simulink model "ABB_1010"  (R2024a)
settings: Solver=VariableStepAuto  StartTime=0.0  StopTime=200  RelTol=1e-3
model workspace: external: MATLAB File C:\Users\lucas\OneDrive\Documents\MATLAB\projeto final\ABB_1010_DataFile.m (data not in the file)
values from neighbouring files (symbols this model uses):
  g = 9.81    [inicializacaoAntropomorfico.m]
  I1 = [ 0.00243841  0.00000307  0.00007261    [inicializacaoAntropomorfico.m]
  I2 = [ 0.01633569  0.00000387 -0.00034405    [inicializacaoAntropomorfico.m]
  I3 = [ 0.00244760 -0.00000208  0.00000538    [inicializacaoAntropomorfico.m]
  I4 = [ 0.00245792 -0.00000008  0.00003121    [inicializacaoAntropomorfico.m]
  I5 = [ 0.00062165 -0.00000206 -0.00000303    [inicializacaoAntropomorfico.m]
  I6 = [ 0.00000357  0.00000000  0.00000000    [inicializacaoAntropomorfico.m]
  I7 = [(m7*L7^2)/12 0.00000000  0.00000000    [inicializacaoAntropomorfico.m]
  L = [L1, L2, L3, L4, L5, L6, L7]    [inicializacaoAntropomorfico.m]
  Lcm1 = [-0.00258308  0.00024508 -0.01434968]    [inicializacaoAntropomorfico.m]
  Lcm2 = [-0.02078894  0.00020016 -0.10516734]    [inicializacaoAntropomorfico.m]
  Lcm3 = [ 0.00021912  0.00015355 -0.06228290]    [inicializacaoAntropomorfico.m]
  Lcm4 = [-0.00172658 -0.00124140 -0.07369196]    [inicializacaoAntropomorfico.m]
  Lcm5 = [-0.00014110  0.00085992 -0.03825278]    [inicializacaoAntropomorfico.m]
  Lcm6 = [ 0.00002478  0.00000000 -0.00042157]    [inicializacaoAntropomorfico.m]
  Lcm7 = [ 0           0          -0.05000000]    [inicializacaoAntropomorfico.m]
  m = [m1, m2, m3, m4, m5, m6, m7]    [inicializacaoAntropomorfico.m]
  Pf = [  0.05    [inicializacaoAntropomorfico.m]
  Pi = [  0.2    [inicializacaoAntropomorfico.m]
  Raio = [0]    [inicializacaoAntropomorfico.m]
  Sentido = [0]    [inicializacaoAntropomorfico.m]
  Tipo = [1]    [inicializacaoAntropomorfico.m]
undefined symbols (not defined in the file or in its folder): smiData, X, Y, Z
libraries: sm_lib x35, nesl_utility x7
(part 14 of 16)

== matlab function ABB_1010/Dinamica1/MATLAB Function3 ==
  data: L parameter; Lcm1 parameter; Q input; I2 parameter; I3 parameter; I4 parameter; I5 parameter; I6 parameter; I7 parameter; Lcm2 parameter; Lcm3 parameter; Lcm4 parameter; Lcm5 parameter; Lcm6 parameter; m parameter; dQ input; C output; Lcm7 parameter; I1 parameter
function C = func_C( L, Lcm1, Q, I2, I3, I4, I5, I6, I7, Lcm2, Lcm3, Lcm4, Lcm5, Lcm6, m, dQ, Lcm7, I1)
%func_C
%    OUT1 = func_C(Ixx2,Ixx3,Ixx4,Ixx5,Ixx6,Ixy3,Ixy4,Ixy5,Ixy6,Ixz2,Ixz3,Ixz4,Ixz5,Ixz6,Iyx3,Iyx4,Iyx5,Iyx6,Iyy4,Iyy5,Iyy6,Iyz3,Iyz4,Iyz5,Iyz6,Izx2,Izx3,Izx4,Izx5,Izx6,Izy3,Izy4,Izy5,Izy6,Izz2,Izz3,Izz4,Izz5,Izz6,Lx2,Lx3,Lxcm2,Lxcm3,Lxcm4,Lxcm5,Lxcm6,Lycm3,Lycm4,Lycm5,Lycm6,Lz4,Lz5,Lzcm2,Lzcm3,Lzcm4,Lzcm5,Lzcm6,Q2,Q3,Q4,Q5,Q6,dQ1,dQ2,dQ3,dQ4,dQ5,dQ6,M2,M3,M4,M5,M6)

%    This function was generated by the Symbolic Math Toolbox version 24.1.
%    30-Apr-2025 06:24:11

C   = zeros(6,1);
m1  = m(1);
m2  = m(2);
m3  = m(3);
m4  = m(4);
m5  = m(5);
m6  = m(6);
m7  = m(7);

Q1  = Q(1);
Q2  = Q(2);
Q3  = Q(3);
Q4  = Q(4);
Q5  = Q(5);
Q6  = Q(6);

dQ1  = dQ(1);
dQ2  = dQ(2);
dQ3  = dQ(3);
dQ4  = dQ(4);
dQ5  = dQ(5);
dQ6  = dQ(6);

Lz1 = L(1);
Lx2 = L(2);
Lx3 = L(3);
Lx4 = L(4);
Lz5 = L(5);
Lz6 = L(6);
Lz7 = L(7);

Lxcm1 = Lcm1(1);
Lycm1 = Lcm1(2);
Lzcm1 = Lcm1(3);

Lxcm2 = Lcm2(1);
Lycm2 = Lcm2(2);
Lzcm2 = Lcm2(3);

Lxcm3 = Lcm3(1);
Lycm3 = Lcm3(2);
Lzcm3 = Lcm3(3);

Lxcm4 = Lcm4(1);
Lycm4 = Lcm4(2);
Lzcm4 = Lcm4(3);

Lxcm5 = Lcm5(1);
Lycm5 = Lcm5(2);
Lzcm5 = Lcm5(3);

Lxcm6 = Lcm6(1);
Lycm6 = Lcm6(2);
Lzcm6 = Lcm6(3);

Lxcm7 = Lcm7(1);
Lycm7 = Lcm7(2);
Lzcm7 = Lcm7(3);

Ixx1 = I1(1,1);
Ixy1 = I1(1,2);
Ixz1 = I1(1,3);
Iyx1 = I1(2,1);
Iyy1 = I1(2,2);
Iyz1 = I1(2,3);
Izx1 = I1(3,1);
Izy1 = I1(3,2);
Izz1 = I1(3,3);

Ixx2 = I2(1,1);
Ixy2 = I2(1,2);
Ixz2 = I2(1,3);
Iyx2 = I2(2,1);
Iyy2 = I2(2,2);
Iyz2 = I2(2,3);
Izx2 = I2(3,1);
Izy2 = I2(3,2);
Izz2 = I2(3,3);

Ixx3 = I3(1,1);
Ixy3 = I3(1,2);
Ixz3 = I3(1,3);
Iyx3 = I3(2,1);
Iyy3 = I3(2,2);
Iyz3 = I3(2,3);
Izx3 = I3(3,1);
Izy3 = I3(3,2);
Izz3 = I3(3,3);

Ixx4 = I4(1,1);
Ixy4 = I4(1,2);
Ixz4 = I4(1,3);
Iyx4 = I4(2,1);
Iyy4 = I4(2,2);
Iyz4 = I4(2,3);
Izx4 = I4(3,1);
Izy4 = I4(3,2);
Izz4 = I4(3,3);

Ixx5 = I5(1,1);
Ixy5 = I5(1,2);
Ixz5 = I5(1,3);
Iyx5 = I5(2,1);
Iyy5 = I5(2,2);
Iyz5 = I5(2,3);
Izx5 = I5(3,1);
Izy5 = I5(3,2);
Izz5 = I5(3,3);

Ixx6 = I6(1,1);
Ixy6 = I6(1,2);
Ixz6 = I6(1,3);
Iyx6 = I6(2,1);
Iyy6 = I6(2,2);
Iyz6 = I6(2,3);
Izx6 = I6(3,1);
Izy6 = I6(3,2);
Izz6 = I6(3,3);

Ixx7 = I7(1,1);
Ixy7 = I7(1,2);
Ixz7 = I7(1,3);
Iyx7 = I7(2,1);
Iyy7 = I7(2,2);
Iyz7 = I7(2,3);
Izx7 = I7(3,1);
Izy7 = I7(3,2);
Izz7 = I7(3,3);

t2 = cos(Q2);
t3 = cos(Q3);
t4 = cos(Q4);
t5 = cos(Q5);
t6 = cos(Q6);
t7 = sin(Q2);
t8 = sin(Q3);
t9 = sin(Q4);
t10 = sin(Q5);
t11 = sin(Q6);
t12 = Lx2^2;
t13 = Lx3^2;
t14 = Lx4^2;
t15 = Lxcm3^2;
t16 = Lxcm4^2;
t17 = Lxcm5^2;
t18 = Lxcm6^2;
t19 = Lycm4^2;
t20 = Lycm5^2;
t21 = Lycm6^2;
t22 = Lz6^2;
t23 = Lzcm3^2;
t24 = Lzcm4^2;
t25 = Lzcm5^2;
t26 = Lzcm6^2;
t27 = Q2*2.0;
t28 = Q3*2.0;
t29 = Q4*2.0;
t30 = Q5*2.0;
t31 = Q6*2.0;
t48 = Lx4*Lycm4*dQ2*dQ4*m4*2.0;
t49 = Lx4*Lycm4*dQ3*dQ4*m4*2.0;
t50 = Lx4*Lycm5*dQ2*dQ4*m5*2.0;
t51 = Lx4*Lycm5*dQ3*dQ4*m5*2.0;
t52 = Lxcm4*Lycm4*dQ2*dQ4*m4*2.0;
t53 = Lxcm4*Lycm4*dQ3*dQ4*m4*2.0;
t54 = Lxcm5*Lzcm5*dQ2*dQ5*m5*2.0;
t55 = Lxcm5*Lzcm5*dQ3*dQ5*m5*2.0;
t32 = t2^2;
t33 = t3^2;
t34 = t4^2;
t35 = t5^2;
t36 = t6^2;
t37 = sin(t27);
t38 = sin(t28);
t39 = sin(t29);
t40 = sin(t30);
t41 = sin(t31);
t42 = Ixx5*dQ4*dQ5*t9;
t43 = Ixx6*dQ4*dQ5*t9;
t44 = Iyy5*dQ4*dQ5*t9;
t45 = Iyy6*dQ4*dQ5*t9;
t46 = Izz5*dQ4*dQ5*t9;
t47 = Izz6*dQ4*dQ5*t9;
t80 = Ixx4*dQ1*dQ4*t2*t8;
t81 = Ixx4*dQ1*dQ4*t3*t7;
t82 = Ixx5*dQ1*dQ4*t2*t8;
t83 = Ixx5*dQ1*dQ4*t3*t7;
t84 = Ixx6*dQ1*dQ4*t2*t8;
t85 = Ixx6*dQ1*dQ4*t3*t7;
t86 = Ixx6*dQ4*dQ6*t4*t10;
t87 = Ixx6*dQ5*dQ6*t5*t9;
t88 = Iyy4*dQ1*dQ4*t2*t8;
t89 = Iyy4*dQ1*dQ4*t3*t7;
t90 = Iyy5*dQ1*dQ4*t2*t8;
t91 = Iyy5*dQ1*dQ4*t3*t7;
t92 = Iyy6*dQ1*dQ4*t2*t8;
t93 = Iyy6*dQ1*dQ4*t3*t7;
t94 = Iyy6*dQ4*dQ6*t4*t10;
t95 = Iyy6*dQ5*dQ6*t5*t9;
t96 = Izz4*dQ1*dQ4*t2*t8;
t97 = Izz4*dQ1*dQ4*t3*t7;
t98 = Izz5*dQ1*dQ4*t2*t8;
t99 = Izz5*dQ1*dQ4*t3*t7;
t100 = Izz6*dQ1*dQ4*t2*t8;
t101 = Izz6*dQ1*dQ4*t3*t7;
t102 = Izz6*dQ4*dQ6*t4*t10;
t103 = Izz6*dQ5*dQ6*t5*t9;
t104 = Lx3*Lycm4*dQ2*dQ4*m4*t4*2.0;
t105 = Lx3*Lycm4*dQ3*dQ4*m4*t4*2.0;
t106 = Lx3*Lycm5*dQ2*dQ4*m5*t4*2.0;
t107 = Lx3*Lycm5*dQ3*dQ4*m5*t4*2.0;
t108 = Lx4*Lycm6*dQ2*dQ4*m6*t6*2.0;
t109 = Lx4*Lycm6*dQ3*dQ4*m6*t6*2.0;
t110 = Lxcm5*Lycm5*dQ2*dQ4*m5*t5*2.0;
t111 = Lxcm5*Lycm5*dQ3*dQ4*m5*t5*2.0;
t112 = Lxcm6*Lycm6*dQ2*dQ4*m6*t5*2.0;
t113 = Lxcm6*Lycm6*dQ3*dQ4*m6*t5*2.0;
t114 = Lxcm6*Lycm6*dQ5*dQ6*m6*t4*2.0;
t115 = Lxcm6*Lz6*dQ2*dQ5*m6*t6*2.0;
t116 = Lxcm6*Lz6*dQ3*dQ5*m6*t6*2.0;
t117 = Lxcm6*Lzcm6*dQ2*dQ5*m6*t6*2.0;
t118 = Lxcm6*Lzcm6*dQ3*dQ5*m6*t6*2.0;
t119 = Lx3*Lx4*dQ2*dQ4*m4*t9*2.0;
t120 = Lx3*Lx4*dQ2*dQ4*m5*t9*2.0;
t121 = Lx3*Lx4*dQ3*dQ4*m4*t9*2.0;
t122 = Lx3*Lx4*dQ2*dQ4*m6*t9*2.0;
t123 = Lx3*Lx4*dQ3*dQ4*m5*t9*2.0;
t124 = Lx3*Lx4*dQ3*dQ4*m6*t9*2.0;
t125 = Lx3*Lxcm4*dQ2*dQ4*m4*t9*2.0;
t126 = Lx3*Lxcm4*dQ3*dQ4*m4*t9*2.0;
t127 = Lx4*Lxcm6*dQ2*dQ4*m6*t11*2.0;
t128 = Lx4*Lxcm6*dQ3*dQ4*m6*t11*2.0;
t129 = Lycm6*Lz6*dQ2*dQ5*m6*t11*2.0;
t130 = Lycm6*Lz6*dQ3*dQ5*m6*t11*2.0;
t131 = Lycm5*Lzcm5*dQ2*dQ4*m5*t10*2.0;
t132 = Lycm5*Lzcm5*dQ3*dQ4*m5*t10*2.0;
t133 = Lycm6*Lzcm6*dQ2*dQ5*m6*t11*2.0;
t134 = Lycm6*Lzcm6*dQ3*dQ5*m6*t11*2.0;
t135 = dQ4*dQ5*m5*t9*t17*2.0;
t136 = dQ4*dQ5*m6*t9*t21*2.0;
t147 = Ixx5*dQ1*dQ5*t2*t3*t9;
t148 = Ixx6*dQ1*dQ5*t2*t3*t9;
t149 = Ixx6*dQ1*dQ6*t2*t5*t8;
t150 = Ixx6*dQ1*dQ6*t3*t5*t7;
t151 = Iyy5*dQ1*dQ5*t2*t3*t9;
t152 = Iyy6*dQ1*dQ5*t2*t3*t9;
t153 = Iyy6*dQ1*dQ6*t2*t5*t8;
t154 = Iyy6*dQ1*dQ6*t3*t5*t7;
t155 = Izz5*dQ1*dQ5*t2*t3*t9;
t156 = Izz6*dQ1*dQ5*t2*t3*t9;
t157 = Izz6*dQ1*dQ6*t2*t5*t8;
t158 = Izz6*dQ1*dQ6*t3*t5*t7;
t159 = Ixx5*dQ1*dQ5*t7*t8*t9;
t160 = Ixx6*dQ1*dQ5*t7*t8*t9;
t161 = Iyy5*dQ1*dQ5*t7*t8*t9;
t162 = Iyy6*dQ1*dQ5*t7*t8*t9;
t163 = Izz5*dQ1*dQ5*t7*t8*t9;
t164 = Izz6*dQ1*dQ5*t7*t8*t9;
t249 = Lx3*Lycm6*dQ2*dQ4*m6*t4*t6*2.0;
t250 = Lx3*Lycm6*dQ3*dQ4*m6*t4*t6*2.0;
t251 = Lx3*Lycm6*dQ5*dQ6*m6*t5*t6*2.0;
t252 = Lx3*Lz6*dQ2*dQ5*m6*t4*t5*2.0;
t253 = Lx3*Lz6*dQ3*dQ5*m6*t4*t5*2.0;
t254 = Lx3*Lzcm5*dQ2*dQ5*m5*t4*t5*2.0;
t255 = Lx3*Lzcm5*dQ3*dQ5*m5*t4*t5*2.0;
t256 = Lx3*Lzcm6*dQ2*dQ5*m6*t4*t5*2.0;
t257 = Lx3*Lzcm6*dQ3*dQ5*m6*t4*t5*2.0;
t258 = Ixx6*dQ2*dQ6*t4*t5*t9*2.0;
t259 = Ixx6*dQ3*dQ6*t4*t5*t9*2.0;
t260 = Ixx6*dQ2*dQ4*t5*t6*t11*2.0;
t261 = Ixx6*dQ3*dQ4*t5*t6*t11*2.0;
t262 = Ixx6*dQ5*dQ6*t4*t6*t11*2.0;
t263 = Iyy6*dQ2*dQ6*t4*t5*t9*2.0;
t264 = Iyy6*dQ3*dQ6*t4*t5*t9*2.0;
t265 = Iyy6*dQ2*dQ4*t5*t6*t11*2.0;
t266 = Iyy6*dQ3*dQ4*t5*t6*t11*2.0;
t267 = Iyy6*dQ5*dQ6*t4*t6*t11*2.0;
t268 = Lx3*Lxcm5*dQ2*dQ4*m5*t5*t9*2.0;
t269 = Lx3*Lxcm5*dQ2*dQ5*m5*t4*t10*2.0;
t270 = Lx3*Lxcm5*dQ3*dQ4*m5*t5*t9*2.0;
t271 = Lx3*Lxcm5*dQ3*dQ5*m5*t4*t10*2.0;
t272 = Lx3*Lxcm6*dQ2*dQ4*m6*t4*t11*2.0;
t273 = Lx3*Lxcm6*dQ3*dQ4*m6*t4*t11*2.0;
t274 = Lx3*Lxcm6*dQ2*dQ6*m6*t6*t9*2.0;
t275 = Lx3*Lxcm6*dQ3*dQ6*m6*t6*t9*2.0;
t276 = Lx3*Lxcm6*dQ5*dQ6*m6*t5*t11*2.0;
t277 = Lycm6*Lz6*dQ2*dQ4*m6*t6*t10*2.0;
t278 = Lycm6*Lz6*dQ3*dQ4*m6*t6*t10*2.0;
t279 = Lycm6*Lzcm6*dQ2*dQ4*m6*t6*t10*2.0;
t280 = Lycm6*Lzcm6*dQ3*dQ4*m6*t6*t10*2.0;
t281 = Lx3*Lycm6*dQ2*dQ6*m6*t9*t11*2.0;
t282 = Lx3*Lycm6*dQ3*dQ6*m6*t9*t11*2.0;
t283 = Lx3*Lz6*dQ2*dQ4*m6*t9*t10*2.0;
t284 = Lx3*Lz6*dQ3*dQ4*m6*t9*t10*2.0;
t285 = Lx3*Lzcm5*dQ2*dQ4*m5*t9*t10*2.0;
t286 = Lx3*Lzcm5*dQ3*dQ4*m5*t9*t10*2.0;
t287 = Lx3*Lzcm6*dQ2*dQ4*m6*t9*t10*2.0;
t288 = Lx3*Lzcm6*dQ3*dQ4*m6*t9*t10*2.0;
t289 = Lxcm6*Lz6*dQ2*dQ4*m6*t10*t11*2.0;
t290 = Lxcm6*Lz6*dQ3*dQ4*m6*t10*t11*2.0;
t291 = Lxcm6*Lzcm6*dQ2*dQ4*m6*t10*t11*2.0;
t292 = Lxcm6*Lzcm6*dQ3*dQ4*m6*t10*t11*2.0;
t314 = Ixx6*dQ1*dQ6*t2*t3*t4*t10;
t315 = Iyy6*dQ1*dQ6*t2*t3*t4*t10;
t316 = Izz6*dQ1*dQ6*t2*t3*t4*t10;
t317 = Ixx6*dQ1*dQ6*t4*t7*t8*t10;
t318 = Iyy6*dQ1*dQ6*t4*t7*t8*t10;
t319 = Izz6*dQ1*dQ6*t4*t7*t8*t10;
t349 = dQ1*dQ4*m6*t2*t8*t18*2.0;
t350 = dQ1*dQ4*m6*t3*t7*t18*2.0;
t351 = dQ5*dQ6*m6*t5*t9*t18*2.0;
t352 = dQ1*dQ4*m4*t2*t8*t19*2.0;
t353 = dQ1*dQ4*m4*t3*t7*t19*2.0;
t354 = dQ1*dQ4*m5*t2*t8*t20*2.0;
t355 = dQ1*dQ4*m5*t3*t7*t20*2.0;
t356 = dQ4*dQ6*m6*t4*t10*t21*2.0;
t374 = Lx3*Lycm6*dQ2*dQ6*m6*t4*t5*t6*2.0;
t375 = Lx3*Lycm6*dQ3*dQ6*m6*t4*t5*t6*2.0;
t376 = Lx4*Lycm6*dQ5*dQ6*m6*t4*t5*t6*2.0;
t377 = Lx4*Lzcm4*dQ1*dQ4*m4*t2*t3*t4*2.0;
t378 = Lxcm6*Lz6*dQ4*dQ6*m6*t4*t5*t6*2.0;
t379 = Lxcm4*Lzcm4*dQ1*dQ4*m4*t2*t3*t4*2.0;
t380 = Lxcm5*Lzcm5*dQ1*dQ4*m5*t2*t3*t4*2.0;
t381 = Lxcm6*Lzcm6*dQ4*dQ6*m6*t4*t5*t6*2.0;
t382 = Lx3*Lx4*dQ1*dQ4*m4*t2*t4*t8*2.0;
t383 = Lx3*Lx4*dQ1*dQ4*m4*t3*t4*t7*2.0;
t384 = Lx3*Lx4*dQ1*dQ4*m5*t2*t4*t8*2.0;
t385 = Lx3*Lx4*dQ1*dQ4*m5*t3*t4*t7*2.0;
t386 = Lx3*Lx4*dQ1*dQ4*m6*t2*t4*t8*2.0;
t387 = Lx3*Lx4*dQ1*dQ4*m6*t3*t4*t7*2.0;
t388 = Lx3*Lxcm4*dQ1*dQ4*m4*t2*t4*t8*2.0;
t389 = Lx3*Lxcm4*dQ1*dQ4*m4*t3*t4*t7*2.0;
t390 = Lx4*Lxcm5*dQ2*dQ4*m5*t4*t5*t9*4.0;
t391 = Lx3*Lxcm6*dQ2*dQ4*m6*t5*t6*t9*2.0;
t392 = Lx4*Lxcm5*dQ3*dQ4*m5*t4*t5*t9*4.0;
t393 = Lx3*Lxcm6*dQ2*dQ5*m6*t4*t6*t10*2.0;
t394 = Lx3*Lxcm6*dQ3*dQ4*m6*t5*t6*t9*2.0;
t395 = Lx3*Lxcm6*dQ2*dQ6*m6*t4*t5*t11*2.0;
t396 = Lx3*Lxcm6*dQ3*dQ5*m6*t4*t6*t10*2.0;
t397 = Lx4*Lxcm6*dQ2*dQ6*m6*t4*t6*t9*2.0;
t398 = Lx3*Lxcm6*dQ3*dQ6*m6*t4*t5*t11*2.0;
t399 = Lx4*Lxcm6*dQ3*dQ6*m6*t4*t6*t9*2.0;
t400 = Lx4*Lxcm6*dQ5*dQ6*m6*t4*t5*t11*2.0;
t401 = Lycm6*Lz6*dQ2*dQ6*m6*t5*t6*t10*2.0;
t402 = Lycm6*Lz6*dQ3*dQ6*m6*t5*t6*t10*2.0;
t403 = Lycm6*Lz6*dQ4*dQ6*m6*t4*t5*t11*2.0;
t404 = Lycm4*Lzcm4*dQ1*dQ4*m4*t2*t3*t9*2.0;
t405 = Lycm5*Lzcm5*dQ1*dQ5*m5*t2*t5*t8*2.0;
t406 = Lycm5*Lzcm5*dQ1*dQ5*m5*t3*t5*t7*2.0;
t407 = Lycm5*Lzcm5*dQ2*dQ5*m5*t4*t5*t9*2.0;
t408 = Lycm5*Lzcm5*dQ3*dQ5*m5*t4*t5*t9*2.0;
t409 = Lycm6*Lzcm6*dQ2*dQ6*m6*t5*t6*t10*2.0;
t410 = Lycm6*Lzcm6*dQ3*dQ6*m6*t5*t6*t10*2.0;
t411 = Lycm6*Lzcm6*dQ4*dQ6*m6*t4*t5*t11*2.0;
t432 = Lx3*Lycm4*dQ1*dQ4*m4*t2*t8*t9*2.0;
t433 = Lx3*Lycm4*dQ1*dQ4*m4*t3*t7*t9*2.0;
t434 = Lx3*Lycm5*dQ1*dQ4*m5*t2*t8*t9*2.0;
t435 = Lx3*Lycm5*dQ1*dQ4*m5*t3*t7*t9*2.0;
t436 = Lx3*Lycm6*dQ2*dQ4*m6*t5*t9*t11*2.0;
t437 = Lx3*Lycm6*dQ2*dQ5*m6*t4*t10*t11*2.0;
t438 = Lx3*Lycm6*dQ3*dQ4*m6*t5*t9*t11*2.0;
t439 = Lx3*Lycm6*dQ3*dQ5*m6*t4*t10*t11*2.0;
t440 = Lx4*Lycm6*dQ2*dQ6*m6*t4*t9*t11*2.0;
t441 = Lx4*Lycm6*dQ3*dQ6*m6*t4*t9*t11*2.0;
t442 = Lxcm5*Lycm5*dQ1*dQ5*m5*t2*t8*t10*2.0;
t443 = Lxcm5*Lycm5*dQ1*dQ5*m5*t3*t7*t10*2.0;
t444 = Lxcm6*Lycm6*dQ1*dQ5*m6*t2*t8*t10*2.0;
t445 = Lxcm6*Lycm6*dQ1*dQ5*m6*t3*t7*t10*2.0;
t446 = Lxcm5*Lycm5*dQ2*dQ5*m5*t4*t9*t10*2.0;
t447 = Lxcm5*Lycm5*dQ3*dQ5*m5*t4*t9*t10*2.0;
t448 = Lxcm6*Lycm6*dQ2*dQ5*m6*t4*t9*t10*2.0;
t449 = Lxcm6*Lycm6*dQ3*dQ5*m6*t4*t9*t10*2.0;
t450 = Lxcm6*Lycm6*dQ4*dQ6*m6*t5*t9*t10*2.0;
t451 = Lxcm6*Lycm6*dQ4*dQ5*m6*t6*t9*t11*4.0;
t452 = Lx4*Lz6*dQ2*dQ4*m6*t4*t9*t10*4.0;
t453 = Lx4*Lz6*dQ3*dQ4*m6*t4*t9*t10*4.0;
t454 = Lx4*Lzcm4*dQ1*dQ4*m4*t4*t7*t8*2.0;
t455 = Lx4*Lzcm5*dQ2*dQ4*m5*t4*t9*t10*4.0;
t456 = Lx4*Lzcm5*dQ3*dQ4*m5*t4*t9*t10*4.0;
t457 = Lx4*Lzcm6*dQ2*dQ4*m6*t4*t9*t10*4.0;
t458 = Lx4*Lzcm6*dQ3*dQ4*m6*t4*t9*t10*4.0;
t459 = Lxcm6*Lz6*dQ2*dQ6*m6*t5*t10*t11*2.0;
t460 = Lxcm6*Lz6*dQ3*dQ6*m6*t5*t10*t11*2.0;
t461 = Lxcm4*Lzcm4*dQ1*dQ4*m4*t4*t7*t8*2.0;
t462 = Lxcm5*Lzcm5*dQ1*dQ4*m5*t4*t7*t8*2.0;
t463 = Lxcm5*Lzcm5*dQ4*dQ5*m5*t5*t9*t10*4.0;
t464 = Lxcm6*Lzcm6*dQ2*dQ6*m6*t5*t10*t11*2.0;
t465 = Lxcm6*Lzcm6*dQ3*dQ6*m6*t5*t10*t11*2.0;
t466 = Lycm4*Lzcm4*dQ1*dQ4*m4*t7*t8*t9*2.0;
t594 = dQ1*dQ5*m5*t2*t3*t9*t17*2.0;
t595 = dQ1*dQ6*m6*t2*t5*t8*t18*2.0;
t596 = dQ1*dQ6*m6*t3*t5*t7*t18*2.0;
t597 = dQ2*dQ6*m6*t4*t5*t9*t18*2.0;
t598 = dQ3*dQ6*m6*t4*t5*t9*t18*2.0;
t599 = dQ2*dQ4*m6*t5*t6*t11*t18*2.0;
t600 = dQ3*dQ4*m6*t5*t6*t11*t18*2.0;
t601 = dQ5*dQ6*m6*t4*t6*t11*t18*2.0;
t602 = dQ1*dQ5*m6*t2*t3*t9*t21*2.0;
t603 = dQ2*dQ6*m6*t4*t5*t9*t21*2.0;
t604 = dQ3*dQ6*m6*t4*t5*t9*t21*2.0;
t605 = dQ2*dQ4*m6*t5*t6*t11*t21*2.0;
t606 = dQ3*dQ4*m6*t5*t6*t11*t21*2.0;
t607 = dQ5*dQ6*m6*t4*t6*t11*t21*2.0;
t611 = dQ1*dQ5*m5*t7*t8*t9*t17*2.0;
t612 = dQ1*dQ5*m6*t7*t8*t9*t21*2.0;
t652 = Ixx5*dQ1*dQ4*t2*t3*t4*t5*t10*2.0;
t653 = Iyy6*dQ1*dQ4*t2*t3*t4*t5*t10*2.0;
t654 = Izz5*dQ1*dQ4*t2*t3*t4*t5*t10*2.0;
t655 = Izz6*dQ1*dQ4*t2*t3*t4*t5*t10*2.0;
t656 = Lx3*Lxcm5*dQ1*dQ4*m5*t2*t4*t5*t8*2.0;
t657 = Lx3*Lxcm5*dQ1*dQ4*m5*t3*t4*t5*t7*2.0;
t658 = Lx4*Lxcm5*dQ1*dQ4*m5*t2*t3*t4*t10*2.0;
t659 = Lx3*Lxcm6*dQ1*dQ6*m6*t2*t4*t6*t8*2.0;
t660 = Lx3*Lxcm6*dQ1*dQ6*m6*t3*t4*t6*t7*2.0;
t661 = Lx4*Lxcm6*dQ2*dQ4*m6*t4*t5*t6*t9*4.0;
t662 = Lx4*Lxcm6*dQ3*dQ4*m6*t4*t5*t6*t9*4.0;
t663 = Lycm6*Lz6*dQ1*dQ4*m6*t2*t3*t4*t11*2.0;
t664 = Lycm6*Lz6*dQ1*dQ5*m6*t2*t5*t6*t8*2.0;
t665 = Lycm6*Lz6*dQ1*dQ5*m6*t3*t5*t6*t7*2.0;
t666 = Lycm6*Lz6*dQ2*dQ5*m6*t4*t5*t6*t9*2.0;
t667 = Lycm6*Lz6*dQ3*dQ5*m6*t4*t5*t6*t9*2.0;
t668 = Lycm5*Lzcm5*dQ1*dQ4*m5*t2*t3*t5*t9*2.0;
t669 = Lycm6*Lzcm6*dQ1*dQ4*m6*t2*t3*t4*t11*2.0;
t670 = Lycm6*Lzcm6*dQ1*dQ5*m6*t2*t5*t6*t8*2.0;
t671 = Lycm6*Lzcm6*dQ1*dQ5*m6*t3*t5*t6*t7*2.0;
t672 = Lycm6*Lzcm6*dQ2*dQ5*m6*t4*t5*t6*t9*2.0;
t673 = Lycm6*Lzcm6*dQ3*dQ5*m6*t4*t5*t6*t9*2.0;
t678 = Lx4*Lycm4*dQ1*dQ4*m4*t2*t4*t8*t9*4.0;
t679 = Lx4*Lycm4*dQ1*dQ4*m4*t3*t4*t7*t9*4.0;
t680 = Lx4*Lycm5*dQ1*dQ4*m5*t2*t4*t8*t9*4.0;
t681 = Lx4*Lycm5*dQ1*dQ4*m5*t3*t4*t7*t9*4.0;
t682 = Lx3*Lycm6*dQ1*dQ4*m6*t2*t6*t8*t9*2.0;
t683 = Lx3*Lycm6*dQ1*dQ4*m6*t3*t6*t7*t9*2.0;
t684 = Lx3*Lycm6*dQ1*dQ6*m6*t2*t4*t8*t11*2.0;
t685 = Lx3*Lycm6*dQ1*dQ6*m6*t3*t4*t7*t11*2.0;
t686 = Lx4*Lycm6*dQ2*dQ4*m6*t4*t5*t9*t11*4.0;
t687 = Lx4*Lycm6*dQ3*dQ4*m6*t4*t5*t9*t11*4.0;
t688 = Lxcm4*Lycm4*dQ1*dQ4*m4*t2*t4*t8*t9*4.0;
t689 = Lxcm4*Lycm4*dQ1*dQ4*m4*t3*t4*t7*t9*4.0;
t690 = Lxcm5*Lycm5*dQ1*dQ4*m5*t2*t3*t9*t10*2.0;
t691 = Lxcm6*Lycm6*dQ1*dQ4*m6*t2*t3*t9*t10*2.0;
t692 = Lxcm6*Lycm6*dQ1*dQ6*m6*t2*t4*t8*t9*2.0;
t693 = Lxcm6*Lycm6*dQ1*dQ6*m6*t3*t4*t7*t9*2.0;
t694 = Lxcm6*Lycm6*dQ1*dQ4*m6*t2*t6*t8*t11*4.0;
t695 = Lxcm6*Lycm6*dQ1*dQ4*m6*t3*t6*t7*t11*4.0;
t696 = Lxcm6*Lycm6*dQ2*dQ4*m6*t4*t6*t9*t11*4.0;
t697 = Lxcm6*Lycm6*dQ3*dQ4*m6*t4*t6*t9*t11*4.0;
t698 = Lxcm6*Lycm6*dQ2*dQ5*m6*t5*t6*t10*t11*4.0;
t699 = Lxcm6*Lycm6*dQ3*dQ5*m6*t5*t6*t10*t11*4.0;
t700 = Lxcm6*Lycm6*dQ4*dQ6*m6*t4*t6*t10*t11*4.0;
t701 = Lxcm6*Lycm6*dQ5*dQ6*m6*t5*t6*t9*t11*4.0;
t702 = Lx3*Lz6*dQ1*dQ4*m6*t2*t4*t8*t10*2.0;
t703 = Lx3*Lz6*dQ1*dQ4*m6*t3*t4*t7*t10*2.0;
t704 = Lx3*Lz6*dQ1*dQ5*m6*t2*t5*t8*t9*2.0;
t705 = Lx3*Lz6*dQ1*dQ5*m6*t3*t5*t7*t9*2.0;
t706 = Lx4*Lz6*dQ1*dQ4*m6*t4*t5*t7*t8*2.0;
t707 = Lx3*Lzcm5*dQ1*dQ4*m5*t2*t4*t8*t10*2.0;
t708 = Lx3*Lzcm5*dQ1*dQ4*m5*t3*t4*t7*t10*2.0;
t709 = Lx3*Lzcm5*dQ1*dQ5*m5*t2*t5*t8*t9*2.0;
t710 = Lx3*Lzcm5*dQ1*dQ5*m5*t3*t5*t7*t9*2.0;
t711 = Lx4*Lzcm5*dQ1*dQ4*m5*t4*t5*t7*t8*2.0;
t712 = Lx3*Lzcm6*dQ1*dQ4*m6*t2*t4*t8*t10*2.0;
t713 = Lx3*Lzcm6*dQ1*dQ4*m6*t3*t4*t7*t10*2.0;
t714 = Lx3*Lzcm6*dQ1*dQ5*m6*t2*t5*t8*t9*2.0;
t715 = Lx3*Lzcm6*dQ1*dQ5*m6*t3*t5*t7*t9*2.0;
t716 = Lx4*Lzcm6*dQ1*dQ4*m6*t4*t5*t7*t8*2.0;
t717 = Lxcm6*Lz6*dQ1*dQ4*m6*t4*t6*t7*t8*2.0;
t718 = Lxcm6*Lz6*dQ1*dQ5*m6*t2*t5*t8*t11*2.0;
t719 = Lxcm6*Lz6*dQ1*dQ5*m6*t3*t5*t7*t11*2.0;
t720 = Lxcm6*Lz6*dQ2*dQ5*m6*t4*t5*t9*t11*2.0;
t721 = Lxcm6*Lz6*dQ2*dQ6*m6*t4*t6*t9*t10*2.0;
t722 = Lxcm6*Lz6*dQ3*dQ5*m6*t4*t5*t9*t11*2.0;
t723 = Lxcm6*Lz6*dQ3*dQ6*m6*t4*t6*t9*t10*2.0;
t724 = Lxcm6*Lz6*dQ4*dQ5*m6*t5*t6*t9*t10*4.0;
t725 = Lxcm5*Lzcm5*dQ1*dQ5*m5*t2*t4*t8*t9*2.0;
t726 = Lxcm5*Lzcm5*dQ1*dQ5*m5*t3*t4*t7*t9*2.0;
t727 = Lxcm6*Lzcm6*dQ1*dQ4*m6*t4*t6*t7*t8*2.0;
t728 = Lxcm6*Lzcm6*dQ1*dQ5*m6*t2*t5*t8*t11*2.0;
t729 = Lxcm6*Lzcm6*dQ1*dQ5*m6*t3*t5*t7*t11*2.0;
t730 = Lxcm5*Lzcm5*dQ2*dQ4*m5*t4*t5*t9*t10*4.0;
t731 = Lxcm5*Lzcm5*dQ3*dQ4*m5*t4*t5*t9*t10*4.0;
t732 = Lxcm6*Lzcm6*dQ2*dQ5*m6*t4*t5*t9*t11*2.0;
t733 = Lxcm6*Lzcm6*dQ2*dQ6*m6*t4*t6*t9*t10*2.0;
t734 = Lxcm6*Lzcm6*dQ3*dQ5*m6*t4*t5*t9*t11*2.0;
t735 = Lxcm6*Lzcm6*dQ3*dQ6*m6*t4*t6*t9*t10*2.0;
t736 = Lxcm6*Lzcm6*dQ4*dQ5*m6*t5*t6*t9*t10*4.0;
t737 = Ixx5*dQ1*dQ4*t4*t5*t7*t8*t10*2.0;
t738 = Ixx6*dQ1*dQ5*t2*t6*t8*t10*t11*2.0;
t739 = Ixx6*dQ1*dQ5*t3*t6*t7*t10*t11*2.0;
t740 = Ixx6*dQ2*dQ5*t4*t6*t9*t10*t11*2.0;
t741 = Ixx6*dQ3*dQ5*t4*t6*t9*t10*t11*2.0;
t742 = Ixx6*dQ4*dQ6*t5*t6*t9*t10*t11*2.0;
t743 = Iyy6*dQ1*dQ4*t4*t5*t7*t8*t10*2.0;
t744 = Iyy6*dQ1*dQ5*t2*t6*t8*t10*t11*2.0;
t745 = Iyy6*dQ1*dQ5*t3*t6*t7*t10*t11*2.0;
t746 = Iyy6*dQ2*dQ5*t4*t6*t9*t10*t11*2.0;
t747 = Iyy6*dQ3*dQ5*t4*t6*t9*t10*t11*2.0;
t748 = Iyy6*dQ4*dQ6*t5*t6*t9*t10*t11*2.0;
t749 = Izz5*dQ1*dQ4*t4*t5*t7*t8*t10*2.0;
t750 = Izz6*dQ1*dQ4*t4*t5*t7*t8*t10*2.0;
t751 = Lx3*Lxcm5*dQ1*dQ5*m5*t2*t8*t9*t10*2.0;
t752 = Lx3*Lxcm5*dQ1*dQ5*m5*t3*t7*t9*t10*2.0;
t753 = Lx4*Lxcm5*dQ1*dQ4*m5*t4*t7*t8*t10*2.0;
t754 = Lx3*Lxcm6*dQ1*dQ4*m6*t2*t8*t9*t11*2.0;
t755 = Lx3*Lxcm6*dQ1*dQ4*m6*t3*t7*t9*t11*2.0;
t756 = Lycm6*Lz6*dQ1*dQ4*m6*t4*t7*t8*t11*2.0;
t757 = Lycm6*Lz6*dQ2*dQ6*m6*t4*t9*t10*t11*2.0;
t758 = Lycm6*Lz6*dQ3*dQ6*m6*t4*t9*t10*t11*2.0;
t759 = Lycm6*Lz6*dQ4*dQ5*m6*t5*t9*t10*t11*4.0;
t760 = Lycm5*Lzcm5*dQ1*dQ4*m5*t5*t7*t8*t9*2.0;
t761 = Lycm6*Lzcm6*dQ1*dQ4*m6*t4*t7*t8*t11*2.0;
t762 = Lycm6*Lzcm6*dQ2*dQ6*m6*t4*t9*t10*t11*2.0;
t763 = Lycm6*Lzcm6*dQ3*dQ6*m6*t4*t9*t10*t11*2.0;
t764 = Lycm6*Lzcm6*dQ4*dQ5*m6*t5*t9*t10*t11*4.0;
t765 = Lxcm5*Lycm5*dQ1*dQ4*m5*t7*t8*t9*t10*2.0;
t766 = Lxcm6*Lycm6*dQ1*dQ4*m6*t7*t8*t9*t10*2.0;
t840 = Lx4*Lz6*dQ1*dQ4*m6*t2*t3*t4*t5*2.0;
t841 = Lx4*Lzcm5*dQ1*dQ4*m5*t2*t3*t4*t5*2.0;
t842 = Lx4*Lzcm6*dQ1*dQ4*m6*t2*t3*t4*t5*2.0;
t843 = Lxcm6*Lz6*dQ1*dQ4*m6*t2*t3*t4*t6*2.0;
t844 = Lxcm6*Lzcm6*dQ1*dQ4*m6*t2*t3*t4*t6*2.0;
t891 = dQ1*dQ6*m6*t2*t3*t4*t10*t21*2.0;
t908 = dQ1*dQ6*m6*t4*t7*t8*t10*t21*2.0;
t1080 = Lxcm6*Lz6*dQ1*dQ6*m6*t2*t3*t4*t5*t6*2.0;
t1081 = Lxcm6*Lzcm6*dQ1*dQ6*m6*t2*t3*t4*t5*t6*2.0;
t1082 = Lx3*Lxcm6*dQ1*dQ4*m6*t2*t4*t5*t6*t8*2.0;
t1083 = Lx3*Lxcm6*dQ1*dQ4*m6*t3*t4*t5*t6*t7*2.0;
t1084 = Lx4*Lxcm6*dQ1*dQ4*m6*t2*t3*t4*t6*t10*2.0;
t1085 = Lycm6*Lz6*dQ1*dQ4*m6*t2*t3*t5*t6*t9*2.0;
t1086 = Lycm6*Lz6*dQ1*dQ6*m6*t2*t3*t4*t5*t11*2.0;
t1087 = Lycm6*Lzcm6*dQ1*dQ4*m6*t2*t3*t5*t6*t9*2.0;
t1088 = Lycm6*Lzcm6*dQ1*dQ6*m6*t2*t3*t4*t5*t11*2.0;
t1089 = Lz6*Lzcm6*dQ1*dQ4*m6*t2*t3*t4*t5*t10*4.0;
t1116 = Lx3*Lycm6*dQ1*dQ4*m6*t2*t4*t5*t8*t11*2.0;
t1117 = Lx3*Lycm6*dQ1*dQ4*m6*t3*t4*t5*t7*t11*2.0;
t1118 = Lx4*Lycm6*dQ1*dQ4*m6*t2*t3*t4*t10*t11*2.0;
t1119 = Lx3*Lycm6*dQ1*dQ6*m6*t2*t5*t6*t8*t9*2.0;
t1120 = Lx3*Lycm6*dQ1*dQ6*m6*t3*t5*t6*t7*t9*2.0;
t1121 = Lx4*Lycm6*dQ1*dQ4*m6*t2*t4*t6*t8*t9*4.0;
t1122 = Lx4*Lycm6*dQ1*dQ4*m6*t3*t4*t6*t7*t9*4.0;
t1123 = Lxcm5*Lycm5*dQ1*dQ4*m5*t2*t4*t5*t8*t9*4.0;
t1124 = Lxcm5*Lycm5*dQ1*dQ4*m5*t3*t4*t5*t7*t9*4.0;
t1125 = Lxcm6*Lycm6*dQ1*dQ4*m6*t2*t4*t5*t8*t9*4.0;
t1126 = Lxcm6*Lycm6*dQ1*dQ4*m6*t3*t4*t5*t7*t9*4.0;
t1127 = Lxcm6*Lycm6*dQ1*dQ6*m6*t2*t3*t5*t9*t10*2.0;
t1128 = Lxcm6*Lycm6*dQ1*dQ5*m6*t2*t3*t6*t9*t11*4.0;
t1129 = Lxcm6*Lycm6*dQ1*dQ6*m6*t2*t5*t6*t8*t11*4.0;
t1130 = Lxcm6*Lycm6*dQ1*dQ6*m6*t3*t5*t6*t7*t11*4.0;
t1131 = Lx4*Lz6*dQ1*dQ5*m6*t2*t4*t5*t8*t9*2.0;
t1132 = Lx4*Lz6*dQ1*dQ5*m6*t3*t4*t5*t7*t9*2.0;
t1133 = Lx4*Lzcm5*dQ1*dQ5*m5*t2*t4*t5*t8*t9*2.0;
t1134 = Lx4*Lzcm5*dQ1*dQ5*m5*t3*t4*t5*t7*t9*2.0;
t1135 = Lx4*Lzcm6*dQ1*dQ5*m6*t2*t4*t5*t8*t9*2.0;
t1136 = Lx4*Lzcm6*dQ1*dQ5*m6*t3*t4*t5*t7*t9*2.0;
t1137 = Lxcm6*Lz6*dQ1*dQ4*m6*t2*t3*t5*t9*t11*2.0;
t1138 = Lxcm6*Lz6*dQ1*dQ5*m6*t2*t4*t6*t8*t9*2.0;
t1139 = Lxcm6*Lz6*dQ1*dQ5*m6*t3*t4*t6*t7*t9*2.0;
t1140 = Lxcm6*Lz6*dQ1*dQ6*m6*t4*t5*t6*t7*t8*2.0;
t1141 = Lxcm6*Lz6*dQ2*dQ4*m6*t4*t5*t6*t9*t10*4.0;
t1142 = Lxcm6*Lz6*dQ3*dQ4*m6*t4*t5*t6*t9*t10*4.0;
t1143 = Lxcm5*Lzcm5*dQ1*dQ5*m5*t2*t3*t5*t9*t10*4.0;
t1144 = Lxcm6*Lzcm6*dQ1*dQ4*m6*t2*t3*t5*t9*t11*2.0;
t1145 = Lxcm6*Lzcm6*dQ1*dQ5*m6*t2*t4*t6*t8*t9*2.0;
t1146 = Lxcm6*Lzcm6*dQ1*dQ5*m6*t3*t4*t6*t7*t9*2.0;
t1147 = Lxcm6*Lzcm6*dQ1*dQ6*m6*t4*t5*t6*t7*t8*2.0;
t1148 = Lxcm6*Lzcm6*dQ2*dQ4*m6*t4*t5*t6*t9*t10*4.0;
t1149 = Lxcm6*Lzcm6*dQ3*dQ4*m6*t4*t5*t6*t9*t10*4.0;
t1150 = Ixx5*dQ1*dQ5*t2*t4*t5*t8*t9*t10*2.0;
t1151 = Ixx5*dQ1*dQ5*t3*t4*t5*t7*t9*t10*2.0;
t1152 = Ixx6*dQ1*dQ4*t2*t3*t6*t9*t10*t11*2.0;
t1153 = Ixx6*dQ1*dQ6*t2*t4*t6*t8*t9*t11*2.0;
t1154 = Ixx6*dQ1*dQ6*t3*t4*t6*t7*t9*t11*2.0;
t1155 = Iyy6*dQ1*dQ5*t2*t4*t5*t8*t9*t10*2.0;
t1156 = Iyy6*dQ1*dQ5*t3*t4*t5*t7*t9*t10*2.0;
t1157 = Iyy6*dQ1*dQ4*t2*t3*t6*t9*t10*t11*2.0;
t1158 = Iyy6*dQ1*dQ6*t2*t4*t6*t8*t9*t11*2.0;
t1159 = Iyy6*dQ1*dQ6*t3*t4*t6*t7*t9*t11*2.0;
t1160 = Izz5*dQ1*dQ5*t2*t4*t5*t8*t9*t10*2.0;
t1161 = Izz5*dQ1*dQ5*t3*t4*t5*t7*t9*t10*2.0;
t1162 = Izz6*dQ1*dQ5*t2*t4*t5*t8*t9*t10*2.0;
t1163 = Izz6*dQ1*dQ5*t3*t4*t5*t7*t9*t10*2.0;
t1164 = Lx4*Lxcm5*dQ1*dQ5*m5*t2*t4*t8*t9*t10*2.0;
t1165 = Lx4*Lxcm5*dQ1*dQ5*m5*t3*t4*t7*t9*t10*2.0;
t1166 = Lx3*Lxcm6*dQ1*dQ5*m6*t2*t6*t8*t9*t10*2.0;
t1167 = Lx3*Lxcm6*dQ1*dQ5*m6*t3*t6*t7*t9*t10*2.0;
t1168 = Lx4*Lxcm6*dQ1*dQ4*m6*t4*t6*t7*t8*t10*2.0;
t1169 = Lx3*Lxcm6*dQ1*dQ6*m6*t2*t5*t8*t9*t11*2.0;
t1170 = Lx3*Lxcm6*dQ1*dQ6*m6*t3*t5*t7*t9*t11*2.0;
t1171 = Lx4*Lxcm6*dQ1*dQ4*m6*t2*t4*t8*t9*t11*4.0;
t1172 = Lx4*Lxcm6*dQ1*dQ4*m6*t3*t4*t7*t9*t11*4.0;
t1173 = Lycm6*Lz6*dQ1*dQ4*m6*t5*t6*t7*t8*t9*2.0;
t1174 = Lycm6*Lz6*dQ1*dQ5*m6*t2*t4*t8*t9*t11*2.0;
t1175 = Lycm6*Lz6*dQ1*dQ5*m6*t3*t4*t7*t9*t11*2.0;
t1176 = Lycm6*Lz6*dQ1*dQ6*m6*t4*t5*t7*t8*t11*2.0;
t1177 = Lycm6*Lz6*dQ2*dQ4*m6*t4*t5*t9*t10*t11*4.0;
t1178 = Lycm6*Lz6*dQ3*dQ4*m6*t4*t5*t9*t10*t11*4.0;
t1179 = Lycm5*Lzcm5*dQ1*dQ4*m5*t2*t4*t8*t9*t10*4.0;
t1180 = Lycm5*Lzcm5*dQ1*dQ4*m5*t3*t4*t7*t9*t10*4.0;
t1181 = Lycm6*Lzcm6*dQ1*dQ4*m6*t5*t6*t7*t8*t9*2.0;
t1182 = Lycm6*Lzcm6*dQ1*dQ5*m6*t2*t4*t8*t9*t11*2.0;
t1183 = Lycm6*Lzcm6*dQ1*dQ5*m6*t3*t4*t7*t9*t11*2.0;
t1184 = Lycm6*Lzcm6*dQ1*dQ6*m6*t4*t5*t7*t8*t11*2.0;
t1185 = Lycm6*Lzcm6*dQ2*dQ4*m6*t4*t5*t9*t10*t11*4.0;
t1186 = Lycm6*Lzcm6*dQ3*dQ4*m6*t4*t5*t9*t10*t11*4.0;
t1187 = Lz6*Lzcm6*dQ1*dQ4*m6*t4*t5*t7*t8*t10*4.0;
t1188 = Lx3*Lycm6*dQ1*dQ5*m6*t2*t8*t9*t10*t11*2.0;
t1189 = Lx3*Lycm6*dQ1*dQ5*m6*t3*t7*t9*t10*t11*2.0;
t1190 = Lx4*Lycm6*dQ1*dQ4*m6*t4*t7*t8*t10*t11*2.0;
t1191 = Lxcm6*Lycm6*dQ1*dQ6*m6*t5*t7*t8*t9*t10*2.0;
t1192 = Lxcm6*Lycm6*dQ1*dQ5*m6*t6*t7*t8*t9*t11*4.0;
t1193 = Lxcm6*Lz6*dQ1*dQ4*m6*t5*t7*t8*t9*t11*2.0;
t1194 = Lxcm5*Lzcm5*dQ1*dQ5*m5*t5*t7*t8*t9*t10*4.0;
t1195 = Lxcm6*Lzcm6*dQ1*dQ4*m6*t5*t7*t8*t9*t11*2.0;
t1196 = Ixx6*dQ1*dQ4*t6*t7*t8*t9*t10*t11*2.0;
t1197 = Iyy6*dQ1*dQ4*t6*t7*t8*t9*t10*t11*2.0;
t1278 = Lxcm6*Lycm6*dQ2*dQ6*m6*t4*t5*t6*t9*t11*8.0;
t1279 = Lxcm6*Lycm6*dQ3*dQ6*m6*t4*t5*t6*t9*t11*8.0;
t1288 = dQ1*dQ4*m5*t2*t3*t4*t5*t10*t17*2.0;
t1289 = dQ1*dQ4*m6*t2*t3*t4*t5*t10*t21*2.0;
t1290 = dQ1*dQ4*m6*t2*t3*t4*t5*t10*t22*2.0;
t1291 = dQ1*dQ4*m5*t2*t3*t4*t5*t10*t25*2.0;
t1292 = dQ1*dQ4*m6*t2*t3*t4*t5*t10*t26*2.0;
t1320 = dQ1*dQ4*m5*t4*t5*t7*t8*t10*t17*2.0;
t1321 = dQ1*dQ5*m6*t2*t6*t8*t10*t11*t18*2.0;
t1322 = dQ1*dQ5*m6*t3*t6*t7*t10*t11*t18*2.0;
t1323 = dQ2*dQ5*m6*t4*t6*t9*t10*t11*t18*2.0;
t1324 = dQ3*dQ5*m6*t4*t6*t9*t10*t11*t18*2.0;
t1325 = dQ4*dQ6*m6*t5*t6*t9*t10*t11*t18*2.0;
t1326 = dQ1*dQ4*m6*t4*t5*t7*t8*t10*t21*2.0;
out1 = ft_1({Ixx2,Ixx3,Ixx4,Ixx5,Ixx6,Iyy4,Iyy5,Iyy6,Izz2,Izz3,Izz4,Izz5,Izz6,Lx2,Lx3,Lx4,Lxcm2,Lxcm3,Lxcm4,Lxcm5,Lxcm6,Lycm3,Lycm4,Lycm5,Lycm6,Lz6,Lzcm2,Lzcm3,Lzcm4,Lzcm5,Lzcm6,dQ1,dQ2,dQ3,dQ4,dQ5,dQ6,m2,m3,m4,m5,m6,t10,t100,t101,t102,t103,t104,t105,t106,t107,t108,t1080,t1081,t1082,t1083,t1084,t1085,t1086,t1087,t1088,t1089,t109,t11,t110,t111,t1116,t1117,t1118,t1119,t112,t1120,t1121,t1122,t1123,t1124,t1125,t1126,t1127,t1128,t1129,t113,t1130,t1131,t1132,t1133,t1134,t1135,t1136,t1137,t1138,t1139,t114,t1140,t1141,t1142,t1143,t1144,t1145,t1146,t1147,t1148,t1149,t115,t1150,t1151,t1152,t1153,t1154,t1155,t1156,t1157,t1158,t1159,t116,t1160,t1161,t1162,t1163,t1164,t1165,t1166,t1167,t1168,t1169,t117,t1170,t1171,t1172,t1173,t1174,t1175,t1176,t1177,t1178,t1179,t118,t1180,t1181,t1182,t1183,t1184,t1185,t1186,t1187,t1188,t1189,t119,t1190,t1191,t1192,t1193,t1194,t1195,t1196,t1197,t12,t120,t121,t122,t123,t124,t125,t126,t127,t1278,t1279,t128,t1288,t1289,t129,t1290,t1291,t1292,t13,t130,t131,t132,t1320,t1321,t1322,t1323,t1324,t1325,t1326,t133,t134,t135,t136,t14,t147,t148,t149,t15,t150,t151,t152,t153,t154,t155,t156,t157,t158,t159,t16,t160,t161,t162,t163,t164,t17,t18,t19,t2,t20,t21,t22,t23,t24,t249,t25,t250,t251,t252,t253,t254,t255,t256,t257,t258,t259,t26,t260,t261,t262,t263,t264,t265,t266,t267,t268,t269,t270,t271,t272,t273,t274,t275,t276,t277,t278,t279,t280,t281,t282,t283,t284,t285,t286,t287,t288,t289,t290,t291,t292,t3,t314,t315,t316,t317,t318,t319,t32,t33,t34,t349,t35,t350,t351,t352,t353,t354,t355,t356,t36,t37,t374,t375,t376,t377,t378,t379,t38,t380,t381,t382,t383,t384,t385,t386,t387,t388,t389,t39,t390,t391,t392,t393,t394,t395,t396,t397,t398,t399,t4,t40,t400,t401,t402,t403,t404,t405,t406,t407,t408,t409,t41,t410,t411,t42,t43,t432,t433,t434,t435,t436,t437,t438,t439,t44,t440,t441,t442,t443,t444,t445,t446,t447,t448,t449,t45,t450,t451,t452,t453,t454,t455,t456,t457,t458,t459,t46,t460,t461,t462,t463,t464,t465,t466,t47,t48,t49,t5,t50,t51,t52,t53,t54,t55,t594,t595,t596,t597,t598,t599,t6,t600,t601,t602,t603,t604,t605,t606,t607,t611,t612,t652,t653,t654,t655,t656,t657,t658,t659,t660,t661,t662,t663,t664,t665,t666,t667,t668,t669,t670,t671,t672,t673,t678,t679,t680,t681,t682,t683,t684,t685,t686,t687,t688,t689,t690,t691,t692,t693,t694,t695,t696,t697,t698,t699,t7,t700,t701,t702,t703,t704,t705,t706,t707,t708,t709,t710,t711,t712,t713,t714,t715,t716,t717,t718,t719,t720,t721,t722,t723,t724,t725,t726,t727,t728,t729,t730,t731,t732,t733,t734,t735,t736,t737,t738,t739,t740,t741,t742,t743,t744,t745,t746,t747,t748,t749,t750,t751,t752,t753,t754,t755,t756,t757,t758,t759,t760,t761,t762,t763,t764,t765,t766,t8,t80,t81,t82,t83,t84,t840,t841,t842,t843,t844,t85,t86,t87,t88,t89,t891,t9,t90,t908,t91,t92,t93,t94,t95,t96,t97,t98,t99});
end
function out1 = ft_1(ct)
[Ixx2,Ixx3,Ixx4,Ixx5,Ixx6,Iyy4,Iyy5,Iyy6,Izz2,Izz3,Izz4,Izz5,Izz6,Lx2,Lx3,Lx4,Lxcm2,Lxcm3,Lxcm4,Lxcm5,Lxcm6,Lycm3,Lycm4,Lycm5,Lycm6,Lz6,Lzcm2,Lzcm3,Lzcm4,Lzcm5,Lzcm6,dQ1,dQ2,dQ3,dQ4,dQ5,dQ6,m2,m3,m4,m5,m6,t10,t100,t101,t102,t103,t104,t105,t106,t107,t108,t1080,t1081,t1082,t1083,t1084,t1085,t1086,t1087,t1088,t1089,t109,t11,t110,t111,t1116,t1117,t1118,t1119,t112,t1120,t1121,t1122,t1123,t1124,t1125,t1126,t1127,t1128,t1129,t113,t1130,t1131,t1132,t1133,t1134,t1135,t1136,t1137,t1138,t1139,t114,t1140,t1141,t1142,t1143,t1144,t1145,t1146,t1147,t1148,t1149,t115,t1150,t1151,t1152,t1153,t1154,t1155,t1156,t1157,t1158,t1159,t116,t1160,t1161,t1162,t1163,t1164,t1165,t1166,t1167,t1168,t1169,t117,t1170,t1171,t1172,t1173,t1174,t1175,t1176,t1177,t1178,t1179,t118,t1180,t1181,t1182,t1183,t1184,t1185,t1186,t1187,t1188,t1189,t119,t1190,t1191,t1192,t1193,t1194,t1195,t1196,t1197,t12,t120,t121,t122,t123,t124,t125,t126,t127,t1278,t1279,t128,t1288,t1289,t129,t1290,t1291,t1292,t13,t130,t131,t132,t1320,t1321,t1322,t1323,t1324,t1325,t1326,t133,t134,t135,t136,t14,t147,t148,t149,t15,t150,t151,t152,t153,t154,t155,t156,t157,t158,t159,t16,t160,t161,t162,t163,t164,t17,t18,t19,t2,t20,t21,t22,t23,t24,t249,t25,t250,t251,t252,t253,t254,t255,t256,t257,t258,t259,t26,t260,t261,t262,t263,t264,t265,t266,t267,t268,t269,t270,t271,t272,t273,t274,t275,t276,t277,t278,t279,t280,t281,t282,t283,t284,t285,t286,t287,t288,t289,t290,t291,t292,t3,t314,t315,t316,t317,t318,t319,t32,t33,t34,t349,t35,t350,t351,t352,t353,t354,t355,t356,t36,t37,t374,t375,t376,t377,t378,t379,t38,t380,t381,t382,t383,t384,t385,t386,t387,t388,t389,t39,t390,t391,t392,t393,t394,t395,t396,t397,t398,t399,t4,t40,t400,t401,t402,t403,t404,t405,t406,t407,t408,t409,t41,t410,t411,t42,t43,t432,t433,t434,t435,t436,t437,t438,t439,t44,t440,t441,t442,t443,t444,t445,t446,t447,t448,t449,t45,t450,t451,t452,t453,t454,t455,t456,t457,t458,t459,t46,t460,t461,t462,t463,t464,t465,t466,t47,t48,t49,t5,t50,t51,t52,t53,t54,t55,t594,t595,t596,t597,t598,t599,t6,t600,t601,t602,t603,t604,t605,t606,t607,t611,t612,t652,t653,t654,t655,t656,t657,t658,t659,t660,t661,t662,t663,t664,t665,t666,t667,t668,t669,t670,t671,t672,t673,t678,t679,t680,t681,t682,t683,t684,t685,t686,t687,t688,t689,t690,t691,t692,t693,t694,t695,t696,t697,t698,t699,t7,t700,t701,t702,t703,t704,t705,t706,t707,t708,t709,t710,t711,t712,t713,t714,t715,t716,t717,t718,t719,t720,t721,t722,t723,t724,t725,t726,t727,t728,t729,t730,t731,t732,t733,t734,t735,t736,t737,t738,t739,t740,t741,t742,t743,t744,t745,t746,t747,t748,t749,t750,t751,t752,t753,t754,t755,t756,t757,t758,t759,t760,t761,t762,t763,t764,t765,t766,t8,t80,t81,t82,t83,t84,t840,t841,t842,t843,t844,t85,t86,t87,t88,t89,t891,t9,t90,t908,t91,t92,t93,t94,t95,t96,t97,t98,t99] = ct{:};
t1327 = dQ1*dQ5*m6*t2*t6*t8*t10*t11*t21*2.0;
t1328 = dQ1*dQ5*m6*t3*t6*t7*t10*t11*t21*2.0;
t1329 = dQ2*dQ5*m6*t4*t6*t9*t10*t11*t21*2.0;
t1330 = dQ3*dQ5*m6*t4*t6*t9*t10*t11*t21*2.0;
t1331 = dQ4*dQ6*m6*t5*t6*t9*t10*t11*t21*2.0;
t1332 = dQ1*dQ4*m6*t4*t5*t7*t8*t10*t22*2.0;
t1333 = dQ1*dQ4*m5*t4*t5*t7*t8*t10*t25*2.0;
t1334 = dQ1*dQ4*m6*t4*t5*t7*t8*t10*t26*2.0;
t1413 = Lx4*Lycm6*dQ1*dQ6*m6*t2*t4*t5*t6*t8*t9*2.0;
t1414 = Lx4*Lycm6*dQ1*dQ6*m6*t3*t4*t5*t6*t7*t9*2.0;
t1415 = Lxcm6*Lycm6*dQ1*dQ6*m6*t2*t3*t4*t6*t10*t11*4.0;
t1416 = Lxcm6*Lz6*dQ1*dQ5*m6*t2*t3*t5*t6*t9*t10*4.0;
t1417 = Lxcm6*Lzcm6*dQ1*dQ5*m6*t2*t3*t5*t6*t9*t10*4.0;
t1420 = Ixx6*dQ1*dQ6*t2*t3*t5*t6*t9*t10*t11*2.0;
t1423 = Iyy6*dQ1*dQ6*t2*t3*t5*t6*t9*t10*t11*2.0;
t1424 = Lx4*Lxcm6*dQ1*dQ5*m6*t2*t4*t6*t8*t9*t10*2.0;
t1425 = Lx4*Lxcm6*dQ1*dQ5*m6*t3*t4*t6*t7*t9*t10*2.0;
t1426 = Lx4*Lxcm6*dQ1*dQ6*m6*t2*t4*t5*t8*t9*t11*2.0;
t1427 = Lx4*Lxcm6*dQ1*dQ6*m6*t3*t4*t5*t7*t9*t11*2.0;
t1428 = Lycm6*Lz6*dQ1*dQ4*m6*t2*t4*t6*t8*t9*t10*4.0;
t1429 = Lycm6*Lz6*dQ1*dQ4*m6*t3*t4*t6*t7*t9*t10*4.0;
t1430 = Lycm6*Lz6*dQ1*dQ5*m6*t2*t3*t5*t9*t10*t11*4.0;
t1431 = Lycm6*Lzcm6*dQ1*dQ4*m6*t2*t4*t6*t8*t9*t10*4.0;
t1432 = Lycm6*Lzcm6*dQ1*dQ4*m6*t3*t4*t6*t7*t9*t10*4.0;
t1433 = Lycm6*Lzcm6*dQ1*dQ5*m6*t2*t3*t5*t9*t10*t11*4.0;
t1434 = Lz6*Lzcm6*dQ1*dQ5*m6*t2*t4*t5*t8*t9*t10*4.0;
t1435 = Lz6*Lzcm6*dQ1*dQ5*m6*t3*t4*t5*t7*t9*t10*4.0;
t1439 = Lx4*Lycm6*dQ1*dQ5*m6*t2*t4*t8*t9*t10*t11*2.0;
t1440 = Lx4*Lycm6*dQ1*dQ5*m6*t3*t4*t7*t9*t10*t11*2.0;
t1441 = Lxcm6*Lycm6*dQ1*dQ6*m6*t4*t6*t7*t8*t10*t11*4.0;
t1442 = Lxcm6*Lz6*dQ1*dQ4*m6*t2*t4*t8*t9*t10*t11*4.0;
t1443 = Lxcm6*Lz6*dQ1*dQ4*m6*t3*t4*t7*t9*t10*t11*4.0;
t1444 = Lxcm6*Lz6*dQ1*dQ5*m6*t5*t6*t7*t8*t9*t10*4.0;
t1445 = Lxcm6*Lzcm6*dQ1*dQ4*m6*t2*t4*t8*t9*t10*t11*4.0;
t1446 = Lxcm6*Lzcm6*dQ1*dQ4*m6*t3*t4*t7*t9*t10*t11*4.0;
t1447 = Lxcm6*Lzcm6*dQ1*dQ5*m6*t5*t6*t7*t8*t9*t10*4.0;
t1448 = Ixx6*dQ1*dQ6*t5*t6*t7*t8*t9*t10*t11*2.0;
t1449 = Iyy6*dQ1*dQ6*t5*t6*t7*t8*t9*t10*t11*2.0;
t1450 = Lycm6*Lz6*dQ1*dQ5*m6*t5*t7*t8*t9*t10*t11*4.0;
t1451 = Lycm6*Lzcm6*dQ1*dQ5*m6*t5*t7*t8*t9*t10*t11*4.0;
t1523 = dQ1*dQ5*m5*t2*t4*t5*t8*t9*t10*t17*2.0;
t1524 = dQ1*dQ5*m5*t3*t4*t5*t7*t9*t10*t17*2.0;
t1525 = dQ1*dQ4*m6*t2*t3*t6*t9*t10*t11*t18*2.0;
t1526 = dQ1*dQ6*m6*t2*t4*t6*t8*t9*t11*t18*2.0;
t1527 = dQ1*dQ6*m6*t3*t4*t6*t7*t9*t11*t18*2.0;
t1528 = dQ1*dQ5*m6*t2*t4*t5*t8*t9*t10*t21*2.0;
t1529 = dQ1*dQ5*m6*t3*t4*t5*t7*t9*t10*t21*2.0;
t1530 = dQ1*dQ4*m6*t2*t3*t6*t9*t10*t11*t21*2.0;
t1531 = dQ1*dQ6*m6*t2*t4*t6*t8*t9*t11*t21*2.0;
t1532 = dQ1*dQ6*m6*t3*t4*t6*t7*t9*t11*t21*2.0;
t1533 = dQ1*dQ5*m6*t2*t4*t5*t8*t9*t10*t22*2.0;
t1534 = dQ1*dQ5*m6*t3*t4*t5*t7*t9*t10*t22*2.0;
t1535 = dQ1*dQ5*m5*t2*t4*t5*t8*t9*t10*t25*2.0;
t1536 = dQ1*dQ5*m5*t3*t4*t5*t7*t9*t10*t25*2.0;
t1537 = dQ1*dQ5*m6*t2*t4*t5*t8*t9*t10*t26*2.0;
t1538 = dQ1*dQ5*m6*t3*t4*t5*t7*t9*t10*t26*2.0;
t1543 = dQ1*dQ4*m6*t6*t7*t8*t9*t10*t11*t18*2.0;
t1544 = dQ1*dQ4*m6*t6*t7*t8*t9*t10*t11*t21*2.0;
t1581 = Lxcm6*Lycm6*dQ1*dQ4*m6*t2*t3*t4*t5*t6*t10*t11*4.0;
t1582 = Lycm6*Lz6*dQ1*dQ6*m6*t2*t4*t5*t6*t8*t9*t10*2.0;
t1583 = Lycm6*Lz6*dQ1*dQ6*m6*t3*t4*t5*t6*t7*t9*t10*2.0;
t1584 = Lycm6*Lzcm6*dQ1*dQ6*m6*t2*t4*t5*t6*t8*t9*t10*2.0;
t1585 = Lycm6*Lzcm6*dQ1*dQ6*m6*t3*t4*t5*t6*t7*t9*t10*2.0;
t1587 = Lxcm6*Lycm6*dQ1*dQ4*m6*t4*t5*t6*t7*t8*t10*t11*4.0;
t1588 = Lxcm6*Lz6*dQ1*dQ6*m6*t2*t4*t5*t8*t9*t10*t11*2.0;
t1589 = Lxcm6*Lz6*dQ1*dQ6*m6*t3*t4*t5*t7*t9*t10*t11*2.0;
t1590 = Lxcm6*Lzcm6*dQ1*dQ6*m6*t2*t4*t5*t8*t9*t10*t11*2.0;
t1591 = Lxcm6*Lzcm6*dQ1*dQ6*m6*t3*t4*t5*t7*t9*t10*t11*2.0;
t1659 = dQ1*dQ4*m6*t2*t4*t5*t6*t8*t9*t11*t18*4.0;
t1660 = dQ1*dQ4*m6*t3*t4*t5*t6*t7*t9*t11*t18*4.0;
t1661 = dQ1*dQ6*m6*t2*t3*t5*t6*t9*t10*t11*t18*2.0;
t1662 = dQ1*dQ4*m6*t2*t4*t5*t6*t8*t9*t11*t21*4.0;
t1663 = dQ1*dQ4*m6*t3*t4*t5*t6*t7*t9*t11*t21*4.0;
t1664 = dQ1*dQ6*m6*t2*t3*t5*t6*t9*t10*t11*t21*2.0;
t1665 = dQ1*dQ6*m6*t5*t6*t7*t8*t9*t10*t11*t18*2.0;
t1666 = dQ1*dQ6*m6*t5*t6*t7*t8*t9*t10*t11*t21*2.0;
t1700 = Lxcm6*Lycm6*dQ1*dQ5*m6*t2*t4*t5*t6*t8*t9*t10*t11*4.0;
t1701 = Lxcm6*Lycm6*dQ1*dQ5*m6*t3*t4*t5*t6*t7*t9*t10*t11*4.0;
t56 = -t43;
t57 = -t44;
t58 = -t46;
t59 = -t47;
t60 = Ixx4*dQ2*dQ4*t39;
t61 = Ixx4*dQ3*dQ4*t39;
t62 = Ixx6*dQ2*dQ4*t39;
t63 = Ixx5*dQ2*dQ5*t40;
t64 = Ixx6*dQ3*dQ4*t39;
t65 = Ixx5*dQ3*dQ5*t40;
t66 = Iyy4*dQ2*dQ4*t39;
t67 = Iyy4*dQ3*dQ4*t39;
t68 = Iyy5*dQ2*dQ4*t39;
t69 = Iyy5*dQ3*dQ4*t39;
t70 = Iyy6*dQ2*dQ5*t40;
t71 = Iyy6*dQ3*dQ5*t40;
t72 = Izz5*dQ2*dQ4*t39;
t73 = Izz5*dQ3*dQ4*t39;
t74 = Izz6*dQ2*dQ4*t39;
t75 = Izz5*dQ2*dQ5*t40;
t76 = Izz6*dQ3*dQ4*t39;
t77 = Izz5*dQ3*dQ5*t40;
t78 = Izz6*dQ2*dQ5*t40;
t79 = Izz6*dQ3*dQ5*t40;
t165 = -t104;
t166 = -t105;
t167 = -t106;
t168 = -t107;
t169 = -t112;
t170 = -t113;
t171 = -t84;
t172 = -t85;
t173 = -t87;
t174 = -t88;
t175 = -t89;
t176 = -t90;
t177 = -t91;
t178 = -t94;
t179 = -t119;
t180 = -t120;
t181 = -t121;
t182 = -t122;
t183 = -t123;
t184 = -t124;
t185 = -t125;
t186 = -t126;
t187 = -t129;
t188 = -t130;
t189 = -t133;
t190 = -t134;
t191 = -t135;
t192 = -t136;
t193 = Lx4*Lycm4*dQ2*dQ4*m4*t34*4.0;
t194 = Lx4*Lycm4*dQ3*dQ4*m4*t34*4.0;
t195 = Lx4*Lycm5*dQ2*dQ4*m5*t34*4.0;
t196 = Lx4*Lycm5*dQ3*dQ4*m5*t34*4.0;
t197 = Lxcm4*Lycm4*dQ2*dQ4*m4*t34*4.0;
t198 = Lxcm4*Lycm4*dQ3*dQ4*m4*t34*4.0;
t199 = Lxcm6*Lycm6*dQ2*dQ6*m6*t34*2.0;
t200 = Lxcm6*Lycm6*dQ2*dQ6*m6*t35*2.0;
t201 = Lxcm6*Lycm6*dQ3*dQ6*m6*t34*2.0;
t202 = Lxcm6*Lycm6*dQ3*dQ6*m6*t35*2.0;
t205 = Lxcm5*Lzcm5*dQ2*dQ5*m5*t35*4.0;
t206 = Lxcm5*Lzcm5*dQ3*dQ5*m5*t35*4.0;
t207 = t35*t42*2.0;
t208 = t36*t43*2.0;
t209 = t35*t45*2.0;
t210 = t36*t45*2.0;
t211 = t35*t46*2.0;
t212 = t35*t47*2.0;
t213 = Lx4*Lxcm4*dQ2*dQ4*m4*t39*2.0;
t214 = Lx4*Lxcm4*dQ3*dQ4*m4*t39*2.0;
t215 = Lz6*Lzcm6*dQ2*dQ4*m6*t39*2.0;
t216 = Lz6*Lzcm6*dQ3*dQ4*m6*t39*2.0;
t217 = Lz6*Lzcm6*dQ2*dQ5*m6*t40*2.0;
t218 = Lz6*Lzcm6*dQ3*dQ5*m6*t40*2.0;
t219 = dQ2*dQ4*m4*t14*t39;
t220 = dQ2*dQ4*m5*t14*t39;
t221 = dQ3*dQ4*m4*t14*t39;
t222 = dQ2*dQ4*m6*t14*t39;
t223 = dQ3*dQ4*m5*t14*t39;
t224 = dQ3*dQ4*m6*t14*t39;
t225 = dQ2*dQ4*m4*t16*t39;
t226 = dQ3*dQ4*m4*t16*t39;
t227 = dQ2*dQ5*m5*t17*t40;
t228 = dQ2*dQ4*m6*t18*t39;
t229 = dQ3*dQ5*m5*t17*t40;
t230 = dQ3*dQ4*m6*t18*t39;
t231 = dQ2*dQ4*m4*t19*t39;
t232 = dQ3*dQ4*m4*t19*t39;
t233 = dQ2*dQ4*m5*t20*t39;
t234 = dQ3*dQ4*m5*t20*t39;
t235 = dQ2*dQ5*m6*t21*t40;
t236 = dQ3*dQ5*m6*t21*t40;
t237 = dQ2*dQ4*m6*t22*t39;
t238 = dQ3*dQ4*m6*t22*t39;
t239 = dQ2*dQ5*m6*t22*t40;
t240 = dQ3*dQ5*m6*t22*t40;
t241 = dQ2*dQ4*m5*t25*t39;
t242 = dQ3*dQ4*m5*t25*t39;
t243 = dQ2*dQ5*m5*t25*t40;
t244 = dQ2*dQ4*m6*t26*t39;
t245 = dQ3*dQ5*m5*t25*t40;
t246 = dQ3*dQ4*m6*t26*t39;
t247 = dQ2*dQ5*m6*t26*t40;
t248 = dQ3*dQ5*m6*t26*t40;
t301 = Lxcm5*Lzcm5*dQ2*dQ5*m5*t34*-2.0;
t302 = Lxcm5*Lzcm5*dQ3*dQ5*m5*t34*-2.0;
t320 = -t249;
t321 = -t250;
t322 = -t251;
t323 = -t148;
t324 = -t149;
t325 = -t150;
t326 = -t258;
t327 = -t259;
t328 = -t260;
t329 = -t261;
t330 = -t151;
t331 = -t267;
t332 = -t155;
t333 = -t156;
t334 = -t268;
t335 = -t269;
t336 = -t270;
t337 = -t271;
t338 = -t272;
t339 = -t273;
t340 = -t274;
t341 = -t275;
t342 = -t276;
t343 = -t283;
t344 = -t284;
t345 = -t285;
t346 = -t286;
t347 = -t287;
t348 = -t288;
t357 = -t159;
t358 = -t162;
t359 = Lx4*Lxcm5*dQ2*dQ5*m5*t10*t34*2.0;
t360 = Lx4*Lxcm5*dQ3*dQ5*m5*t10*t34*2.0;
t361 = Lx4*Lxcm6*dQ2*dQ4*m6*t11*t34*4.0;
t362 = Lx4*Lxcm6*dQ3*dQ4*m6*t11*t34*4.0;
t363 = t34*t129;
t364 = t34*t130;
t365 = Lycm6*Lz6*dQ2*dQ5*m6*t11*t35*4.0;
t366 = Lycm6*Lz6*dQ3*dQ5*m6*t11*t35*4.0;
t367 = Lycm5*Lzcm5*dQ2*dQ4*m5*t10*t34*4.0;
t368 = Lycm5*Lzcm5*dQ3*dQ4*m5*t10*t34*4.0;
t369 = t34*t133;
t370 = t34*t134;
t371 = Lycm6*Lzcm6*dQ2*dQ5*m6*t11*t35*4.0;
t372 = Lycm6*Lzcm6*dQ3*dQ5*m6*t11*t35*4.0;
t373 = Lz6*Lzcm6*dQ4*dQ5*m6*t9*t35*4.0;
t467 = Lx4*Lycm6*dQ2*dQ4*m6*t6*t34*4.0;
t468 = Lx4*Lycm6*dQ3*dQ4*m6*t6*t34*4.0;
t469 = Lxcm5*Lycm5*dQ2*dQ4*m5*t5*t34*4.0;
t470 = Lxcm5*Lycm5*dQ3*dQ4*m5*t5*t34*4.0;
t471 = Lxcm6*Lycm6*dQ2*dQ4*m6*t5*t34*4.0;
t472 = Lxcm6*Lycm6*dQ3*dQ4*m6*t5*t34*4.0;
t473 = Lxcm6*Lycm6*dQ2*dQ4*m6*t5*t36*4.0;
t474 = Lxcm6*Lycm6*dQ3*dQ4*m6*t5*t36*4.0;
t475 = Lxcm6*Lycm6*dQ5*dQ6*m6*t4*t36*4.0;
t476 = Lx4*Lz6*dQ2*dQ5*m6*t5*t34*2.0;
t477 = Lx4*Lz6*dQ3*dQ5*m6*t5*t34*2.0;
t478 = Lx4*Lzcm5*dQ2*dQ5*m5*t5*t34*2.0;
t479 = Lx4*Lzcm5*dQ3*dQ5*m5*t5*t34*2.0;
t480 = Lx4*Lzcm6*dQ2*dQ5*m6*t5*t34*2.0;
t481 = Lx4*Lzcm6*dQ3*dQ5*m6*t5*t34*2.0;
t484 = Lxcm6*Lz6*dQ2*dQ5*m6*t6*t35*4.0;
t485 = Lxcm6*Lz6*dQ3*dQ5*m6*t6*t35*4.0;
t488 = Lxcm6*Lzcm6*dQ2*dQ5*m6*t6*t35*4.0;
t489 = Lxcm6*Lzcm6*dQ3*dQ5*m6*t6*t35*4.0;
t490 = t34*t80*2.0;
t491 = t34*t81*2.0;
t492 = t34*t84*2.0;
t493 = t34*t85*2.0;
t494 = t36*t84*2.0;
t495 = t36*t85*2.0;
t496 = Ixx5*dQ2*dQ4*t4*t9*t35*2.0;
t497 = Ixx5*dQ3*dQ4*t4*t9*t35*2.0;
t498 = Ixx5*dQ2*dQ5*t5*t10*t34*2.0;
t499 = Ixx6*dQ2*dQ4*t4*t9*t36*2.0;
t500 = Ixx5*dQ3*dQ5*t5*t10*t34*2.0;
t501 = Ixx6*dQ3*dQ4*t4*t9*t36*2.0;
t502 = Ixx6*dQ2*dQ5*t5*t10*t36*2.0;
t503 = Ixx6*dQ2*dQ6*t6*t11*t34*2.0;
t504 = Ixx6*dQ3*dQ5*t5*t10*t36*2.0;
t505 = Ixx6*dQ2*dQ6*t6*t11*t35*2.0;
t506 = Ixx6*dQ3*dQ6*t6*t11*t34*2.0;
t507 = t36*t86*2.0;
t508 = Ixx6*dQ3*dQ6*t6*t11*t35*2.0;
t509 = t36*t87*2.0;
t510 = t34*t88*2.0;
t511 = t34*t89*2.0;
t512 = t34*t90*2.0;
t513 = t34*t91*2.0;
t514 = t36*t92*2.0;
t515 = t36*t93*2.0;
t516 = Iyy6*dQ2*dQ4*t4*t9*t35*2.0;
t517 = Iyy6*dQ2*dQ4*t4*t9*t36*2.0;
t518 = Iyy6*dQ3*dQ4*t4*t9*t35*2.0;
t519 = Iyy6*dQ2*dQ5*t5*t10*t34*2.0;
t520 = Iyy6*dQ3*dQ4*t4*t9*t36*2.0;
t521 = Iyy6*dQ3*dQ5*t5*t10*t34*2.0;
t522 = Iyy6*dQ2*dQ5*t5*t10*t36*2.0;
t523 = Iyy6*dQ2*dQ6*t6*t11*t34*2.0;
t524 = Iyy6*dQ3*dQ5*t5*t10*t36*2.0;
t525 = Iyy6*dQ2*dQ6*t6*t11*t35*2.0;
t526 = Iyy6*dQ3*dQ6*t6*t11*t34*2.0;
t527 = t36*t94*2.0;
t528 = Iyy6*dQ3*dQ6*t6*t11*t35*2.0;
t529 = t36*t95*2.0;
t530 = t34*t98*2.0;
t531 = t34*t99*2.0;
t532 = t34*t100*2.0;
t533 = t34*t101*2.0;
t534 = Izz5*dQ2*dQ4*t4*t9*t35*2.0;
t535 = Izz5*dQ3*dQ4*t4*t9*t35*2.0;
t536 = Izz6*dQ2*dQ4*t4*t9*t35*2.0;
t537 = Izz5*dQ2*dQ5*t5*t10*t34*2.0;
t538 = Izz6*dQ3*dQ4*t4*t9*t35*2.0;
t539 = Izz5*dQ3*dQ5*t5*t10*t34*2.0;
t540 = Izz6*dQ2*dQ5*t5*t10*t34*2.0;
t541 = Izz6*dQ3*dQ5*t5*t10*t34*2.0;
t549 = t35*t135;
t550 = dQ4*dQ5*m6*t9*t18*t36*2.0;
t551 = t35*t136;
t552 = t36*t136;
t553 = dQ4*dQ5*m6*t9*t22*t35*2.0;
t554 = dQ4*dQ5*m5*t9*t25*t35*2.0;
t555 = dQ4*dQ5*m6*t9*t26*t35*2.0;
t556 = -t374;
t557 = -t375;
t558 = -t376;
t559 = -t377;
t560 = -t378;
t561 = -t379;
t562 = -t381;
t563 = -t315;
t564 = -t390;
t565 = -t391;
t566 = -t392;
t567 = -t393;
t568 = -t394;
t569 = -t395;
t570 = -t396;
t571 = -t397;
t572 = -t398;
t573 = -t399;
t574 = -t400;
t575 = -t405;
t576 = -t406;
t577 = -t407;
t578 = -t408;
t579 = -t432;
t580 = -t433;
t581 = -t434;
t582 = -t435;
t583 = -t444;
t584 = -t445;
t585 = -t448;
t586 = -t449;
t587 = -t452;
t588 = -t453;
t589 = -t455;
t590 = -t456;
t591 = -t457;
t592 = -t458;
t593 = -t462;
t608 = -t317;
t609 = -t319;
t610 = -t466;
t618 = Lxcm6*Lz6*dQ2*dQ5*m6*t6*t34*-2.0;
t619 = Lxcm6*Lz6*dQ3*dQ5*m6*t6*t34*-2.0;
t622 = Lxcm6*Lzcm6*dQ2*dQ5*m6*t6*t34*-2.0;
t623 = Lxcm6*Lzcm6*dQ3*dQ5*m6*t6*t34*-2.0;
t769 = Lxcm6*Lycm6*dQ2*dQ6*m6*t34*t36*4.0;
t770 = Lxcm6*Lycm6*dQ2*dQ6*m6*t35*t36*4.0;
t771 = Lxcm6*Lycm6*dQ3*dQ6*m6*t34*t36*4.0;
t772 = Lxcm6*Lycm6*dQ3*dQ6*m6*t35*t36*4.0;
t777 = -t594;
t778 = -t601;
t779 = -t602;
t780 = -t603;
t781 = -t604;
t782 = -t605;
t783 = -t606;
t784 = Lx4*Lycm6*dQ2*dQ6*m6*t5*t6*t34*2.0;
t785 = Lx4*Lycm6*dQ3*dQ6*m6*t5*t6*t34*2.0;
t786 = t35*t147*2.0;
t787 = t36*t148*2.0;
t788 = t34*t149*2.0;
t789 = t34*t150*2.0;
t790 = t36*t149*2.0;
t791 = t36*t150*2.0;
t792 = Ixx6*dQ2*dQ4*t5*t6*t11*t34*4.0;
t793 = Ixx6*dQ2*dQ6*t4*t5*t9*t36*4.0;
t794 = Ixx6*dQ3*dQ4*t5*t6*t11*t34*4.0;
t795 = Ixx6*dQ3*dQ6*t4*t5*t9*t36*4.0;
t796 = t35*t152*2.0;
t797 = t36*t152*2.0;
t798 = t34*t153*2.0;
t799 = t34*t154*2.0;
t800 = t36*t153*2.0;
t801 = t36*t154*2.0;
t802 = Iyy6*dQ2*dQ4*t5*t6*t11*t34*4.0;
t803 = Iyy6*dQ2*dQ6*t4*t5*t9*t36*4.0;
t804 = Iyy6*dQ3*dQ4*t5*t6*t11*t34*4.0;
t805 = Iyy6*dQ3*dQ6*t4*t5*t9*t36*4.0;
t806 = t35*t155*2.0;
t807 = t35*t156*2.0;
t808 = Lx4*Lxcm4*dQ1*dQ4*m4*t2*t8*t34*4.0;
t809 = Lx4*Lxcm4*dQ1*dQ4*m4*t3*t7*t34*4.0;
t810 = Lx4*Lxcm6*dQ2*dQ5*m6*t6*t10*t34*2.0;
t811 = Lx4*Lxcm6*dQ2*dQ6*m6*t5*t11*t34*2.0;
t812 = Lx4*Lxcm6*dQ3*dQ5*m6*t6*t10*t34*2.0;
t813 = Lx4*Lxcm6*dQ3*dQ6*m6*t5*t11*t34*2.0;
t814 = Lycm6*Lz6*dQ2*dQ4*m6*t6*t10*t34*4.0;
t815 = Lycm6*Lz6*dQ3*dQ4*m6*t6*t10*t34*4.0;
t816 = Lycm6*Lz6*dQ4*dQ6*m6*t6*t9*t35*2.0;
t817 = Lycm6*Lzcm6*dQ2*dQ4*m6*t6*t10*t34*4.0;
t818 = Lycm6*Lzcm6*dQ3*dQ4*m6*t6*t10*t34*4.0;
t819 = Lycm6*Lzcm6*dQ4*dQ6*m6*t6*t9*t35*2.0;
t820 = Lz6*Lzcm6*dQ1*dQ4*m6*t2*t8*t34*4.0;
t821 = Lz6*Lzcm6*dQ1*dQ4*m6*t3*t7*t34*4.0;
t822 = Lz6*Lzcm6*dQ2*dQ4*m6*t4*t9*t35*4.0;
t823 = Lz6*Lzcm6*dQ3*dQ4*m6*t4*t9*t35*4.0;
t824 = Lz6*Lzcm6*dQ2*dQ5*m6*t5*t10*t34*4.0;
t825 = Lz6*Lzcm6*dQ3*dQ5*m6*t5*t10*t34*4.0;
t826 = Lx4*Lycm6*dQ2*dQ5*m6*t10*t11*t34*2.0;
t827 = Lx4*Lycm6*dQ3*dQ5*m6*t10*t11*t34*2.0;
t828 = Lxcm6*Lz6*dQ2*dQ4*m6*t10*t11*t34*4.0;
t829 = Lxcm6*Lz6*dQ3*dQ4*m6*t10*t11*t34*4.0;
t830 = Lxcm6*Lz6*dQ4*dQ6*m6*t9*t11*t35*2.0;
t831 = Lxcm6*Lzcm6*dQ2*dQ4*m6*t10*t11*t34*4.0;
t832 = Lxcm6*Lzcm6*dQ3*dQ4*m6*t10*t11*t34*4.0;
t833 = Lxcm6*Lzcm6*dQ4*dQ6*m6*t9*t11*t35*2.0;
t834 = t35*t159*2.0;
t835 = t36*t160*2.0;
t836 = t35*t162*2.0;
t837 = t36*t162*2.0;
t838 = t35*t163*2.0;
t839 = t35*t164*2.0;
t845 = -t652;
t846 = -t653;
t847 = -t661;
t848 = -t662;
t849 = -t663;
t850 = -t664;
t851 = -t665;
t852 = -t666;
t853 = -t667;
t854 = -t669;
t855 = -t670;
t856 = -t671;
t857 = -t672;
t858 = -t673;
t859 = -t678;
t860 = -t679;
t861 = -t680;
t862 = -t681;
t863 = -t682;
t864 = -t683;
t865 = -t684;
t866 = -t685;
t867 = -t688;
t868 = -t689;
t869 = -t690;
t870 = -t698;
t871 = -t699;
t872 = -t700;
t873 = -t717;
t874 = -t718;
t875 = -t719;
t876 = -t720;
t877 = -t721;
t878 = -t722;
t879 = -t723;
t880 = -t725;
t881 = -t726;
t882 = -t727;
t883 = -t728;
t884 = -t729;
t885 = -t730;
t886 = -t731;
t887 = -t732;
t888 = -t733;
t889 = -t734;
t890 = -t735;
t892 = -t738;
t893 = -t739;
t894 = -t740;
t895 = -t741;
t896 = -t748;
t897 = -t749;
t898 = -t750;
t899 = -t751;
t900 = -t752;
t901 = -t753;
t902 = -t754;
t903 = -t755;
t904 = -t759;
t905 = -t760;
t906 = -t764;
t907 = -t766;
t911 = t35*t36*t43*-2.0;
t937 = dQ1*dQ4*m4*t2*t8*t14*t34*2.0;
t938 = dQ1*dQ4*m4*t3*t7*t14*t34*2.0;
t939 = dQ1*dQ4*m5*t2*t8*t14*t34*2.0;
t940 = dQ1*dQ4*m5*t3*t7*t14*t34*2.0;
t941 = dQ1*dQ4*m6*t2*t8*t14*t34*2.0;
t942 = dQ1*dQ4*m6*t3*t7*t14*t34*2.0;
t943 = dQ1*dQ4*m4*t2*t8*t16*t34*2.0;
t944 = dQ1*dQ4*m4*t3*t7*t16*t34*2.0;
t945 = t34*t349;
t946 = t34*t350;
t947 = t36*t349;
t948 = t36*t350;
t949 = dQ2*dQ4*m5*t4*t9*t17*t35*2.0;
t950 = dQ3*dQ4*m5*t4*t9*t17*t35*2.0;
t951 = dQ2*dQ5*m5*t5*t10*t17*t34*2.0;
out1 = ft_2({Ixx2,Ixx3,Ixx4,Ixx5,Ixx6,Iyy4,Iyy5,Iyy6,Izz2,Izz3,Izz4,Izz5,Izz6,Lx2,Lx3,Lx4,Lxcm2,Lxcm3,Lxcm4,Lxcm5,Lxcm6,Lycm3,Lycm4,Lycm5,Lycm6,Lz6,Lzcm2,Lzcm3,Lzcm4,Lzcm5,Lzcm6,dQ1,dQ2,dQ3,dQ4,dQ5,dQ6,m2,m3,m4,m5,m6,t10,t100,t101,t102,t103,t108,t1080,t1081,t1082,t1083,t1084,t1085,t1086,t1087,t1088,t1089,t109,t11,t110,t111,t1116,t1117,t1118,t1119,t112,t1120,t1121,t1122,t1123,t1124,t1125,t1126,t1127,t1128,t1129,t113,t1130,t1131,t1132,t1133,t1134,t1135,t1136,t1137,t1138,t1139,t114,t1140,t1141,t1142,t1143,t1144,t1145,t1146,t1147,t1148,t1149,t115,t1150,t1151,t1152,t1153,t1154,t1155,t1156,t1157,t1158,t1159,t116,t1160,t1161,t1162,t1163,t1164,t1165,t1166,t1167,t1168,t1169,t117,t1170,t1171,t1172,t1173,t1174,t1175,t1176,t1177,t1178,t1179,t118,t1180,t1181,t1182,t1183,t1184,t1185,t1186,t1187,t1188,t1189,t1190,t1191,t1192,t1193,t1194,t1195,t1196,t1197,t12,t127,t1278,t1279,t128,t1288,t1289,t129,t1290,t1291,t1292,t13,t130,t131,t132,t1320,t1321,t1322,t1323,t1324,t1325,t1326,t1327,t1328,t1329,t133,t1330,t1331,t1332,t1333,t1334,t134,t14,t1413,t1414,t1415,t1416,t1417,t1420,t1423,t1424,t1425,t1426,t1427,t1428,t1429,t1430,t1431,t1432,t1433,t1434,t1435,t1439,t1440,t1441,t1442,t1443,t1444,t1445,t1446,t1447,t1448,t1449,t1450,t1451,t147,t148,t149,t15,t150,t152,t1523,t1524,t1525,t1526,t1527,t1528,t1529,t153,t1530,t1531,t1532,t1533,t1534,t1535,t1536,t1537,t1538,t154,t1543,t1544,t157,t158,t1581,t1582,t1583,t1584,t1585,t1587,t1588,t1589,t1590,t1591,t16,t160,t161,t162,t163,t164,t165,t1659,t166,t1660,t1661,t1662,t1663,t1664,t1665,t1666,t167,t168,t169,t17,t170,t1700,t1701,t171,t172,t173,t174,t175,t176,t177,t178,t179,t18,t180,t181,t182,t183,t184,t185,t186,t187,t188,t189,t19,t190,t191,t192,t193,t194,t195,t196,t197,t198,t199,t2,t20,t200,t201,t202,t205,t206,t207,t208,t209,t21,t210,t211,t212,t213,t214,t215,t216,t217,t218,t219,t22,t220,t221,t222,t223,t224,t225,t226,t227,t228,t229,t23,t230,t231,t232,t233,t234,t235,t236,t237,t238,t239,t24,t240,t241,t242,t243,t244,t245,t246,t247,t248,t25,t252,t253,t254,t255,t256,t257,t26,t260,t261,t262,t263,t264,t265,t266,t277,t278,t279,t280,t281,t282,t289,t290,t291,t292,t3,t301,t302,t314,t315,t316,t317,t318,t32,t320,t321,t322,t323,t324,t325,t326,t327,t328,t329,t33,t330,t331,t332,t333,t334,t335,t336,t337,t338,t339,t34,t340,t341,t342,t343,t344,t345,t346,t347,t348,t349,t35,t350,t351,t352,t353,t354,t355,t356,t357,t358,t359,t36,t360,t361,t362,t363,t364,t365,t366,t367,t368,t369,t37,t370,t371,t372,t373,t38,t380,t382,t383,t384,t385,t386,t387,t388,t389,t39,t4,t40,t401,t402,t403,t404,t405,t406,t409,t41,t410,t411,t42,t436,t437,t438,t439,t440,t441,t442,t443,t444,t445,t446,t447,t45,t450,t451,t454,t459,t460,t461,t463,t464,t465,t467,t468,t469,t470,t471,t472,t473,t474,t475,t476,t477,t478,t479,t48,t480,t481,t484,t485,t488,t489,t49,t490,t491,t492,t493,t494,t495,t496,t497,t498,t499,t5,t50,t500,t501,t502,t503,t504,t505,t506,t507,t508,t509,t51,t510,t511,t512,t513,t514,t515,t516,t517,t518,t519,t52,t520,t521,t522,t523,t524,t525,t526,t527,t528,t529,t53,t530,t531,t532,t533,t534,t535,t536,t537,t538,t539,t54,t540,t541,t549,t55,t550,t551,t552,t553,t554,t555,t556,t557,t558,t559,t56,t560,t561,t562,t563,t564,t565,t566,t567,t568,t569,t57,t570,t571,t572,t573,t574,t575,t576,t577,t578,t579,t58,t580,t581,t582,t583,t584,t585,t586,t587,t588,t589,t59,t590,t591,t592,t593,t594,t595,t596,t597,t598,t599,t6,t60,t600,t602,t605,t606,t607,t608,t609,t61,t610,t611,t612,t618,t619,t62,t622,t623,t63,t64,t65,t653,t654,t655,t656,t657,t658,t659,t66,t660,t664,t665,t668,t67,t670,t671,t68,t686,t687,t69,t691,t692,t693,t694,t695,t696,t697,t698,t699,t7,t70,t701,t702,t703,t704,t705,t706,t707,t708,t709,t71,t710,t711,t712,t713,t714,t715,t716,t718,t719,t72,t724,t728,t729,t73,t736,t737,t738,t739,t74,t742,t743,t744,t745,t746,t747,t75,t756,t757,t758,t76,t761,t762,t763,t765,t769,t77,t770,t771,t772,t777,t778,t779,t78,t780,t781,t782,t783,t784,t785,t786,t787,t788,t789,t79,t790,t791,t792,t793,t794,t795,t796,t797,t798,t799,t8,t80,t800,t801,t802,t803,t804,t805,t806,t807,t808,t809,t81,t810,t811,t812,t813,t814,t815,t816,t817,t818,t819,t82,t820,t821,t822,t823,t824,t825,t826,t827,t828,t829,t83,t830,t831,t832,t833,t834,t835,t836,t837,t838,t839,t84,t840,t841,t842,t843,t844,t845,t846,t847,t848,t849,t85,t850,t851,t852,t853,t854,t855,t856,t857,t858,t859,t86,t860,t861,t862,t863,t864,t865,t866,t867,t868,t869,t870,t871,t872,t873,t874,t875,t876,t877,t878,t879,t88,t880,t881,t882,t883,t884,t885,t886,t887,t888,t889,t890,t891,t892,t893,t894,t895,t896,t897,t898,t899,t9,t90,t900,t901,t902,t903,t904,t905,t906,t907,t908,t91,t911,t92,t93,t937,t938,t939,t94,t940,t941,t942,t943,t944,t945,t946,t947,t948,t949,t95,t950,t951,t96,t97,t98,t99});
end
function out1 = ft_2(ct)
[Ixx2,Ixx3,Ixx4,Ixx5,Ixx6,Iyy4,Iyy5,Iyy6,Izz2,Izz3,Izz4,Izz5,Izz6,Lx2,Lx3,Lx4,Lxcm2,Lxcm3,Lxcm4,Lxcm5,Lxcm6,Lycm3,Lycm4,Lycm5,Lycm6,Lz6,Lzcm2,Lzcm3,Lzcm4,Lzcm5,Lzcm6,dQ1,dQ2,dQ3,dQ4,dQ5,dQ6,m2,m3,m4,m5,m6,t10,t100,t101,t102,t103,t108,t1080,t1081,t1082,t1083,t1084,t1085,t1086,t1087,t1088,t1089,t109,t11,t110,t111,t1116,t1117,t1118,t1119,t112,t1120,t1121,t1122,t1123,t1124,t1125,t1126,t1127,t1128,t1129,t113,t1130,t1131,t1132,t1133,t1134,t1135,t1136,t1137,t1138,t1139,t114,t1140,t1141,t1142,t1143,t1144,t1145,t1146,t1147,t1148,t1149,t115,t1150,t1151,t1152,t1153,t1154,t1155,t1156,t1157,t1158,t1159,t116,t1160,t1161,t1162,t1163,t1164,t1165,t1166,t1167,t1168,t1169,t117,t1170,t1171,t1172,t1173,t1174,t1175,t1176,t1177,t1178,t1179,t118,t1180,t1181,t1182,t1183,t1184,t1185,t1186,t1187,t1188,t1189,t1190,t1191,t1192,t1193,t1194,t1195,t1196,t1197,t12,t127,t1278,t1279,t128,t1288,t1289,t129,t1290,t1291,t1292,t13,t130,t131,t132,t1320,t1321,t1322,t1323,t1324,t1325,t1326,t1327,t1328,t1329,t133,t1330,t1331,t1332,t1333,t1334,t134,t14,t1413,t1414,t1415,t1416,t1417,t1420,t1423,t1424,t1425,t1426,t1427,t1428,t1429,t1430,t1431,t1432,t1433,t1434,t1435,t1439,t1440,t1441,t1442,t1443,t1444,t1445,t1446,t1447,t1448,t1449,t1450,t1451,t147,t148,t149,t15,t150,t152,t1523,t1524,t1525,t1526,t1527,t1528,t1529,t153,t1530,t1531,t1532,t1533,t1534,t1535,t1536,t1537,t1538,t154,t1543,t1544,t157,t158,t1581,t1582,t1583,t1584,t1585,t1587,t1588,t1589,t1590,t1591,t16,t160,t161,t162,t163,t164,t165,t1659,t166,t1660,t1661,t1662,t1663,t1664,t1665,t1666,t167,t168,t169,t17,t170,t1700,t1701,t171,t172,t173,t174,t175,t176,t177,t178,t179,t18,t180,t181,t182,t183,t184,t185,t186,t187,t188,t189,t19,t190,t191,t192,t193,t194,t195,t196,t197,t198,t199,t2,t20,t200,t201,t202,t205,t206,t207,t208,t209,t21,t210,t211,t212,t213,t214,t215,t216,t217,t218,t219,t22,t220,t221,t222,t223,t224,t225,t226,t227,t228,t229,t23,t230,t231,t232,t233,t234,t235,t236,t237,t238,t239,t24,t240,t241,t242,t243,t244,t245,t246,t247,t248,t25,t252,t253,t254,t255,t256,t257,t26,t260,t261,t262,t263,t264,t265,t266,t277,t278,t279,t280,t281,t282,t289,t290,t291,t292,t3,t301,t302,t314,t315,t316,t317,t318,t32,t320,t321,t322,t323,t324,t325,t326,t327,t328,t329,t33,t330,t331,t332,t333,t334,t335,t336,t337,t338,t339,t34,t340,t341,t342,t343,t344,t345,t346,t347,t348,t349,t35,t350,t351,t352,t353,t354,t355,t356,t357,t358,t359,t36,t360,t361,t362,t363,t364,t365,t366,t367,t368,t369,t37,t370,t371,t372,t373,t38,t380,t382,t383,t384,t385,t386,t387,t388,t389,t39,t4,t40,t401,t402,t403,t404,t405,t406,t409,t41,t410,t411,t42,t436,t437,t438,t439,t440,t441,t442,t443,t444,t445,t446,t447,t45,t450,t451,t454,t459,t460,t461,t463,t464,t465,t467,t468,t469,t470,t471,t472,t473,t474,t475,t476,t477,t478,t479,t48,t480,t481,t484,t485,t488,t489,t49,t490,t491,t492,t493,t494,t495,t496,t497,t498,t499,t5,t50,t500,t501,t502,t503,t504,t505,t506,t507,t508,t509,t51,t510,t511,t512,t513,t514,t515,t516,t517,t518,t519,t52,t520,t521,t522,t523,t524,t525,t526,t527,t528,t529,t53,t530,t531,t532,t533,t534,t535,t536,t537,t538,t539,t54,t540,t541,t549,t55,t550,t551,t552,t553,t554,t555,t556,t557,t558,t559,t56,t560,t561,t562,t563,t564,t565,t566,t567,t568,t569,t57,t570,t571,t572,t573,t574,t575,t576,t577,t578,t579,t58,t580,t581,t582,t583,t584,t585,t586,t587,t588,t589,t59,t590,t591,t592,t593,t594,t595,t596,t597,t598,t599,t6,t60,t600,t602,t605,t606,t607,t608,t609,t61,t610,t611,t612,t618,t619,t62,t622,t623,t63,t64,t65,t653,t654,t655,t656,t657,t658,t659,t66,t660,t664,t665,t668,t67,t670,t671,t68,t686,t687,t69,t691,t692,t693,t694,t695,t696,t697,t698,t699,t7,t70,t701,t702,t703,t704,t705,t706,t707,t708,t709,t71,t710,t711,t712,t713,t714,t715,t716,t718,t719,t72,t724,t728,t729,t73,t736,t737,t738,t739,t74,t742,t743,t744,t745,t746,t747,t75,t756,t757,t758,t76,t761,t762,t763,t765,t769,t77,t770,t771,t772,t777,t778,t779,t78,t780,t781,t782,t783,t784,t785,t786,t787,t788,t789,t79,t790,t791,t792,t793,t794,t795,t796,t797,t798,t799,t8,t80,t800,t801,t802,t803,t804,t805,t806,t807,t808,t809,t81,t810,t811,t812,t813,t814,t815,t816,t817,t818,t819,t82,t820,t821,t822,t823,t824,t825,t826,t827,t828,t829,t83,t830,t831,t832,t833,t834,t835,t836,t837,t838,t839,t84,t840,t841,t842,t843,t844,t845,t846,t847,t848,t849,t85,t850,t851,t852,t853,t854,t855,t856,t857,t858,t859,t86,t860,t861,t862,t863,t864,t865,t866,t867,t868,t869,t870,t871,t872,t873,t874,t875,t876,t877,t878,t879,t88,t880,t881,t882,t883,t884,t885,t886,t887,t888,t889,t890,t891,t892,t893,t894,t895,t896,t897,t898,t899,t9,t90,t900,t901,t902,t903,t904,t905,t906,t907,t908,t91,t911,t92,t93,t937,t938,t939,t94,t940,t941,t942,t943,t944,t945,t946,t947,t948,t949,t95,t950,t951,t96,t97,t98,t99] = ct{:};
t952 = dQ3*dQ5*m5*t5*t10*t17*t34*2.0;
t953 = dQ2*dQ4*m6*t4*t9*t18*t36*2.0;
t954 = dQ3*dQ4*m6*t4*t9*t18*t36*2.0;
t955 = dQ2*dQ5*m6*t5*t10*t18*t36*2.0;
t956 = dQ2*dQ6*m6*t6*t11*t18*t34*2.0;
t957 = dQ3*dQ5*m6*t5*t10*t18*t36*2.0;
t958 = dQ2*dQ6*m6*t6*t11*t18*t35*2.0;
t959 = dQ3*dQ6*m6*t6*t11*t18*t34*2.0;
t960 = dQ4*dQ6*m6*t4*t10*t18*t36*2.0;
t961 = dQ3*dQ6*m6*t6*t11*t18*t35*2.0;
t967 = dQ1*dQ4*m6*t2*t8*t21*t36*2.0;
t968 = dQ1*dQ4*m6*t3*t7*t21*t36*2.0;
t969 = dQ2*dQ4*m6*t4*t9*t21*t35*2.0;
t970 = dQ2*dQ4*m6*t4*t9*t21*t36*2.0;
t971 = dQ3*dQ4*m6*t4*t9*t21*t35*2.0;
t972 = dQ2*dQ5*m6*t5*t10*t21*t34*2.0;
t973 = dQ3*dQ4*m6*t4*t9*t21*t36*2.0;
t974 = dQ3*dQ5*m6*t5*t10*t21*t34*2.0;
t975 = dQ2*dQ5*m6*t5*t10*t21*t36*2.0;
t976 = dQ2*dQ6*m6*t6*t11*t21*t34*2.0;
t977 = dQ3*dQ5*m6*t5*t10*t21*t36*2.0;
t978 = dQ2*dQ6*m6*t6*t11*t21*t35*2.0;
t979 = dQ3*dQ6*m6*t6*t11*t21*t34*2.0;
t981 = dQ3*dQ6*m6*t6*t11*t21*t35*2.0;
t982 = dQ5*dQ6*m6*t5*t9*t21*t36*2.0;
t983 = dQ1*dQ4*m6*t2*t8*t22*t34*2.0;
t984 = dQ1*dQ4*m6*t3*t7*t22*t34*2.0;
t985 = dQ2*dQ4*m6*t4*t9*t22*t35*2.0;
t986 = dQ3*dQ4*m6*t4*t9*t22*t35*2.0;
t987 = dQ2*dQ5*m6*t5*t10*t22*t34*2.0;
t988 = dQ3*dQ5*m6*t5*t10*t22*t34*2.0;
t989 = dQ1*dQ4*m5*t2*t8*t25*t34*2.0;
t990 = dQ1*dQ4*m5*t3*t7*t25*t34*2.0;
t991 = dQ1*dQ4*m6*t2*t8*t26*t34*2.0;
t992 = dQ1*dQ4*m6*t3*t7*t26*t34*2.0;
t993 = dQ2*dQ4*m5*t4*t9*t25*t35*2.0;
t994 = dQ3*dQ4*m5*t4*t9*t25*t35*2.0;
t995 = dQ2*dQ5*m5*t5*t10*t25*t34*2.0;
t996 = dQ2*dQ4*m6*t4*t9*t26*t35*2.0;
t997 = dQ3*dQ5*m5*t5*t10*t25*t34*2.0;
t998 = dQ3*dQ4*m6*t4*t9*t26*t35*2.0;
t999 = dQ2*dQ5*m6*t5*t10*t26*t34*2.0;
t1000 = dQ3*dQ5*m6*t5*t10*t26*t34*2.0;
t1004 = -t840;
t1005 = -t841;
t1006 = -t842;
t1011 = t34*t35*t82*2.0;
t1012 = t34*t35*t83*2.0;
t1021 = t34*t35*t92*2.0;
t1022 = t34*t35*t93*2.0;
t1039 = -t908;
t1040 = Lxcm5*Lzcm5*dQ1*dQ4*m5*t2*t3*t4*t35*4.0;
t1041 = t36*t314*2.0;
t1042 = t36*t315*2.0;
t1043 = Lx4*Lxcm5*dQ1*dQ4*m5*t2*t5*t8*t34*4.0;
t1044 = Lx4*Lxcm5*dQ1*dQ4*m5*t3*t5*t7*t34*4.0;
t1045 = Lx4*Lxcm6*dQ1*dQ6*m6*t2*t6*t8*t34*2.0;
t1046 = Lx4*Lxcm6*dQ1*dQ6*m6*t3*t6*t7*t34*2.0;
t1049 = t34*t405;
t1050 = t34*t406;
t1053 = Lz6*Lzcm6*dQ1*dQ5*m6*t2*t3*t9*t35*4.0;
t1054 = Lx4*Lycm6*dQ1*dQ6*m6*t2*t8*t11*t34*2.0;
t1055 = Lx4*Lycm6*dQ1*dQ6*m6*t3*t7*t11*t34*2.0;
t1058 = t34*t444;
t1059 = t34*t445;
t1060 = Lxcm6*Lycm6*dQ1*dQ5*m6*t2*t8*t10*t36*4.0;
t1061 = Lxcm6*Lycm6*dQ1*dQ5*m6*t3*t7*t10*t36*4.0;
t1062 = Lxcm6*Lycm6*dQ2*dQ5*m6*t4*t9*t10*t36*4.0;
t1063 = Lxcm6*Lycm6*dQ3*dQ5*m6*t4*t9*t10*t36*4.0;
t1065 = Lxcm6*Lycm6*dQ4*dQ6*m6*t5*t9*t10*t36*4.0;
t1066 = Lx4*Lz6*dQ1*dQ4*m6*t2*t8*t10*t34*4.0;
t1067 = Lx4*Lz6*dQ1*dQ4*m6*t3*t7*t10*t34*4.0;
t1068 = Lx4*Lzcm5*dQ1*dQ4*m5*t2*t8*t10*t34*4.0;
t1069 = Lx4*Lzcm5*dQ1*dQ4*m5*t3*t7*t10*t34*4.0;
t1070 = Lx4*Lzcm6*dQ1*dQ4*m6*t2*t8*t10*t34*4.0;
t1071 = Lx4*Lzcm6*dQ1*dQ4*m6*t3*t7*t10*t34*4.0;
t1074 = Lxcm5*Lzcm5*dQ1*dQ4*m5*t4*t7*t8*t35*4.0;
t1077 = t36*t317*2.0;
t1078 = t36*t318*2.0;
t1079 = Lz6*Lzcm6*dQ1*dQ5*m6*t7*t8*t9*t35*4.0;
t1090 = dQ1*dQ4*m6*t2*t8*t18*t34*-2.0;
t1091 = dQ1*dQ4*m6*t3*t7*t18*t34*-2.0;
t1092 = dQ1*dQ4*m6*t2*t8*t18*t36*-2.0;
t1093 = dQ1*dQ4*m6*t3*t7*t18*t36*-2.0;
t1102 = dQ5*dQ6*m6*t5*t9*t18*t36*-2.0;
t1103 = dQ1*dQ4*m4*t2*t8*t19*t34*-2.0;
t1104 = dQ1*dQ4*m4*t3*t7*t19*t34*-2.0;
t1105 = dQ1*dQ4*m5*t2*t8*t20*t34*-2.0;
t1106 = dQ1*dQ4*m5*t3*t7*t20*t34*-2.0;
t1114 = dQ4*dQ6*m6*t4*t10*t21*t36*-2.0;
t1198 = Lxcm6*Lycm6*dQ2*dQ4*m6*t5*t34*t36*8.0;
t1199 = Lxcm6*Lycm6*dQ3*dQ4*m6*t5*t34*t36*8.0;
t1202 = t34*t36*t84*-2.0;
t1203 = t34*t36*t85*-2.0;
t1206 = Iyy6*dQ2*dQ4*t4*t9*t35*t36*-2.0;
t1207 = Iyy6*dQ3*dQ4*t4*t9*t35*t36*-2.0;
t1208 = Iyy6*dQ2*dQ5*t5*t10*t34*t36*-2.0;
t1209 = Iyy6*dQ3*dQ5*t5*t10*t34*t36*-2.0;
t1210 = Iyy6*dQ2*dQ6*t6*t11*t34*t35*-2.0;
t1211 = Iyy6*dQ3*dQ6*t6*t11*t34*t35*-2.0;
t1212 = Lycm6*Lz6*dQ2*dQ5*m6*t11*t34*t35*-4.0;
t1213 = Lycm6*Lz6*dQ3*dQ5*m6*t11*t34*t35*-4.0;
t1214 = Lycm6*Lzcm6*dQ2*dQ5*m6*t11*t34*t35*-4.0;
t1215 = Lycm6*Lzcm6*dQ3*dQ5*m6*t11*t34*t35*-4.0;
t1220 = Lycm6*Lz6*dQ2*dQ6*m6*t5*t6*t10*t34*-2.0;
t1221 = Lycm6*Lz6*dQ3*dQ6*m6*t5*t6*t10*t34*-2.0;
t1222 = Lycm6*Lzcm6*dQ2*dQ6*m6*t5*t6*t10*t34*-2.0;
t1223 = Lycm6*Lzcm6*dQ3*dQ6*m6*t5*t6*t10*t34*-2.0;
t1227 = Lxcm5*Lycm5*dQ1*dQ5*m5*t2*t8*t10*t34*-2.0;
t1228 = Lxcm5*Lycm5*dQ1*dQ5*m5*t3*t7*t10*t34*-2.0;
t1229 = Lxcm6*Lycm6*dQ4*dQ5*m6*t6*t9*t11*t35*-4.0;
t1231 = Lxcm6*Lz6*dQ2*dQ6*m6*t5*t10*t11*t34*-2.0;
t1232 = Lxcm6*Lz6*dQ3*dQ6*m6*t5*t10*t11*t34*-2.0;
t1233 = Lxcm6*Lzcm6*dQ2*dQ6*m6*t5*t10*t11*t34*-2.0;
t1234 = Lxcm6*Lzcm6*dQ3*dQ6*m6*t5*t10*t11*t34*-2.0;
t1235 = t35*t594;
t1236 = dQ1*dQ5*m6*t2*t3*t9*t18*t36*2.0;
t1239 = t36*t595;
t1240 = t36*t596;
t1241 = dQ2*dQ4*m6*t5*t6*t11*t18*t34*4.0;
t1242 = dQ2*dQ6*m6*t4*t5*t9*t18*t36*4.0;
t1243 = dQ3*dQ4*m6*t5*t6*t11*t18*t34*4.0;
t1244 = dQ3*dQ6*m6*t4*t5*t9*t18*t36*4.0;
t1245 = t35*t602;
t1246 = t36*t602;
t1247 = dQ1*dQ6*m6*t2*t5*t8*t21*t34*2.0;
t1248 = dQ1*dQ6*m6*t3*t5*t7*t21*t34*2.0;
t1249 = dQ1*dQ6*m6*t2*t5*t8*t21*t36*2.0;
t1250 = dQ1*dQ6*m6*t3*t5*t7*t21*t36*2.0;
t1251 = dQ2*dQ4*m6*t5*t6*t11*t21*t34*4.0;
t1252 = dQ2*dQ6*m6*t4*t5*t9*t21*t36*4.0;
t1253 = dQ3*dQ4*m6*t5*t6*t11*t21*t34*4.0;
t1254 = dQ3*dQ6*m6*t4*t5*t9*t21*t36*4.0;
t1255 = dQ1*dQ5*m6*t2*t3*t9*t22*t35*2.0;
t1256 = dQ1*dQ5*m5*t2*t3*t9*t25*t35*2.0;
t1257 = dQ1*dQ5*m6*t2*t3*t9*t26*t35*2.0;
t1260 = dQ1*dQ5*m6*t7*t8*t9*t18*t36*2.0;
t1261 = t35*t612;
t1263 = dQ1*dQ5*m6*t7*t8*t9*t22*t35*2.0;
t1264 = dQ1*dQ5*m5*t7*t8*t9*t25*t35*2.0;
t1265 = dQ1*dQ5*m6*t7*t8*t9*t26*t35*2.0;
t1266 = -t1080;
t1267 = -t1081;
t1268 = -t1089;
t1269 = -t1116;
t1270 = -t1117;
t1271 = -t1118;
t1272 = -t1119;
t1273 = -t1120;
t1274 = -t1121;
t1275 = -t1122;
t1276 = -t1123;
t1277 = -t1124;
t1280 = -t1138;
t1281 = -t1139;
t1282 = -t1141;
t1283 = -t1142;
t1284 = -t1145;
t1285 = -t1146;
t1286 = -t1148;
t1287 = -t1149;
t1293 = -t1157;
t1294 = -t1158;
t1295 = -t1159;
t1296 = -t1160;
t1297 = -t1161;
t1298 = -t1162;
t1299 = -t1163;
t1300 = -t1164;
t1301 = -t1165;
t1302 = -t1166;
t1303 = -t1167;
t1304 = -t1168;
t1305 = -t1169;
t1306 = -t1170;
t1307 = -t1171;
t1308 = -t1172;
t1309 = -t1173;
t1310 = -t1176;
t1311 = -t1179;
t1312 = -t1180;
t1313 = -t1181;
t1314 = -t1184;
t1315 = -t1191;
t1316 = -t1192;
t1317 = -t1193;
t1318 = -t1194;
t1319 = -t1195;
t1335 = -t1196;
t1338 = Lxcm6*Lz6*dQ1*dQ4*m6*t2*t3*t4*t6*t35*4.0;
t1339 = Lxcm6*Lzcm6*dQ1*dQ4*m6*t2*t3*t4*t6*t35*4.0;
t1340 = Ixx6*dQ1*dQ4*t2*t3*t4*t5*t10*t36*2.0;
t1341 = t36*t653;
t1342 = Lx4*Lxcm6*dQ1*dQ4*m6*t2*t5*t6*t8*t34*4.0;
t1343 = Lx4*Lxcm6*dQ1*dQ4*m6*t3*t5*t6*t7*t34*4.0;
t1344 = t34*t664;
t1345 = t34*t665;
t1346 = Lycm6*Lz6*dQ1*dQ4*m6*t2*t3*t4*t11*t35*4.0;
t1347 = Lycm6*Lz6*dQ1*dQ6*m6*t2*t3*t6*t9*t35*2.0;
t1348 = t34*t670;
t1349 = t34*t671;
t1350 = Lycm6*Lzcm6*dQ1*dQ4*m6*t2*t3*t4*t11*t35*4.0;
t1351 = Lycm6*Lzcm6*dQ1*dQ6*m6*t2*t3*t6*t9*t35*2.0;
t1352 = dQ4*dQ5*m6*t9*t21*t35*t36*-2.0;
t1353 = Lx4*Lycm6*dQ1*dQ4*m6*t2*t5*t8*t11*t34*4.0;
t1354 = Lx4*Lycm6*dQ1*dQ4*m6*t3*t5*t7*t11*t34*4.0;
t1355 = t35*t692;
t1356 = t35*t693;
t1357 = Lxcm6*Lycm6*dQ1*dQ4*m6*t2*t3*t9*t10*t36*4.0;
t1360 = Lxcm6*Lycm6*dQ1*dQ6*m6*t2*t4*t8*t9*t36*4.0;
t1361 = Lxcm6*Lycm6*dQ1*dQ6*m6*t3*t4*t7*t9*t36*4.0;
t1362 = t35*t696;
t1363 = t35*t697;
t1364 = t34*t698;
t1365 = t34*t699;
t1366 = t34*t718;
t1367 = t34*t719;
t1368 = Lxcm6*Lz6*dQ1*dQ4*m6*t4*t6*t7*t8*t35*4.0;
t1369 = Lxcm6*Lz6*dQ1*dQ6*m6*t2*t3*t9*t11*t35*2.0;
t1370 = Lxcm6*Lz6*dQ1*dQ6*m6*t2*t6*t8*t10*t34*2.0;
t1371 = Lxcm6*Lz6*dQ1*dQ6*m6*t3*t6*t7*t10*t34*2.0;
t1372 = Lxcm5*Lzcm5*dQ1*dQ4*m5*t2*t5*t8*t10*t34*4.0;
t1373 = Lxcm5*Lzcm5*dQ1*dQ4*m5*t3*t5*t7*t10*t34*4.0;
t1374 = Lxcm5*Lzcm5*dQ1*dQ5*m5*t2*t4*t8*t9*t35*4.0;
t1375 = Lxcm5*Lzcm5*dQ1*dQ5*m5*t3*t4*t7*t9*t35*4.0;
t1376 = t34*t728;
t1377 = t34*t729;
t1378 = Lxcm6*Lzcm6*dQ1*dQ4*m6*t4*t6*t7*t8*t35*4.0;
t1379 = Lxcm6*Lzcm6*dQ1*dQ6*m6*t2*t3*t9*t11*t35*2.0;
t1380 = Lxcm6*Lzcm6*dQ1*dQ6*m6*t2*t6*t8*t10*t34*2.0;
t1381 = Lxcm6*Lzcm6*dQ1*dQ6*m6*t3*t6*t7*t10*t34*2.0;
t1382 = Ixx6*dQ1*dQ4*t4*t5*t7*t8*t10*t36*2.0;
t1383 = t34*t738;
t1384 = t34*t739;
t1388 = Lycm6*Lz6*dQ1*dQ4*m6*t4*t7*t8*t11*t35*4.0;
t1389 = Lycm6*Lz6*dQ1*dQ6*m6*t2*t8*t10*t11*t34*2.0;
t1390 = Lycm6*Lz6*dQ1*dQ6*m6*t3*t7*t10*t11*t34*2.0;
t1391 = Lycm6*Lz6*dQ1*dQ6*m6*t6*t7*t8*t9*t35*2.0;
t1392 = Lycm6*Lzcm6*dQ1*dQ4*m6*t4*t7*t8*t11*t35*4.0;
t1393 = Lycm6*Lzcm6*dQ1*dQ6*m6*t2*t8*t10*t11*t34*2.0;
t1394 = Lycm6*Lzcm6*dQ1*dQ6*m6*t3*t7*t10*t11*t34*2.0;
t1395 = Lycm6*Lzcm6*dQ1*dQ6*m6*t6*t7*t8*t9*t35*2.0;
t1396 = Lxcm6*Lycm6*dQ1*dQ4*m6*t7*t8*t9*t10*t36*4.0;
t1397 = Lxcm6*Lz6*dQ1*dQ6*m6*t7*t8*t9*t11*t35*2.0;
t1398 = Lxcm6*Lzcm6*dQ1*dQ6*m6*t7*t8*t9*t11*t35*2.0;
t1402 = dQ1*dQ6*m6*t2*t5*t8*t18*t34*-2.0;
t1403 = dQ1*dQ6*m6*t3*t5*t7*t18*t34*-2.0;
t1404 = dQ1*dQ6*m6*t2*t5*t8*t18*t36*-2.0;
t1405 = dQ1*dQ6*m6*t3*t5*t7*t18*t36*-2.0;
t1418 = t4*t5*t6*t9*t11*t84*4.0;
t1419 = t4*t5*t6*t9*t11*t85*4.0;
t1421 = t4*t5*t6*t9*t11*t92*4.0;
t1422 = t4*t5*t6*t9*t11*t93*4.0;
t1436 = dQ1*dQ5*m5*t7*t8*t9*t17*t35*-2.0;
t1437 = dQ1*dQ5*m6*t7*t8*t9*t21*t35*-2.0;
t1438 = dQ1*dQ5*m6*t7*t8*t9*t21*t36*-2.0;
t1453 = t34*t36*t149*4.0;
t1454 = t34*t36*t150*4.0;
t1456 = t34*t36*t153*4.0;
t1457 = t34*t36*t154*4.0;
t1460 = -t1290;
t1461 = -t1291;
t1462 = -t1292;
t1465 = -t1320;
t1466 = -t1325;
t1467 = -t1326;
t1468 = -t1327;
t1469 = -t1328;
t1470 = -t1329;
t1471 = -t1330;
t1478 = Lxcm6*Lycm6*dQ1*dQ4*m6*t2*t6*t8*t11*t34*-4.0;
t1479 = Lxcm6*Lycm6*dQ1*dQ4*m6*t3*t6*t7*t11*t34*-4.0;
t1482 = dQ1*dQ6*m6*t2*t3*t4*t10*t18*t36*2.0;
t1484 = Iyy6*dQ1*dQ4*t4*t5*t7*t8*t10*t36*-2.0;
t1485 = Iyy6*dQ1*dQ5*t2*t6*t8*t10*t11*t34*-2.0;
t1486 = Iyy6*dQ1*dQ5*t3*t6*t7*t10*t11*t34*-2.0;
t1497 = dQ1*dQ6*m6*t4*t7*t8*t10*t18*t36*2.0;
t1498 = t36*t908;
t1499 = Lxcm6*Lycm6*dQ2*dQ6*m6*t34*t35*t36*-4.0;
t1500 = Lxcm6*Lycm6*dQ3*dQ6*m6*t34*t35*t36*-4.0;
t1501 = -t1413;
t1502 = -t1414;
t1503 = -t1415;
t1506 = -t1423;
t1507 = -t1424;
t1508 = -t1425;
t1509 = -t1426;
t1510 = -t1427;
t1511 = -t1428;
t1512 = -t1429;
t1513 = -t1430;
t1514 = -t1431;
t1515 = -t1432;
t1516 = -t1433;
t1517 = -t1442;
t1518 = -t1443;
t1519 = -t1444;
t1520 = -t1445;
t1521 = -t1446;
t1522 = -t1447;
t1539 = -t1448;
t1540 = t35*t36*t148*-2.0;
t1545 = Lz6*Lzcm6*dQ1*dQ4*m6*t2*t8*t34*t35*-4.0;
t1546 = Lz6*Lzcm6*dQ1*dQ4*m6*t3*t7*t34*t35*-4.0;
t1547 = dQ1*dQ4*m5*t2*t8*t17*t34*t35*2.0;
t1548 = dQ1*dQ4*m5*t3*t7*t17*t34*t35*2.0;
t1557 = dQ1*dQ4*m6*t2*t8*t21*t34*t35*2.0;
t1558 = dQ1*dQ4*m6*t3*t7*t21*t34*t35*2.0;
t1573 = t35*t36*t162*-2.0;
t1574 = t35*t1192;
t1575 = Lxcm6*Lycm6*dQ1*dQ6*m6*t5*t7*t8*t9*t10*t36*4.0;
t1580 = dQ1*dQ6*m6*t2*t3*t4*t10*t21*t36*-2.0;
t1594 = -t1523;
t1595 = -t1524;
t1596 = -t1525;
t1597 = -t1526;
t1598 = -t1527;
t1599 = -t1528;
t1600 = -t1529;
t1601 = -t1544;
t1602 = dQ2*dQ4*m6*t4*t9*t18*t35*t36*-2.0;
t1603 = dQ3*dQ4*m6*t4*t9*t18*t35*t36*-2.0;
t1604 = dQ2*dQ5*m6*t5*t10*t18*t34*t36*-2.0;
t1605 = dQ3*dQ5*m6*t5*t10*t18*t34*t36*-2.0;
t1606 = dQ2*dQ6*m6*t6*t11*t18*t34*t35*-2.0;
t1607 = dQ3*dQ6*m6*t6*t11*t18*t34*t35*-2.0;
t1608 = dQ1*dQ4*m6*t2*t8*t21*t34*t36*-2.0;
t1609 = dQ1*dQ4*m6*t3*t7*t21*t34*t36*-2.0;
t1610 = dQ1*dQ4*m6*t2*t8*t22*t34*t35*-2.0;
t1611 = dQ1*dQ4*m6*t3*t7*t22*t34*t35*-2.0;
t1612 = dQ1*dQ4*m5*t2*t8*t25*t34*t35*-2.0;
t1613 = dQ1*dQ4*m5*t3*t7*t25*t34*t35*-2.0;
t1614 = dQ1*dQ4*m6*t2*t8*t26*t34*t35*-2.0;
t1615 = dQ1*dQ4*m6*t3*t7*t26*t34*t35*-2.0;
t1617 = Lxcm6*Lycm6*dQ1*dQ6*m6*t2*t3*t5*t9*t10*t36*4.0;
t1618 = Lxcm6*Lz6*dQ1*dQ4*m6*t2*t5*t6*t8*t10*t34*4.0;
t1619 = Lxcm6*Lz6*dQ1*dQ4*m6*t3*t5*t6*t7*t10*t34*4.0;
t1620 = Lxcm6*Lz6*dQ1*dQ5*m6*t2*t4*t6*t8*t9*t35*4.0;
t1621 = Lxcm6*Lz6*dQ1*dQ5*m6*t3*t4*t6*t7*t9*t35*4.0;
t1622 = Lxcm6*Lzcm6*dQ1*dQ4*m6*t2*t5*t6*t8*t10*t34*4.0;
t1623 = Lxcm6*Lzcm6*dQ1*dQ4*m6*t3*t5*t6*t7*t10*t34*4.0;
t1624 = Lxcm6*Lzcm6*dQ1*dQ5*m6*t2*t4*t6*t8*t9*t35*4.0;
t1625 = Lxcm6*Lzcm6*dQ1*dQ5*m6*t3*t4*t6*t7*t9*t35*4.0;
t1626 = Ixx6*dQ1*dQ5*t2*t4*t5*t8*t9*t10*t36*2.0;
t1627 = Ixx6*dQ1*dQ5*t3*t4*t5*t7*t9*t10*t36*2.0;
t1628 = t35*t1153;
t1629 = t35*t1154;
t1634 = Lycm6*Lz6*dQ1*dQ4*m6*t2*t5*t8*t10*t11*t34*4.0;
t1635 = Lycm6*Lz6*dQ1*dQ4*m6*t3*t5*t7*t10*t11*t34*4.0;
t1636 = Lycm6*Lz6*dQ1*dQ5*m6*t2*t4*t8*t9*t11*t35*4.0;
t1637 = Lycm6*Lz6*dQ1*dQ5*m6*t3*t4*t7*t9*t11*t35*4.0;
t1638 = Lycm6*Lzcm6*dQ1*dQ4*m6*t2*t5*t8*t10*t11*t34*4.0;
t1639 = Lycm6*Lzcm6*dQ1*dQ4*m6*t3*t5*t7*t10*t11*t34*4.0;
t1640 = Lycm6*Lzcm6*dQ1*dQ5*m6*t2*t4*t8*t9*t11*t35*4.0;
t1641 = Lycm6*Lzcm6*dQ1*dQ5*m6*t3*t4*t7*t9*t11*t35*4.0;
t1642 = dQ1*dQ4*m6*t4*t5*t7*t8*t10*t18*t36*2.0;
t1645 = t36*t1326;
t1646 = t34*t1327;
t1647 = t34*t1328;
t1650 = -t1581;
t1651 = -t1582;
t1652 = -t1583;
t1653 = -t1584;
t1654 = -t1585;
t1655 = -t1588;
t1656 = -t1589;
t1657 = -t1590;
t1658 = -t1591;
t1667 = Lxcm6*Lycm6*dQ1*dQ5*m6*t2*t8*t10*t34*t36*-4.0;
t1668 = Lxcm6*Lycm6*dQ1*dQ5*m6*t3*t7*t10*t34*t36*-4.0;
t1670 = dQ1*dQ6*m6*t2*t5*t8*t18*t34*t36*4.0;
t1671 = dQ1*dQ6*m6*t3*t5*t7*t18*t34*t36*4.0;
t1673 = dQ1*dQ6*m6*t2*t5*t8*t21*t34*t36*4.0;
t1674 = dQ1*dQ6*m6*t3*t5*t7*t21*t34*t36*4.0;
t1677 = Lxcm6*Lycm6*dQ1*dQ5*m6*t2*t3*t6*t9*t11*t35*-4.0;
t1679 = Lxcm6*Lycm6*dQ1*dQ4*m6*t2*t4*t5*t8*t9*t36*8.0;
t1680 = Lxcm6*Lycm6*dQ1*dQ4*m6*t3*t4*t5*t7*t9*t36*8.0;
t1681 = Lxcm6*Lycm6*dQ1*dQ6*m6*t2*t5*t6*t8*t11*t34*8.0;
t1682 = Lxcm6*Lycm6*dQ1*dQ6*m6*t3*t5*t6*t7*t11*t34*8.0;
t1683 = dQ1*dQ4*m6*t2*t3*t4*t5*t10*t18*t36*2.0;
t1685 = Iyy6*dQ1*dQ5*t2*t4*t5*t8*t9*t10*t36*-2.0;
t1686 = Iyy6*dQ1*dQ5*t3*t4*t5*t7*t9*t10*t36*-2.0;
t1687 = Iyy6*dQ1*dQ6*t2*t4*t6*t8*t9*t11*t35*-2.0;
t1688 = Iyy6*dQ1*dQ6*t3*t4*t6*t7*t9*t11*t35*-2.0;
t1698 = dQ1*dQ5*m6*t2*t6*t8*t10*t11*t18*t34*-2.0;
t1699 = dQ1*dQ5*m6*t3*t6*t7*t10*t11*t18*t34*-2.0;
t1706 = -t1659;
t1707 = -t1660;
t1708 = -t1661;
t1709 = -t1666;
t1710 = dQ1*dQ5*m6*t2*t3*t9*t21*t35*t36*-2.0;
t1713 = dQ1*dQ5*m6*t7*t8*t9*t18*t35*t36*-2.0;
t1718 = dQ1*dQ4*m6*t2*t3*t4*t5*t10*t21*t36*-2.0;
t1721 = Lxcm6*Lycm6*dQ1*dQ6*m6*t2*t4*t8*t9*t35*t36*-4.0;
t1722 = Lxcm6*Lycm6*dQ1*dQ6*m6*t3*t4*t7*t9*t35*t36*-4.0;
t1723 = dQ1*dQ5*m6*t2*t4*t5*t8*t9*t10*t18*t36*2.0;
t1724 = dQ1*dQ5*m6*t3*t4*t5*t7*t9*t10*t18*t36*2.0;
t1727 = t36*t1528;
t1728 = t36*t1529;
t1729 = t35*t1531;
t1730 = t35*t1532;
t1737 = dQ1*dQ6*m6*t2*t4*t6*t8*t9*t11*t18*t35*-2.0;
t1738 = dQ1*dQ6*m6*t3*t4*t6*t7*t9*t11*t18*t35*-2.0;
t137 = -t62;
t138 = -t63;
t139 = -t64;
t140 = -t65;
t141 = -t66;
t142 = -t67;
t143 = -t68;
t144 = -t69;
t145 = -t70;
t146 = -t71;
t293 = -t193;
t294 = -t194;
t295 = -t195;
t296 = -t196;
t297 = -t197;
t298 = -t198;
t299 = -t200;
t300 = -t202;
t303 = -t205;
t304 = -t206;
t305 = -t207;
t306 = -t209;
t307 = -t210;
t308 = -t213;
t309 = -t214;
t310 = -t215;
t311 = -t216;
t312 = -t217;
t313 = -t218;
t412 = -t219;
t413 = -t220;
t414 = -t221;
t415 = -t222;
t416 = -t223;
t417 = -t224;
t418 = -t225;
t419 = -t226;
t420 = -t237;
t421 = -t238;
t422 = -t239;
t423 = -t240;
t424 = -t241;
t425 = -t242;
t426 = -t243;
t427 = -t244;
t428 = -t245;
t429 = -t246;
t430 = -t247;
t431 = -t248;
t542 = -t359;
t543 = -t360;
t544 = -t361;
t545 = -t362;
t546 = -t367;
t547 = -t368;
t548 = -t373;
t613 = -t467;
t614 = -t468;
t615 = -t469;
t616 = -t470;
t617 = -t475;
t620 = -t484;
t621 = -t485;
t624 = -t488;
t625 = -t489;
t626 = -t490;
t627 = -t491;
t628 = -t502;
t629 = -t504;
t630 = -t505;
t631 = -t507;
t632 = -t508;
t633 = -t514;
t634 = -t515;
t635 = -t517;
t636 = -t520;
t637 = -t523;
t638 = -t526;
t639 = -t529;
t640 = -t530;
t641 = -t531;
t642 = -t532;
t643 = -t533;
t644 = -t534;
t645 = -t535;
t646 = -t536;
t647 = -t537;
t648 = -t538;
t649 = -t539;
t650 = -t540;
t651 = -t541;
t674 = -t550;
t675 = -t553;
t676 = -t554;
t677 = -t555;
t767 = t35*t199;
t768 = t35*t201;
out1 = ft_3({Ixx2,Ixx3,Ixx4,Ixx5,Ixx6,Iyy4,Iyy5,Iyy6,Izz2,Izz3,Izz4,Izz5,Izz6,Lx2,Lx3,Lx4,Lxcm2,Lxcm3,Lxcm4,Lxcm5,Lxcm6,Lycm3,Lycm4,Lycm5,Lycm6,Lz6,Lzcm2,Lzcm3,Lzcm4,Lzcm5,Lzcm6,dQ1,dQ2,dQ3,dQ4,dQ5,dQ6,m2,m3,m4,m5,m6,t10,t100,t1000,t1004,t1005,t1006,t101,t1011,t1012,t102,t1021,t1022,t103,t1039,t1040,t1041,t1042,t1043,t1044,t1045,t1046,t1049,t1050,t1053,t1054,t1055,t1058,t1059,t1060,t1061,t1062,t1063,t1065,t1066,t1067,t1068,t1069,t1070,t1071,t1074,t1077,t1078,t1079,t108,t1082,t1083,t1084,t1085,t1086,t1087,t1088,t109,t1090,t1091,t1092,t1093,t11,t110,t1102,t1103,t1104,t1105,t1106,t111,t1114,t112,t1125,t1126,t1127,t1128,t1129,t113,t1130,t1131,t1132,t1133,t1134,t1135,t1136,t1137,t114,t1140,t1143,t1144,t1147,t115,t1150,t1151,t1152,t1153,t1154,t1155,t1156,t116,t117,t1174,t1175,t1177,t1178,t118,t1182,t1183,t1185,t1186,t1187,t1188,t1189,t1190,t1197,t1198,t1199,t12,t1202,t1203,t1206,t1207,t1208,t1209,t1210,t1211,t1212,t1213,t1214,t1215,t1220,t1221,t1222,t1223,t1227,t1228,t1229,t1231,t1232,t1233,t1234,t1235,t1236,t1239,t1240,t1241,t1242,t1243,t1244,t1245,t1246,t1247,t1248,t1249,t1250,t1251,t1252,t1253,t1254,t1255,t1256,t1257,t1260,t1261,t1263,t1264,t1265,t1266,t1267,t1268,t1269,t127,t1270,t1271,t1272,t1273,t1274,t1275,t1276,t1277,t1278,t1279,t128,t1280,t1281,t1282,t1283,t1284,t1285,t1286,t1287,t1288,t1289,t129,t1293,t1294,t1295,t1296,t1297,t1298,t1299,t13,t130,t1300,t1301,t1302,t1303,t1304,t1305,t1306,t1307,t1308,t1309,t131,t1310,t1311,t1312,t1313,t1314,t1315,t1316,t1317,t1318,t1319,t132,t1321,t1322,t1323,t1324,t133,t1331,t1332,t1333,t1334,t1335,t1338,t1339,t134,t1340,t1341,t1342,t1343,t1344,t1345,t1346,t1347,t1348,t1349,t1350,t1351,t1352,t1353,t1354,t1355,t1356,t1357,t1360,t1361,t1362,t1363,t1364,t1365,t1366,t1367,t1368,t1369,t137,t1370,t1371,t1372,t1373,t1374,t1375,t1376,t1377,t1378,t1379,t138,t1380,t1381,t1382,t1383,t1384,t1388,t1389,t139,t1390,t1391,t1392,t1393,t1394,t1395,t1396,t1397,t1398,t14,t140,t1402,t1403,t1404,t1405,t141,t1416,t1417,t1418,t1419,t142,t1420,t1421,t1422,t143,t1434,t1435,t1436,t1437,t1438,t1439,t144,t1440,t1441,t1449,t145,t1450,t1451,t1453,t1454,t1456,t1457,t146,t1460,t1461,t1462,t1465,t1466,t1467,t1468,t1469,t147,t1470,t1471,t1478,t1479,t148,t1482,t1484,t1485,t1486,t149,t1497,t1498,t1499,t15,t150,t1500,t1501,t1502,t1503,t1506,t1507,t1508,t1509,t1510,t1511,t1512,t1513,t1514,t1515,t1516,t1517,t1518,t1519,t152,t1520,t1521,t1522,t153,t1530,t1531,t1532,t1533,t1534,t1535,t1536,t1537,t1538,t1539,t154,t1540,t1543,t1545,t1546,t1547,t1548,t1557,t1558,t157,t1573,t1574,t1575,t158,t1580,t1587,t1594,t1595,t1596,t1597,t1598,t1599,t16,t160,t1600,t1601,t1602,t1603,t1604,t1605,t1606,t1607,t1608,t1609,t161,t1610,t1611,t1612,t1613,t1614,t1615,t1617,t1618,t1619,t1620,t1621,t1622,t1623,t1624,t1625,t1626,t1627,t1628,t1629,t163,t1634,t1635,t1636,t1637,t1638,t1639,t164,t1640,t1641,t1642,t1645,t1646,t1647,t165,t1650,t1651,t1652,t1653,t1654,t1655,t1656,t1657,t1658,t166,t1662,t1663,t1664,t1665,t1667,t1668,t167,t1670,t1671,t1673,t1674,t1677,t1679,t168,t1680,t1681,t1682,t1683,t1685,t1686,t1687,t1688,t169,t1698,t1699,t17,t170,t1700,t1701,t1706,t1707,t1708,t1709,t171,t1710,t1713,t1718,t172,t1721,t1722,t1723,t1724,t1727,t1728,t1729,t173,t1730,t1737,t1738,t174,t175,t176,t177,t178,t179,t18,t180,t181,t182,t183,t184,t185,t186,t187,t188,t189,t19,t190,t191,t192,t199,t2,t20,t200,t201,t202,t205,t206,t208,t209,t21,t211,t212,t22,t227,t228,t229,t23,t230,t231,t232,t233,t234,t235,t236,t24,t25,t252,t253,t254,t255,t256,t257,t26,t260,t261,t262,t263,t264,t265,t266,t277,t278,t279,t280,t281,t282,t289,t290,t291,t292,t293,t294,t295,t296,t297,t298,t299,t3,t300,t301,t302,t303,t304,t305,t306,t307,t308,t309,t310,t311,t312,t313,t314,t316,t318,t32,t320,t321,t322,t323,t324,t325,t326,t327,t328,t329,t33,t330,t331,t332,t333,t334,t335,t336,t337,t338,t339,t34,t340,t341,t342,t343,t344,t345,t346,t347,t348,t349,t35,t350,t351,t352,t353,t354,t355,t356,t357,t358,t36,t363,t364,t365,t366,t369,t37,t370,t371,t372,t38,t380,t382,t383,t384,t385,t386,t387,t388,t389,t39,t4,t40,t401,t402,t403,t404,t409,t41,t410,t411,t412,t413,t414,t415,t416,t417,t418,t419,t42,t420,t421,t422,t423,t424,t425,t426,t427,t428,t429,t430,t431,t436,t437,t438,t439,t440,t441,t442,t443,t446,t447,t45,t450,t451,t454,t459,t460,t461,t463,t464,t465,t471,t472,t473,t474,t476,t477,t478,t479,t48,t480,t481,t484,t485,t488,t489,t49,t492,t493,t494,t495,t496,t497,t498,t499,t5,t50,t500,t501,t502,t503,t504,t505,t506,t508,t509,t51,t510,t511,t512,t513,t514,t515,t516,t518,t519,t52,t521,t522,t524,t525,t527,t528,t53,t530,t531,t532,t533,t54,t542,t543,t544,t545,t546,t547,t548,t549,t55,t550,t551,t552,t556,t557,t558,t559,t56,t560,t561,t562,t563,t564,t565,t566,t567,t568,t569,t57,t570,t571,t572,t573,t574,t575,t576,t577,t578,t579,t58,t580,t581,t582,t583,t584,t585,t586,t587,t588,t589,t59,t590,t591,t592,t593,t595,t596,t597,t598,t599,t6,t60,t600,t605,t606,t607,t608,t609,t61,t610,t611,t612,t613,t614,t615,t616,t617,t618,t619,t620,t621,t622,t623,t624,t625,t626,t627,t628,t629,t630,t631,t632,t633,t634,t635,t636,t637,t638,t639,t640,t641,t642,t643,t644,t645,t646,t647,t648,t649,t650,t651,t654,t655,t656,t657,t658,t659,t660,t668,t674,t675,t676,t677,t686,t687,t691,t692,t693,t694,t695,t696,t697,t698,t699,t7,t701,t702,t703,t704,t705,t706,t707,t708,t709,t710,t711,t712,t713,t714,t715,t716,t72,t724,t73,t736,t737,t74,t742,t743,t744,t745,t746,t747,t75,t756,t757,t758,t76,t761,t762,t763,t765,t767,t768,t769,t77,t770,t771,t772,t777,t778,t779,t78,t780,t781,t782,t783,t784,t785,t786,t787,t788,t789,t79,t790,t791,t792,t793,t794,t795,t796,t797,t798,t799,t8,t80,t800,t801,t802,t803,t804,t805,t806,t807,t808,t809,t81,t810,t811,t812,t813,t814,t815,t816,t817,t818,t819,t82,t820,t821,t822,t823,t824,t825,t826,t827,t828,t829,t83,t830,t831,t832,t833,t834,t835,t836,t837,t838,t839,t84,t843,t844,t845,t846,t847,t848,t849,t85,t850,t851,t852,t853,t854,t855,t856,t857,t858,t859,t86,t860,t861,t862,t863,t864,t865,t866,t867,t868,t869,t870,t871,t872,t873,t874,t875,t876,t877,t878,t879,t88,t880,t881,t882,t883,t884,t885,t886,t887,t888,t889,t890,t891,t892,t893,t894,t895,t896,t897,t898,t899,t9,t90,t900,t901,t902,t903,t904,t905,t906,t907,t91,t911,t92,t93,t937,t938,t939,t94,t940,t941,t942,t943,t944,t945,t946,t947,t948,t949,t95,t950,t951,t952,t953,t954,t955,t956,t957,t958,t959,t96,t960,t961,t967,t968,t969,t97,t970,t971,t972,t973,t974,t975,t976,t977,t978,t979,t98,t981,t982,t983,t984,t985,t986,t987,t988,t989,t99,t990,t991,t992,t993,t994,t995,t996,t997,t998,t999});
end
function out1 = ft_3(ct)
[Ixx2,Ixx3,Ixx4,Ixx5,Ixx6,Iyy4,Iyy5,Iyy6,Izz2,Izz3,Izz4,Izz5,Izz6,Lx2,Lx3,Lx4,Lxcm2,Lxcm3,Lxcm4,Lxcm5,Lxcm6,Lycm3,Lycm4,Lycm5,Lycm6,Lz6,Lzcm2,Lzcm3,Lzcm4,Lzcm5,Lzcm6,dQ1,dQ2,dQ3,dQ4,dQ5,dQ6,m2,m3,m4,m5,m6,t10,t100,t1000,t1004,t1005,t1006,t101,t1011,t1012,t102,t1021,t1022,t103,t1039,t1040,t1041,t1042,t1043,t1044,t1045,t1046,t1049,t1050,t1053,t1054,t1055,t1058,t1059,t1060,t1061,t1062,t1063,t1065,t1066,t1067,t1068,t1069,t1070,t1071,t1074,t1077,t1078,t1079,t108,t1082,t1083,t1084,t1085,t1086,t1087,t1088,t109,t1090,t1091,t1092,t1093,t11,t110,t1102,t1103,t1104,t1105,t1106,t111,t1114,t112,t1125,t1126,t1127,t1128,t1129,t113,t1130,t1131,t1132,t1133,t1134,t1135,t1136,t1137,t114,t1140,t1143,t1144,t1147,t115,t1150,t1151,t1152,t1153,t1154,t1155,t1156,t116,t117,t1174,t1175,t1177,t1178,t118,t1182,t1183,t1185,t1186,t1187,t1188,t1189,t1190,t1197,t1198,t1199,t12,t1202,t1203,t1206,t1207,t1208,t1209,t1210,t1211,t1212,t1213,t1214,t1215,t1220,t1221,t1222,t1223,t1227,t1228,t1229,t1231,t1232,t1233,t1234,t1235,t1236,t1239,t1240,t1241,t1242,t1243,t1244,t1245,t1246,t1247,t1248,t1249,t1250,t1251,t1252,t1253,t1254,t1255,t1256,t1257,t1260,t1261,t1263,t1264,t1265,t1266,t1267,t1268,t1269,t127,t1270,t1271,t1272,t1273,t1274,t1275,t1276,t1277,t1278,t1279,t128,t1280,t1281,t1282,t1283,t1284,t1285,t1286,t1287,t1288,t1289,t129,t1293,t1294,t1295,t1296,t1297,t1298,t1299,t13,t130,t1300,t1301,t1302,t1303,t1304,t1305,t1306,t1307,t1308,t1309,t131,t1310,t1311,t1312,t1313,t1314,t1315,t1316,t1317,t1318,t1319,t132,t1321,t1322,t1323,t1324,t133,t1331,t1332,t1333,t1334,t1335,t1338,t1339,t134,t1340,t1341,t1342,t1343,t1344,t1345,t1346,t1347,t1348,t1349,t1350,t1351,t1352,t1353,t1354,t1355,t1356,t1357,t1360,t1361,t1362,t1363,t1364,t1365,t1366,t1367,t1368,t1369,t137,t1370,t1371,t1372,t1373,t1374,t1375,t1376,t1377,t1378,t1379,t138,t1380,t1381,t1382,t1383,t1384,t1388,t1389,t139,t1390,t1391,t1392,t1393,t1394,t1395,t1396,t1397,t1398,t14,t140,t1402,t1403,t1404,t1405,t141,t1416,t1417,t1418,t1419,t142,t1420,t1421,t1422,t143,t1434,t1435,t1436,t1437,t1438,t1439,t144,t1440,t1441,t1449,t145,t1450,t1451,t1453,t1454,t1456,t1457,t146,t1460,t1461,t1462,t1465,t1466,t1467,t1468,t1469,t147,t1470,t1471,t1478,t1479,t148,t1482,t1484,t1485,t1486,t149,t1497,t1498,t1499,t15,t150,t1500,t1501,t1502,t1503,t1506,t1507,t1508,t1509,t1510,t1511,t1512,t1513,t1514,t1515,t1516,t1517,t1518,t1519,t152,t1520,t1521,t1522,t153,t1530,t1531,t1532,t1533,t1534,t1535,t1536,t1537,t1538,t1539,t154,t1540,t1543,t1545,t1546,t1547,t1548,t1557,t1558,t157,t1573,t1574,t1575,t158,t1580,t1587,t1594,t1595,t1596,t1597,t1598,t1599,t16,t160,t1600,t1601,t1602,t1603,t1604,t1605,t1606,t1607,t1608,t1609,t161,t1610,t1611,t1612,t1613,t1614,t1615,t1617,t1618,t1619,t1620,t1621,t1622,t1623,t1624,t1625,t1626,t1627,t1628,t1629,t163,t1634,t1635,t1636,t1637,t1638,t1639,t164,t1640,t1641,t1642,t1645,t1646,t1647,t165,t1650,t1651,t1652,t1653,t1654,t1655,t1656,t1657,t1658,t166,t1662,t1663,t1664,t1665,t1667,t1668,t167,t1670,t1671,t1673,t1674,t1677,t1679,t168,t1680,t1681,t1682,t1683,t1685,t1686,t1687,t1688,t169,t1698,t1699,t17,t170,t1700,t1701,t1706,t1707,t1708,t1709,t171,t1710,t1713,t1718,t172,t1721,t1722,t1723,t1724,t1727,t1728,t1729,t173,t1730,t1737,t1738,t174,t175,t176,t177,t178,t179,t18,t180,t181,t182,t183,t184,t185,t186,t187,t188,t189,t19,t190,t191,t192,t199,t2,t20,t200,t201,t202,t205,t206,t208,t209,t21,t211,t212,t22,t227,t228,t229,t23,t230,t231,t232,t233,t234,t235,t236,t24,t25,t252,t253,t254,t255,t256,t257,t26,t260,t261,t262,t263,t264,t265,t266,t277,t278,t279,t280,t281,t282,t289,t290,t291,t292,t293,t294,t295,t296,t297,t298,t299,t3,t300,t301,t302,t303,t304,t305,t306,t307,t308,t309,t310,t311,t312,t313,t314,t316,t318,t32,t320,t321,t322,t323,t324,t325,t326,t327,t328,t329,t33,t330,t331,t332,t333,t334,t335,t336,t337,t338,t339,t34,t340,t341,t342,t343,t344,t345,t346,t347,t348,t349,t35,t350,t351,t352,t353,t354,t355,t356,t357,t358,t36,t363,t364,t365,t366,t369,t37,t370,t371,t372,t38,t380,t382,t383,t384,t385,t386,t387,t388,t389,t39,t4,t40,t401,t402,t403,t404,t409,t41,t410,t411,t412,t413,t414,t415,t416,t417,t418,t419,t42,t420,t421,t422,t423,t424,t425,t426,t427,t428,t429,t430,t431,t436,t437,t438,t439,t440,t441,t442,t443,t446,t447,t45,t450,t451,t454,t459,t460,t461,t463,t464,t465,t471,t472,t473,t474,t476,t477,t478,t479,t48,t480,t481,t484,t485,t488,t489,t49,t492,t493,t494,t495,t496,t497,t498,t499,t5,t50,t500,t501,t502,t503,t504,t505,t506,t508,t509,t51,t510,t511,t512,t513,t514,t515,t516,t518,t519,t52,t521,t522,t524,t525,t527,t528,t53,t530,t531,t532,t533,t54,t542,t543,t544,t545,t546,t547,t548,t549,t55,t550,t551,t552,t556,t557,t558,t559,t56,t560,t561,t562,t563,t564,t565,t566,t567,t568,t569,t57,t570,t571,t572,t573,t574,t575,t576,t577,t578,t579,t58,t580,t581,t582,t583,t584,t585,t586,t587,t588,t589,t59,t590,t591,t592,t593,t595,t596,t597,t598,t599,t6,t60,t600,t605,t606,t607,t608,t609,t61,t610,t611,t612,t613,t614,t615,t616,t617,t618,t619,t620,t621,t622,t623,t624,t625,t626,t627,t628,t629,t630,t631,t632,t633,t634,t635,t636,t637,t638,t639,t640,t641,t642,t643,t644,t645,t646,t647,t648,t649,t650,t651,t654,t655,t656,t657,t658,t659,t660,t668,t674,t675,t676,t677,t686,t687,t691,t692,t693,t694,t695,t696,t697,t698,t699,t7,t701,t702,t703,t704,t705,t706,t707,t708,t709,t710,t711,t712,t713,t714,t715,t716,t72,t724,t73,t736,t737,t74,t742,t743,t744,t745,t746,t747,t75,t756,t757,t758,t76,t761,t762,t763,t765,t767,t768,t769,t77,t770,t771,t772,t777,t778,t779,t78,t780,t781,t782,t783,t784,t785,t786,t787,t788,t789,t79,t790,t791,t792,t793,t794,t795,t796,t797,t798,t799,t8,t80,t800,t801,t802,t803,t804,t805,t806,t807,t808,t809,t81,t810,t811,t812,t813,t814,t815,t816,t817,t818,t819,t82,t820,t821,t822,t823,t824,t825,t826,t827,t828,t829,t83,t830,t831,t832,t833,t834,t835,t836,t837,t838,t839,t84,t843,t844,t845,t846,t847,t848,t849,t85,t850,t851,t852,t853,t854,t855,t856,t857,t858,t859,t86,t860,t861,t862,t863,t864,t865,t866,t867,t868,t869,t870,t871,t872,t873,t874,t875,t876,t877,t878,t879,t88,t880,t881,t882,t883,t884,t885,t886,t887,t888,t889,t890,t891,t892,t893,t894,t895,t896,t897,t898,t899,t9,t90,t900,t901,t902,t903,t904,t905,t906,t907,t91,t911,t92,t93,t937,t938,t939,t94,t940,t941,t942,t943,t944,t945,t946,t947,t948,t949,t95,t950,t951,t952,t953,t954,t955,t956,t957,t958,t959,t96,t960,t961,t967,t968,t969,t97,t970,t971,t972,t973,t974,t975,t976,t977,t978,t979,t98,t981,t982,t983,t984,t985,t986,t987,t988,t989,t99,t990,t991,t992,t993,t994,t995,t996,t997,t998,t999] = ct{:};
t773 = t34*t205;
t774 = t34*t206;
t776 = t36*t209;
t909 = -t769;
t910 = -t771;
t912 = -t784;
t913 = -t785;
t914 = -t786;
t915 = -t796;
t916 = -t797;
t917 = -t798;
t918 = -t799;
t919 = -t800;
t920 = -t801;
t921 = -t802;
t922 = -t803;
t923 = -t804;
t924 = -t805;
t925 = -t810;
t926 = -t811;
t927 = -t812;
t928 = -t813;
t929 = -t814;
t930 = -t815;
t931 = -t817;
t932 = -t818;
t933 = -t828;
t934 = -t829;
t935 = -t831;
t936 = -t832;
t1001 = -t835;
t1002 = -t838;
t1003 = -t839;
t1007 = t34*t484;
t1008 = t34*t485;
t1009 = t34*t488;
t1010 = t34*t489;
t1015 = t35*t499;
t1016 = t35*t501;
t1017 = t34*t502;
t1018 = t34*t504;
t1019 = t35*t503;
t1020 = t35*t506;
t1023 = t34*t514;
t1024 = t34*t515;
t1031 = t35*t530;
t1032 = t35*t531;
t1033 = t35*t532;
t1034 = t35*t533;
t1094 = -t949;
t1095 = -t950;
t1096 = -t951;
t1097 = -t952;
t1098 = -t953;
t1099 = -t954;
t1100 = -t956;
t1101 = -t959;
t1107 = -t969;
t1108 = -t971;
t1109 = -t972;
t1110 = -t974;
t1111 = -t975;
t1112 = -t977;
t1113 = -t978;
t1115 = -t981;
t1200 = -t1011;
t1201 = -t1012;
t1204 = -t1021;
t1205 = -t1022;
t1216 = t35*t550;
t1218 = -t1040;
t1219 = -t1041;
t1224 = -t1053;
t1225 = -t1054;
t1226 = -t1055;
t1230 = -t1065;
t1258 = -t1078;
t1336 = -t1198;
t1337 = -t1199;
t1401 = -t1236;
t1406 = -t1241;
t1407 = -t1242;
t1408 = -t1243;
t1409 = -t1244;
t1410 = -t1255;
t1411 = -t1256;
t1412 = -t1257;
t1455 = t36*t796;
t1463 = t35*t835;
t1472 = -t1338;
t1473 = -t1339;
t1474 = -t1340;
t1475 = -t1353;
t1476 = -t1354;
t1477 = -t1357;
t1480 = -t1360;
t1481 = -t1361;
t1487 = -t1388;
t1488 = -t1389;
t1489 = -t1390;
t1490 = -t1391;
t1491 = -t1392;
t1492 = -t1393;
t1493 = -t1394;
t1494 = -t1395;
t1495 = -t1397;
t1496 = -t1398;
t1504 = -t1421;
t1505 = -t1422;
t1541 = -t1453;
t1542 = -t1454;
t1549 = t36*t945;
t1550 = t36*t946;
t1561 = t36*t969;
t1562 = t36*t971;
t1563 = t36*t972;
t1564 = t36*t974;
t1565 = t35*t976;
t1566 = t35*t979;
t1586 = -t1497;
t1648 = t35*t1202;
t1649 = t35*t1203;
t1669 = t35*t1236;
t1676 = t36*t1261;
t1678 = -t1617;
t1689 = -t1634;
t1690 = -t1635;
t1691 = -t1636;
t1692 = -t1637;
t1693 = -t1638;
t1694 = -t1639;
t1695 = -t1640;
t1696 = -t1641;
t1697 = -t1642;
t1711 = -t1673;
t1712 = -t1674;
t1714 = -t1679;
t1715 = -t1680;
t1716 = -t1681;
t1717 = -t1682;
t1719 = t35*t1478;
t1720 = t35*t1479;
t1735 = -t1723;
t1736 = -t1724;
t1739 = t35*t1608;
t1740 = t35*t1609;
t1578 = t35*t1023;
t1579 = t35*t1024;
t1731 = t35*t1549;
t1732 = t35*t1550;
et1 = Ixx2*dQ1*dQ2*t37-Ixx3*dQ1*dQ2*t37-Ixx3*dQ1*dQ2*t38-Ixx3*dQ1*dQ3*t37-Ixx3*dQ1*dQ3*t38+Ixx5*dQ1*dQ2*t37+Ixx5*dQ1*dQ2*t38+Ixx5*dQ1*dQ3*t37-Ixx6*dQ1*dQ2*t37+Ixx5*dQ1*dQ3*t38-Ixx6*dQ1*dQ2*t38-Ixx6*dQ1*dQ3*t37-Ixx6*dQ1*dQ3*t38+Ixx5*dQ1*dQ5*t40-Ixx6*dQ1*dQ6*t41-Iyy4*dQ1*dQ2*t37-Iyy4*dQ1*dQ2*t38-Iyy4*dQ1*dQ3*t37-Iyy5*dQ1*dQ2*t37-Iyy4*dQ1*dQ3*t38-Iyy5*dQ1*dQ2*t38-Iyy5*dQ1*dQ3*t37+Iyy6*dQ1*dQ2*t37-Iyy5*dQ1*dQ3*t38+Iyy6*dQ1*dQ2*t38+Iyy6*dQ1*dQ3*t37+Iyy6*dQ1*dQ3*t38+Iyy6*dQ1*dQ5*t40+Iyy6*dQ1*dQ6*t41-Izz2*dQ1*dQ2*t37+Izz3*dQ1*dQ2*t37+Izz3*dQ1*dQ2*t38;
et2 = Izz3*dQ1*dQ3*t37+Izz4*dQ1*dQ2*t37+Izz3*dQ1*dQ3*t38+Izz4*dQ1*dQ2*t38+Izz4*dQ1*dQ3*t37+Izz4*dQ1*dQ3*t38-Izz5*dQ1*dQ5*t40-Izz6*dQ1*dQ5*t40-Lxcm6*Lycm6*dQ1*dQ6*m6*2.0-Lx2*Lzcm2*dQ1*dQ2*m2*2.0+Lx3*Lzcm3*dQ1*dQ2*m3*2.0+Lx3*Lzcm3*dQ1*dQ3*m3*2.0+Lx3*Lzcm4*dQ1*dQ2*m4*2.0+Lx3*Lzcm4*dQ1*dQ3*m4*2.0-Lxcm2*Lzcm2*dQ1*dQ2*m2*2.0+Lxcm3*Lzcm3*dQ1*dQ2*m3*2.0+Lxcm3*Lzcm3*dQ1*dQ3*m3*2.0-Lxcm5*Lzcm5*dQ1*dQ5*m5*2.0+Ixx4*dQ2*dQ4*t2*t8+Ixx4*dQ2*dQ4*t3*t7+Ixx4*dQ3*dQ4*t2*t8+Ixx4*dQ3*dQ4*t3*t7-Ixx5*dQ2*dQ4*t2*t8-Ixx5*dQ2*dQ4*t3*t7-Ixx5*dQ3*dQ4*t2*t8-Ixx5*dQ3*dQ4*t3*t7-Ixx6*dQ2*dQ4*t2*t8-Ixx6*dQ2*dQ4*t3*t7-Ixx6*dQ3*dQ4*t2*t8;
et3 = -Ixx6*dQ3*dQ4*t3*t7-Iyy4*dQ2*dQ4*t2*t8-Iyy4*dQ2*dQ4*t3*t7-Iyy4*dQ3*dQ4*t2*t8-Iyy4*dQ3*dQ4*t3*t7-Iyy5*dQ2*dQ4*t2*t8-Iyy5*dQ2*dQ4*t3*t7-Iyy5*dQ3*dQ4*t2*t8-Iyy5*dQ3*dQ4*t3*t7-Iyy6*dQ2*dQ4*t2*t8-Iyy6*dQ2*dQ4*t3*t7-Iyy6*dQ3*dQ4*t2*t8-Iyy6*dQ3*dQ4*t3*t7-Izz4*dQ2*dQ4*t2*t8-Izz4*dQ2*dQ4*t3*t7-Izz4*dQ3*dQ4*t2*t8-Izz4*dQ3*dQ4*t3*t7+Izz5*dQ2*dQ4*t2*t8+Izz5*dQ2*dQ4*t3*t7+Izz5*dQ3*dQ4*t2*t8+Izz5*dQ3*dQ4*t3*t7+Izz6*dQ2*dQ4*t2*t8+Izz6*dQ2*dQ4*t3*t7+Izz6*dQ3*dQ4*t2*t8+Izz6*dQ3*dQ4*t3*t7-dQ1*dQ2*m2*t12*t37-dQ1*dQ2*m3*t12*t37;
et4 = dQ1*dQ2*m3*t13*t37-dQ1*dQ2*m4*t12*t37+dQ1*dQ2*m3*t13*t38+dQ1*dQ2*m4*t13*t37-dQ1*dQ2*m5*t12*t37+dQ1*dQ3*m3*t13*t37+dQ1*dQ2*m3*t15*t37+dQ1*dQ2*m4*t13*t38+dQ1*dQ2*m5*t13*t37-dQ1*dQ2*m6*t12*t37+dQ1*dQ3*m3*t13*t38+dQ1*dQ3*m4*t13*t37+dQ1*dQ2*m3*t15*t38+dQ1*dQ2*m5*t13*t38+dQ1*dQ2*m6*t13*t37+dQ1*dQ3*m3*t15*t37+dQ1*dQ3*m4*t13*t38+dQ1*dQ3*m5*t13*t37+dQ1*dQ2*m6*t13*t38+dQ1*dQ3*m3*t15*t38+dQ1*dQ3*m5*t13*t38+dQ1*dQ3*m6*t13*t37+dQ1*dQ3*m6*t13*t38-dQ1*dQ2*m5*t17*t37+dQ1*dQ2*m4*t19*t37-dQ1*dQ2*m5*t17*t38-dQ1*dQ3*m5*t17*t37+dQ1*dQ2*m4*t19*t38+dQ1*dQ2*m6*t18*t37+dQ1*dQ3*m4*t19*t37-dQ1*dQ3*m5*t17*t38;
et5 = dQ1*dQ2*m5*t20*t37+dQ1*dQ2*m6*t18*t38+dQ1*dQ3*m4*t19*t38+dQ1*dQ3*m6*t18*t37-dQ1*dQ2*m3*t23*t37+dQ1*dQ2*m5*t20*t38+dQ1*dQ3*m5*t20*t37+dQ1*dQ3*m6*t18*t38-dQ1*dQ2*m3*t23*t38-dQ1*dQ2*m6*t21*t37-dQ1*dQ3*m3*t23*t37+dQ1*dQ3*m5*t20*t38-dQ1*dQ2*m4*t24*t37-dQ1*dQ2*m6*t21*t38-dQ1*dQ3*m3*t23*t38-dQ1*dQ3*m6*t21*t37-dQ1*dQ5*m5*t17*t40-dQ1*dQ2*m4*t24*t38-dQ1*dQ3*m4*t24*t37-dQ1*dQ3*m6*t21*t38-dQ1*dQ3*m4*t24*t38+dQ1*dQ6*m6*t18*t41-dQ1*dQ5*m6*t21*t40+dQ1*dQ5*m6*t22*t40-dQ1*dQ6*m6*t21*t41+dQ1*dQ5*m5*t25*t40+dQ1*dQ5*m6*t26*t40-t3*t4*t7*t9*t80*4.0;
et6 = t3*t4*t7*t9*t84*4.0+t3*t4*t7*t9*t88*4.0+t3*t4*t7*t9*t90*4.0-t3*t4*t7*t9*t98*4.0-t3*t4*t7*t9*t100*4.0+t2*t4*t8*t9*t129+t3*t4*t7*t9*t129+t2*t4*t8*t9*t130+t3*t4*t7*t9*t130+t2*t4*t8*t9*t133+t3*t4*t7*t9*t133+t2*t4*t8*t9*t134+t3*t4*t7*t9*t134+t3*t4*t7*t9*t149*4.0-t3*t4*t7*t9*t153*4.0+t2*t4*t8*t9*t200+t3*t4*t7*t9*t200+t2*t4*t8*t9*t202+t3*t4*t7*t9*t202+t2*t4*t8*t9*t205+t3*t4*t7*t9*t205+t2*t4*t8*t9*t206+t3*t4*t7*t9*t206+t2*t4*t8*t9*t484+t3*t4*t7*t9*t484+t2*t4*t8*t9*t485+t3*t4*t7*t9*t485+t2*t4*t8*t9*t488+t3*t4*t7*t9*t488+t2*t4*t8*t9*t489+t3*t4*t7*t9*t489;
et7 = t2*t4*t8*t9*t502+t3*t4*t7*t9*t502+t2*t4*t8*t9*t504+t3*t4*t7*t9*t504+t2*t4*t8*t9*t505+t3*t4*t7*t9*t505+t2*t4*t8*t9*t508+t3*t4*t7*t9*t508+t2*t4*t8*t9*t698+t3*t4*t7*t9*t698+t2*t4*t8*t9*t699+t3*t4*t7*t9*t699+t2*t4*t8*t9*t975+t3*t4*t7*t9*t975+t2*t4*t8*t9*t977+t3*t4*t7*t9*t977+t2*t4*t8*t9*t978+t3*t4*t7*t9*t978+t2*t4*t8*t9*t981+t3*t4*t7*t9*t981-Lxcm2^2*dQ1*dQ2*m2*t37+Lzcm2^2*dQ1*dQ2*m2*t37+t3*t5*t6*t7*t11*t84*4.0-t2*t5*t6*t8*t11*t86*2.0-t3*t5*t6*t7*t11*t86*2.0-t3*t5*t6*t7*t11*t92*4.0+t2*t5*t6*t8*t11*t94*2.0+t3*t5*t6*t7*t11*t94*2.0-t3*t4*t7*t9*t35*t82*4.0;
et8 = t3*t4*t7*t9*t36*t84*-4.0-t3*t4*t7*t9*t35*t92*4.0+t3*t4*t7*t9*t36*t92*4.0+t3*t4*t7*t9*t35*t98*4.0+t3*t4*t7*t9*t35*t100*4.0-t3*t4*t7*t9*t36*t149*8.0+t3*t4*t7*t9*t36*t153*8.0+Lx2*Lx3*dQ1*dQ2*m3*t8*2.0+Lx2*Lx3*dQ1*dQ2*m4*t8*2.0+Lx2*Lx3*dQ1*dQ2*m5*t8*2.0+Lx2*Lx3*dQ1*dQ2*m6*t8*2.0-Lx3*Lx4*dQ1*dQ4*m4*t9*2.0-Lx3*Lx4*dQ1*dQ4*m5*t9*2.0-Lx3*Lx4*dQ1*dQ4*m6*t9*2.0+Lx2*Lxcm3*dQ1*dQ2*m3*t8*2.0-Lx3*Lxcm4*dQ1*dQ4*m4*t9*2.0-Lx3*Lxcm5*dQ1*dQ2*m5*t10*2.0-Lx3*Lxcm5*dQ1*dQ3*m5*t10*2.0-Lx4*Lxcm5*dQ1*dQ5*m5*t10*2.0-Lx2*Lxcm2*dQ1*dQ2*m2*t37*2.0+Lx3*Lxcm3*dQ1*dQ2*m3*t37*2.0+Lx3*Lxcm3*dQ1*dQ2*m3*t38*2.0+Lx3*Lxcm3*dQ1*dQ3*m3*t37*2.0;
et9 = Lx3*Lxcm3*dQ1*dQ3*m3*t38*2.0-Lx3*Lycm4*dQ1*dQ4*m4*t4*2.0-Lx3*Lycm5*dQ1*dQ4*m5*t4*2.0-Lx4*Lycm4*dQ1*dQ4*m4*t32*2.0-Lx4*Lycm4*dQ1*dQ4*m4*t33*2.0-Lx4*Lycm5*dQ1*dQ4*m5*t32*2.0-Lx4*Lycm5*dQ1*dQ4*m5*t33*2.0-Lxcm4*Lycm4*dQ1*dQ4*m4*t32*2.0-Lxcm4*Lycm4*dQ1*dQ4*m4*t33*2.0+Lxcm6*Lycm6*dQ1*dQ6*m6*t32*4.0+Lxcm6*Lycm6*dQ1*dQ6*m6*t33*4.0+Lxcm6*Lycm6*dQ1*dQ6*m6*t35*2.0+Lxcm6*Lycm6*dQ1*dQ6*m6*t36*4.0+Lx3*Lz6*dQ1*dQ2*m6*t5*2.0+Lx3*Lz6*dQ1*dQ3*m6*t5*2.0+Lx4*Lz6*dQ1*dQ5*m6*t5*2.0-Lx2*Lzcm3*dQ1*dQ2*m3*t3*2.0-Lx2*Lzcm4*dQ1*dQ2*m4*t3*2.0+Lx4*Lzcm4*dQ1*dQ2*m4*t4*2.0+Lx4*Lzcm4*dQ1*dQ3*m4*t4*2.0+Lx3*Lzcm5*dQ1*dQ2*m5*t5*2.0+Lx3*Lzcm5*dQ1*dQ3*m5*t5*2.0+Lx3*Lzcm6*dQ1*dQ2*m6*t5*2.0;
et10 = Lx3*Lzcm6*dQ1*dQ3*m6*t5*2.0+Lx4*Lzcm5*dQ1*dQ5*m5*t5*2.0+Lx4*Lzcm6*dQ1*dQ5*m6*t5*2.0-Lxcm6*Lz6*dQ1*dQ5*m6*t6*2.0+Lx2*Lzcm2*dQ1*dQ2*m2*t32*4.0-Lx3*Lzcm3*dQ1*dQ2*m3*t32*4.0-Lx3*Lzcm3*dQ1*dQ2*m3*t33*4.0-Lx3*Lzcm3*dQ1*dQ3*m3*t32*4.0-Lx3*Lzcm3*dQ1*dQ3*m3*t33*4.0-Lx3*Lzcm4*dQ1*dQ2*m4*t32*4.0-Lx3*Lzcm4*dQ1*dQ2*m4*t33*4.0-Lx3*Lzcm4*dQ1*dQ3*m4*t32*4.0-Lx3*Lzcm4*dQ1*dQ3*m4*t33*4.0+Lxcm4*Lzcm4*dQ1*dQ2*m4*t4*2.0+Lxcm4*Lzcm4*dQ1*dQ3*m4*t4*2.0-Lxcm5*Lzcm5*dQ1*dQ2*m5*t4*2.0-Lxcm5*Lzcm5*dQ1*dQ3*m5*t4*2.0-Lxcm6*Lzcm6*dQ1*dQ5*m6*t6*2.0+Lxcm2*Lzcm2*dQ1*dQ2*m2*t32*4.0-Lxcm3*Lzcm3*dQ1*dQ2*m3*t32*4.0-Lxcm3*Lzcm3*dQ1*dQ2*m3*t33*4.0-Lxcm3*Lzcm3*dQ1*dQ3*m3*t32*4.0-Lxcm3*Lzcm3*dQ1*dQ3*m3*t33*4.0;
et11 = Lxcm5*Lzcm5*dQ1*dQ5*m5*t32*2.0+Lxcm5*Lzcm5*dQ1*dQ5*m5*t33*2.0+Lxcm5*Lzcm5*dQ1*dQ5*m5*t35*4.0+Lycm6*Lz6*dQ1*dQ5*m6*t11*2.0-Lycm4*Lzcm4*dQ1*dQ2*m4*t9*2.0-Lycm4*Lzcm4*dQ1*dQ3*m4*t9*2.0+Lycm6*Lzcm6*dQ1*dQ5*m6*t11*2.0+Lz6*Lzcm6*dQ1*dQ5*m6*t40*2.0+Ixx5*dQ1*dQ5*t2*t4*t7*2.0+Ixx5*dQ1*dQ5*t3*t4*t8*2.0+Ixx5*dQ2*dQ5*t2*t3*t9+Ixx5*dQ1*dQ2*t4*t5*t10*2.0+Ixx5*dQ3*dQ5*t2*t3*t9+Ixx6*dQ2*dQ5*t2*t3*t9+Ixx5*dQ1*dQ3*t4*t5*t10*2.0-Ixx5*dQ4*dQ5*t2*t4*t8-Ixx5*dQ4*dQ5*t3*t4*t7+Ixx6*dQ3*dQ5*t2*t3*t9-Ixx6*dQ2*dQ6*t2*t5*t8-Ixx6*dQ2*dQ6*t3*t5*t7+Ixx6*dQ4*dQ5*t2*t4*t8+Ixx6*dQ4*dQ5*t3*t4*t7-Ixx6*dQ3*dQ6*t2*t5*t8-Ixx6*dQ3*dQ6*t3*t5*t7;
et12 = Ixx6*dQ5*dQ6*t2*t3*t10-Ixx5*dQ2*dQ5*t7*t8*t9-Ixx5*dQ3*dQ5*t7*t8*t9-Ixx6*dQ2*dQ5*t7*t8*t9-Ixx6*dQ3*dQ5*t7*t8*t9-Ixx6*dQ5*dQ6*t7*t8*t10+Ixx3*dQ1*dQ2*t2*t7*t33*4.0+Ixx3*dQ1*dQ2*t3*t8*t32*4.0+Ixx3*dQ1*dQ3*t2*t7*t33*4.0+Ixx3*dQ1*dQ3*t3*t8*t32*4.0-Ixx4*dQ1*dQ2*t2*t7*t34*2.0-Ixx5*dQ1*dQ2*t2*t7*t33*4.0-Ixx4*dQ1*dQ3*t2*t7*t34*2.0-Ixx5*dQ1*dQ2*t3*t8*t32*4.0-Ixx5*dQ1*dQ3*t2*t7*t33*4.0+Ixx6*dQ1*dQ2*t2*t7*t33*4.0-Ixx4*dQ1*dQ2*t3*t8*t34*2.0-Ixx5*dQ1*dQ2*t2*t7*t35*2.0-Ixx5*dQ1*dQ3*t3*t8*t32*4.0+Ixx6*dQ1*dQ2*t2*t7*t34*2.0+Ixx6*dQ1*dQ2*t3*t8*t32*4.0+Ixx6*dQ1*dQ3*t2*t7*t33*4.0-Ixx4*dQ1*dQ3*t3*t8*t34*2.0;
et13 = Ixx5*dQ1*dQ3*t2*t7*t35*-2.0+Ixx6*dQ1*dQ3*t2*t7*t34*2.0+Ixx6*dQ1*dQ3*t3*t8*t32*4.0-Ixx4*dQ1*dQ4*t4*t9*t32*2.0-Ixx4*dQ2*dQ4*t2*t8*t34*2.0-Ixx4*dQ2*dQ4*t3*t7*t34*2.0-Ixx5*dQ1*dQ2*t3*t8*t35*2.0+Ixx6*dQ1*dQ2*t2*t7*t36*4.0+Ixx6*dQ1*dQ2*t3*t8*t34*2.0-Ixx4*dQ1*dQ4*t4*t9*t33*2.0-Ixx4*dQ3*dQ4*t2*t8*t34*2.0-Ixx4*dQ3*dQ4*t3*t7*t34*2.0-Ixx5*dQ1*dQ3*t3*t8*t35*2.0+Ixx6*dQ1*dQ3*t2*t7*t36*4.0+Ixx6*dQ1*dQ3*t3*t8*t34*2.0+Ixx5*dQ2*dQ4*t2*t8*t35*2.0+Ixx5*dQ2*dQ4*t3*t7*t35*2.0+Ixx6*dQ1*dQ2*t3*t8*t36*4.0+Ixx6*dQ1*dQ4*t4*t9*t32*2.0+Ixx6*dQ2*dQ4*t2*t8*t34*2.0+Ixx6*dQ2*dQ4*t3*t7*t34*2.0+Ixx5*dQ3*dQ4*t2*t8*t35*2.0+Ixx5*dQ3*dQ4*t3*t7*t35*2.0;
et14 = Ixx6*dQ1*dQ3*t3*t8*t36*4.0+Ixx6*dQ1*dQ4*t4*t9*t33*2.0+Ixx6*dQ3*dQ4*t2*t8*t34*2.0+Ixx6*dQ3*dQ4*t3*t7*t34*2.0-Ixx5*dQ1*dQ5*t5*t10*t32*2.0-Ixx5*dQ1*dQ5*t5*t10*t33*2.0+Ixx6*dQ1*dQ6*t6*t11*t32*4.0+Ixx6*dQ1*dQ5*t5*t10*t36*2.0+Ixx6*dQ1*dQ6*t6*t11*t33*4.0+Ixx6*dQ1*dQ6*t6*t11*t35*2.0+Iyy6*dQ1*dQ5*t2*t4*t7*2.0+Iyy5*dQ2*dQ5*t2*t3*t9+Iyy5*dQ3*dQ5*t2*t3*t9+Iyy6*dQ1*dQ5*t3*t4*t8*2.0+Iyy6*dQ2*dQ5*t2*t3*t9+Iyy5*dQ4*dQ5*t2*t4*t8+Iyy5*dQ4*dQ5*t3*t4*t7+Iyy6*dQ1*dQ2*t4*t5*t10*2.0+Iyy6*dQ3*dQ5*t2*t3*t9+Iyy6*dQ1*dQ3*t4*t5*t10*2.0+Iyy6*dQ2*dQ6*t2*t5*t8+Iyy6*dQ2*dQ6*t3*t5*t7-Iyy6*dQ4*dQ5*t2*t4*t8-Iyy6*dQ4*dQ5*t3*t4*t7+Iyy6*dQ3*dQ6*t2*t5*t8;
et15 = Iyy6*dQ3*dQ6*t3*t5*t7-Iyy6*dQ5*dQ6*t2*t3*t10-Iyy5*dQ2*dQ5*t7*t8*t9-Iyy5*dQ3*dQ5*t7*t8*t9-Iyy6*dQ2*dQ5*t7*t8*t9-Iyy6*dQ3*dQ5*t7*t8*t9+Iyy6*dQ5*dQ6*t7*t8*t10+Iyy4*dQ1*dQ2*t2*t7*t33*4.0+Iyy4*dQ1*dQ2*t2*t7*t34*2.0+Iyy4*dQ1*dQ2*t3*t8*t32*4.0+Iyy4*dQ1*dQ3*t2*t7*t33*4.0+Iyy5*dQ1*dQ2*t2*t7*t33*4.0+Iyy4*dQ1*dQ3*t2*t7*t34*2.0+Iyy4*dQ1*dQ3*t3*t8*t32*4.0+Iyy5*dQ1*dQ2*t2*t7*t34*2.0+Iyy5*dQ1*dQ2*t3*t8*t32*4.0+Iyy5*dQ1*dQ3*t2*t7*t33*4.0-Iyy6*dQ1*dQ2*t2*t7*t33*4.0+Iyy4*dQ1*dQ2*t3*t8*t34*2.0+Iyy5*dQ1*dQ3*t2*t7*t34*2.0+Iyy5*dQ1*dQ3*t3*t8*t32*4.0-Iyy6*dQ1*dQ2*t3*t8*t32*4.0-Iyy6*dQ1*dQ3*t2*t7*t33*4.0+Iyy4*dQ1*dQ3*t3*t8*t34*2.0;
et16 = Iyy5*dQ1*dQ2*t3*t8*t34*2.0-Iyy6*dQ1*dQ2*t2*t7*t35*2.0-Iyy6*dQ1*dQ3*t3*t8*t32*4.0+Iyy4*dQ1*dQ4*t4*t9*t32*2.0+Iyy4*dQ2*dQ4*t2*t8*t34*2.0+Iyy4*dQ2*dQ4*t3*t7*t34*2.0+Iyy5*dQ1*dQ3*t3*t8*t34*2.0-Iyy6*dQ1*dQ2*t2*t7*t36*4.0-Iyy6*dQ1*dQ3*t2*t7*t35*2.0+Iyy4*dQ1*dQ4*t4*t9*t33*2.0+Iyy4*dQ3*dQ4*t2*t8*t34*2.0+Iyy4*dQ3*dQ4*t3*t7*t34*2.0+Iyy5*dQ1*dQ4*t4*t9*t32*2.0+Iyy5*dQ2*dQ4*t2*t8*t34*2.0+Iyy5*dQ2*dQ4*t3*t7*t34*2.0-Iyy6*dQ1*dQ2*t3*t8*t35*2.0-Iyy6*dQ1*dQ3*t2*t7*t36*4.0+Iyy5*dQ1*dQ4*t4*t9*t33*2.0+Iyy5*dQ3*dQ4*t2*t8*t34*2.0+Iyy5*dQ3*dQ4*t3*t7*t34*2.0-Iyy6*dQ1*dQ2*t3*t8*t36*4.0-Iyy6*dQ1*dQ3*t3*t8*t35*2.0-Iyy6*dQ1*dQ3*t3*t8*t36*4.0;
et17 = Iyy6*dQ2*dQ4*t2*t8*t35*2.0+Iyy6*dQ2*dQ4*t3*t7*t35*2.0+Iyy6*dQ3*dQ4*t2*t8*t35*2.0+Iyy6*dQ3*dQ4*t3*t7*t35*2.0-Iyy6*dQ1*dQ5*t5*t10*t32*2.0-Iyy6*dQ1*dQ5*t5*t10*t33*2.0-Iyy6*dQ1*dQ6*t6*t11*t32*4.0-Iyy6*dQ1*dQ5*t5*t10*t36*2.0-Iyy6*dQ1*dQ6*t6*t11*t33*4.0-Iyy6*dQ1*dQ6*t6*t11*t35*2.0-Izz5*dQ1*dQ5*t2*t4*t7*2.0-Izz6*dQ1*dQ5*t2*t4*t7*2.0-Izz5*dQ1*dQ5*t3*t4*t8*2.0-Izz5*dQ2*dQ5*t2*t3*t9-Izz5*dQ1*dQ2*t4*t5*t10*2.0-Izz5*dQ3*dQ5*t2*t3*t9-Izz6*dQ1*dQ5*t3*t4*t8*2.0-Izz6*dQ2*dQ5*t2*t3*t9-Izz5*dQ1*dQ3*t4*t5*t10*2.0+Izz5*dQ4*dQ5*t2*t4*t8+Izz5*dQ4*dQ5*t3*t4*t7-Izz6*dQ1*dQ2*t4*t5*t10*2.0-Izz6*dQ3*dQ5*t2*t3*t9;
et18 = Izz6*dQ1*dQ3*t4*t5*t10*-2.0-Izz6*dQ2*dQ6*t2*t5*t8-Izz6*dQ2*dQ6*t3*t5*t7+Izz6*dQ4*dQ5*t2*t4*t8+Izz6*dQ4*dQ5*t3*t4*t7-Izz6*dQ3*dQ6*t2*t5*t8-Izz6*dQ3*dQ6*t3*t5*t7-Izz6*dQ5*dQ6*t2*t3*t10+Izz5*dQ2*dQ5*t7*t8*t9+Izz5*dQ3*dQ5*t7*t8*t9+Izz6*dQ2*dQ5*t7*t8*t9+Izz6*dQ3*dQ5*t7*t8*t9+Izz6*dQ5*dQ6*t7*t8*t10-Izz3*dQ1*dQ2*t2*t7*t33*4.0-Izz3*dQ1*dQ2*t3*t8*t32*4.0-Izz3*dQ1*dQ3*t2*t7*t33*4.0-Izz4*dQ1*dQ2*t2*t7*t33*4.0-Izz3*dQ1*dQ3*t3*t8*t32*4.0-Izz4*dQ1*dQ2*t3*t8*t32*4.0-Izz4*dQ1*dQ3*t2*t7*t33*4.0-Izz4*dQ1*dQ3*t3*t8*t32*4.0-Izz5*dQ1*dQ2*t2*t7*t34*2.0+Izz5*dQ1*dQ2*t2*t7*t35*2.0;
et19 = Izz5*dQ1*dQ3*t2*t7*t34*-2.0-Izz6*dQ1*dQ2*t2*t7*t34*2.0-Izz5*dQ1*dQ2*t3*t8*t34*2.0+Izz5*dQ1*dQ3*t2*t7*t35*2.0+Izz6*dQ1*dQ2*t2*t7*t35*2.0-Izz6*dQ1*dQ3*t2*t7*t34*2.0+Izz5*dQ1*dQ2*t3*t8*t35*2.0-Izz5*dQ1*dQ3*t3*t8*t34*2.0-Izz6*dQ1*dQ2*t3*t8*t34*2.0+Izz6*dQ1*dQ3*t2*t7*t35*2.0+Izz5*dQ1*dQ3*t3*t8*t35*2.0-Izz5*dQ1*dQ4*t4*t9*t32*2.0-Izz5*dQ2*dQ4*t2*t8*t34*2.0-Izz5*dQ2*dQ4*t3*t7*t34*2.0+Izz6*dQ1*dQ2*t3*t8*t35*2.0-Izz6*dQ1*dQ3*t3*t8*t34*2.0-Izz5*dQ1*dQ4*t4*t9*t33*2.0-Izz5*dQ2*dQ4*t2*t8*t35*2.0-Izz5*dQ2*dQ4*t3*t7*t35*2.0-Izz5*dQ3*dQ4*t2*t8*t34*2.0-Izz5*dQ3*dQ4*t3*t7*t34*2.0+Izz6*dQ1*dQ3*t3*t8*t35*2.0-Izz6*dQ1*dQ4*t4*t9*t32*2.0;
et20 = Izz6*dQ2*dQ4*t2*t8*t34*-2.0-Izz6*dQ2*dQ4*t3*t7*t34*2.0-Izz5*dQ3*dQ4*t2*t8*t35*2.0-Izz5*dQ3*dQ4*t3*t7*t35*2.0-Izz6*dQ1*dQ4*t4*t9*t33*2.0-Izz6*dQ2*dQ4*t2*t8*t35*2.0-Izz6*dQ2*dQ4*t3*t7*t35*2.0-Izz6*dQ3*dQ4*t2*t8*t34*2.0-Izz6*dQ3*dQ4*t3*t7*t34*2.0+Izz5*dQ1*dQ5*t5*t10*t32*2.0-Izz6*dQ3*dQ4*t2*t8*t35*2.0-Izz6*dQ3*dQ4*t3*t7*t35*2.0+Izz5*dQ1*dQ5*t5*t10*t33*2.0+Izz6*dQ1*dQ5*t5*t10*t32*2.0+Izz6*dQ1*dQ5*t5*t10*t33*2.0-dQ2*dQ4*m4*t2*t8*t14*2.0-dQ2*dQ4*m4*t3*t7*t14*2.0-dQ2*dQ4*m5*t2*t8*t14*2.0-dQ2*dQ4*m5*t3*t7*t14*2.0-dQ3*dQ4*m4*t2*t8*t14*2.0-dQ3*dQ4*m4*t3*t7*t14*2.0-dQ2*dQ4*m4*t2*t8*t16*2.0;
et21 = dQ2*dQ4*m4*t3*t7*t16*-2.0-dQ2*dQ4*m6*t2*t8*t14*2.0-dQ2*dQ4*m6*t3*t7*t14*2.0-dQ3*dQ4*m5*t2*t8*t14*2.0-dQ3*dQ4*m5*t3*t7*t14*2.0-dQ3*dQ4*m4*t2*t8*t16*2.0-dQ3*dQ4*m4*t3*t7*t16*2.0-dQ3*dQ4*m6*t2*t8*t14*2.0-dQ3*dQ4*m6*t3*t7*t14*2.0-dQ2*dQ4*m6*t2*t8*t22*2.0-dQ2*dQ4*m6*t3*t7*t22*2.0-dQ3*dQ4*m6*t2*t8*t22*2.0-dQ3*dQ4*m6*t3*t7*t22*2.0-dQ2*dQ4*m5*t2*t8*t25*2.0-dQ2*dQ4*m5*t3*t7*t25*2.0-dQ3*dQ4*m5*t2*t8*t25*2.0-dQ3*dQ4*m5*t3*t7*t25*2.0-dQ2*dQ4*m6*t2*t8*t26*2.0-dQ2*dQ4*m6*t3*t7*t26*2.0-dQ3*dQ4*m6*t2*t8*t26*2.0-dQ3*dQ4*m6*t3*t7*t26*2.0+Lx2*Lx4*dQ1*dQ2*m4*t4*t8*2.0;
et22 = Lx2*Lx4*dQ1*dQ2*m5*t4*t8*2.0+Lx2*Lx4*dQ1*dQ2*m6*t4*t8*2.0-Lx2*Lx3*dQ1*dQ2*m3*t8*t32*4.0-Lx2*Lx3*dQ1*dQ2*m4*t8*t32*4.0-Lx2*Lx3*dQ1*dQ3*m3*t8*t32*2.0-Lx2*Lx3*dQ1*dQ2*m5*t8*t32*4.0-Lx2*Lx3*dQ1*dQ3*m4*t8*t32*2.0-Lx2*Lx3*dQ1*dQ2*m6*t8*t32*4.0-Lx2*Lx3*dQ1*dQ3*m5*t8*t32*2.0-Lx2*Lx3*dQ1*dQ3*m6*t8*t32*2.0+Lx3*Lx4*dQ1*dQ4*m4*t9*t32*2.0+Lx3*Lx4*dQ1*dQ4*m4*t9*t33*2.0+Lx3*Lx4*dQ1*dQ4*m5*t9*t32*2.0+Lx3*Lx4*dQ1*dQ4*m5*t9*t33*2.0+Lx3*Lx4*dQ1*dQ4*m6*t9*t32*2.0+Lx3*Lx4*dQ1*dQ4*m6*t9*t33*2.0+Lx2*Lxcm4*dQ1*dQ2*m4*t4*t8*2.0+Lx2*Lxcm5*dQ1*dQ2*m5*t3*t10*2.0-Lx4*Lxcm4*dQ2*dQ4*m4*t2*t8*4.0-Lx4*Lxcm4*dQ2*dQ4*m4*t3*t7*4.0-Lx4*Lxcm4*dQ3*dQ4*m4*t2*t8*4.0;
et23 = Lx4*Lxcm4*dQ3*dQ4*m4*t3*t7*-4.0-Lx4*Lxcm5*dQ1*dQ2*m5*t4*t10*2.0-Lx3*Lxcm5*dQ1*dQ4*m5*t5*t9*2.0-Lx4*Lxcm5*dQ1*dQ3*m5*t4*t10*2.0-Lx3*Lxcm5*dQ1*dQ5*m5*t4*t10*2.0-Lx3*Lxcm6*dQ1*dQ2*m6*t6*t10*2.0-Lx3*Lxcm6*dQ1*dQ3*m6*t6*t10*2.0-Lx3*Lxcm6*dQ1*dQ4*m6*t4*t11*2.0-Lx3*Lxcm6*dQ1*dQ6*m6*t6*t9*2.0-Lx4*Lxcm6*dQ1*dQ5*m6*t6*t10*2.0-Lx4*Lxcm6*dQ1*dQ6*m6*t5*t11*2.0-Lx2*Lxcm3*dQ1*dQ2*m3*t8*t32*4.0-Lx2*Lxcm3*dQ1*dQ3*m3*t8*t32*2.0+Lx3*Lxcm4*dQ1*dQ4*m4*t9*t32*2.0+Lx3*Lxcm4*dQ1*dQ4*m4*t9*t33*2.0+Lx3*Lxcm5*dQ1*dQ2*m5*t10*t32*4.0+Lx3*Lxcm5*dQ1*dQ2*m5*t10*t33*4.0+Lx3*Lxcm5*dQ1*dQ3*m5*t10*t32*4.0+Lx3*Lxcm5*dQ1*dQ3*m5*t10*t33*4.0-Lx4*Lxcm6*dQ1*dQ4*m6*t11*t32*2.0;
et24 = Lx4*Lxcm6*dQ1*dQ4*m6*t11*t33*-2.0+Lx3*Lycm3*dQ2*dQ3*m3*t2*t3*2.0-Lx4*Lycm4*dQ2*dQ3*m4*t2*t3*2.0-Lx4*Lycm5*dQ2*dQ3*m5*t2*t3*2.0-Lx3*Lycm3*dQ2*dQ3*m3*t7*t8*2.0-Lx2*Lycm4*dQ1*dQ2*m4*t8*t9*2.0-Lx3*Lycm6*dQ1*dQ4*m6*t4*t6*2.0-Lx2*Lycm5*dQ1*dQ2*m5*t8*t9*2.0+Lx4*Lycm4*dQ2*dQ3*m4*t7*t8*2.0+Lx4*Lycm5*dQ2*dQ3*m5*t7*t8*2.0-Lx4*Lycm6*dQ1*dQ6*m6*t5*t6*2.0+Lx3*Lycm6*dQ1*dQ2*m6*t10*t11*2.0+Lx3*Lycm6*dQ1*dQ3*m6*t10*t11*2.0+Lx3*Lycm6*dQ1*dQ6*m6*t9*t11*2.0+Lx4*Lycm6*dQ1*dQ5*m6*t10*t11*2.0+Lx3*Lycm4*dQ1*dQ4*m4*t4*t32*2.0+Lx3*Lycm4*dQ1*dQ4*m4*t4*t33*2.0+Lx3*Lycm5*dQ1*dQ4*m5*t4*t32*2.0+Lx3*Lycm5*dQ1*dQ4*m5*t4*t33*2.0-Lx4*Lycm6*dQ1*dQ4*m6*t6*t32*2.0-Lx4*Lycm6*dQ1*dQ4*m6*t6*t33*2.0;
et25 = Lx4*Lycm4*dQ1*dQ4*m4*t32*t33*4.0+Lx4*Lycm4*dQ1*dQ4*m4*t32*t34*4.0+Lx4*Lycm4*dQ1*dQ4*m4*t33*t34*4.0+Lx4*Lycm5*dQ1*dQ4*m5*t32*t33*4.0+Lx4*Lycm5*dQ1*dQ4*m5*t32*t34*4.0+Lx4*Lycm5*dQ1*dQ4*m5*t33*t34*4.0+Lxcm3*Lycm3*dQ2*dQ3*m3*t2*t3*2.0-Lxcm4*Lycm4*dQ2*dQ3*m4*t2*t3*2.0-Lxcm3*Lycm3*dQ2*dQ3*m3*t7*t8*2.0+Lxcm4*Lycm4*dQ2*dQ3*m4*t7*t8*2.0-Lxcm6*Lycm6*dQ4*dQ6*m6*t2*t3*2.0+Lxcm5*Lycm5*dQ1*dQ2*m5*t9*t10*2.0+Lxcm5*Lycm5*dQ1*dQ3*m5*t9*t10*2.0-Lxcm6*Lycm6*dQ1*dQ2*m6*t9*t10*2.0-Lxcm6*Lycm6*dQ1*dQ3*m6*t9*t10*2.0+Lxcm6*Lycm6*dQ4*dQ6*m6*t7*t8*2.0-Lxcm5*Lycm5*dQ1*dQ4*m5*t5*t32*2.0-Lxcm5*Lycm5*dQ1*dQ4*m5*t5*t33*2.0+Lxcm6*Lycm6*dQ1*dQ4*m6*t5*t32*2.0+Lxcm6*Lycm6*dQ1*dQ4*m6*t5*t33*2.0+Lxcm4*Lycm4*dQ1*dQ4*m4*t32*t33*4.0;
et26 = Lxcm4*Lycm4*dQ1*dQ4*m4*t32*t34*4.0+Lxcm4*Lycm4*dQ1*dQ4*m4*t33*t34*4.0-Lxcm6*Lycm6*dQ1*dQ6*m6*t32*t33*8.0-Lxcm6*Lycm6*dQ1*dQ6*m6*t32*t34*2.0-Lxcm6*Lycm6*dQ1*dQ6*m6*t32*t35*2.0-Lxcm6*Lycm6*dQ1*dQ6*m6*t33*t34*2.0-Lxcm6*Lycm6*dQ1*dQ6*m6*t32*t36*8.0-Lxcm6*Lycm6*dQ1*dQ6*m6*t33*t35*2.0-Lxcm6*Lycm6*dQ1*dQ6*m6*t33*t36*8.0-Lxcm6*Lycm6*dQ1*dQ6*m6*t35*t36*4.0-Lx2*Lz6*dQ1*dQ2*m6*t3*t5*2.0+Lx4*Lz6*dQ1*dQ2*m6*t4*t5*2.0+Lx4*Lz6*dQ1*dQ3*m6*t4*t5*2.0+Lx3*Lz6*dQ1*dQ5*m6*t4*t5*2.0-Lx3*Lz6*dQ1*dQ4*m6*t9*t10*2.0-Lx3*Lz6*dQ1*dQ2*m6*t5*t32*4.0-Lx3*Lz6*dQ1*dQ2*m6*t5*t33*4.0-Lx3*Lz6*dQ1*dQ3*m6*t5*t32*4.0-Lx3*Lz6*dQ1*dQ3*m6*t5*t33*4.0-Lx2*Lzcm5*dQ1*dQ2*m5*t3*t5*2.0;
et27 = Lx2*Lzcm6*dQ1*dQ2*m6*t3*t5*-2.0+Lx4*Lzcm5*dQ1*dQ2*m5*t4*t5*2.0+Lx4*Lzcm5*dQ1*dQ3*m5*t4*t5*2.0+Lx3*Lzcm5*dQ1*dQ5*m5*t4*t5*2.0+Lx4*Lzcm6*dQ1*dQ2*m6*t4*t5*2.0+Lx4*Lzcm6*dQ1*dQ3*m6*t4*t5*2.0+Lx3*Lzcm6*dQ1*dQ5*m6*t4*t5*2.0-Lxcm6*Lz6*dQ1*dQ2*m6*t4*t6*2.0-Lxcm6*Lz6*dQ1*dQ3*m6*t4*t6*2.0-Lx3*Lzcm5*dQ1*dQ4*m5*t9*t10*2.0-Lx3*Lzcm6*dQ1*dQ4*m6*t9*t10*2.0+Lx2*Lzcm3*dQ1*dQ2*m3*t3*t32*4.0+Lx2*Lzcm3*dQ1*dQ3*m3*t3*t32*2.0+Lx2*Lzcm4*dQ1*dQ2*m4*t3*t32*4.0+Lx2*Lzcm4*dQ1*dQ3*m4*t3*t32*2.0-Lx4*Lzcm4*dQ1*dQ2*m4*t4*t32*4.0-Lx4*Lzcm4*dQ1*dQ2*m4*t4*t33*4.0-Lx4*Lzcm4*dQ1*dQ3*m4*t4*t32*4.0-Lx3*Lzcm5*dQ1*dQ2*m5*t5*t32*4.0-Lx4*Lzcm4*dQ1*dQ3*m4*t4*t33*4.0-Lx3*Lzcm5*dQ1*dQ2*m5*t5*t33*4.0;
et28 = Lx3*Lzcm5*dQ1*dQ3*m5*t5*t32*-4.0-Lx3*Lzcm5*dQ1*dQ3*m5*t5*t33*4.0-Lx3*Lzcm6*dQ1*dQ2*m6*t5*t32*4.0-Lx3*Lzcm6*dQ1*dQ2*m6*t5*t33*4.0-Lx3*Lzcm6*dQ1*dQ3*m6*t5*t32*4.0-Lx3*Lzcm6*dQ1*dQ3*m6*t5*t33*4.0+Lxcm6*Lz6*dQ1*dQ5*m6*t6*t32*2.0+Lxcm6*Lz6*dQ1*dQ5*m6*t6*t33*2.0+Lxcm6*Lz6*dQ1*dQ5*m6*t6*t35*4.0+Lx3*Lzcm3*dQ1*dQ2*m3*t32*t33*8.0+Lx3*Lzcm3*dQ1*dQ3*m3*t32*t33*8.0+Lx3*Lzcm4*dQ1*dQ2*m4*t32*t33*8.0+Lx3*Lzcm4*dQ1*dQ3*m4*t32*t33*8.0-Lxcm5*Lzcm5*dQ4*dQ5*m5*t2*t3*2.0-Lxcm6*Lzcm6*dQ1*dQ2*m6*t4*t6*2.0-Lxcm6*Lzcm6*dQ1*dQ3*m6*t4*t6*2.0+Lxcm5*Lzcm5*dQ4*dQ5*m5*t7*t8*2.0-Lxcm4*Lzcm4*dQ1*dQ2*m4*t4*t32*4.0-Lxcm4*Lzcm4*dQ1*dQ2*m4*t4*t33*4.0-Lxcm4*Lzcm4*dQ1*dQ3*m4*t4*t32*4.0;
et29 = Lxcm4*Lzcm4*dQ1*dQ3*m4*t4*t33*-4.0+Lxcm5*Lzcm5*dQ1*dQ2*m5*t4*t32*4.0+Lxcm5*Lzcm5*dQ1*dQ2*m5*t4*t33*4.0+Lxcm5*Lzcm5*dQ1*dQ3*m5*t4*t32*4.0+Lxcm5*Lzcm5*dQ1*dQ3*m5*t4*t33*4.0+Lxcm5*Lzcm5*dQ1*dQ2*m5*t4*t35*4.0+Lxcm5*Lzcm5*dQ1*dQ3*m5*t4*t35*4.0+Lxcm6*Lzcm6*dQ1*dQ5*m6*t6*t32*2.0+Lxcm6*Lzcm6*dQ1*dQ5*m6*t6*t33*2.0+Lxcm6*Lzcm6*dQ1*dQ5*m6*t6*t35*4.0+Lxcm3*Lzcm3*dQ1*dQ2*m3*t32*t33*8.0+Lxcm3*Lzcm3*dQ1*dQ3*m3*t32*t33*8.0-Lxcm5*Lzcm5*dQ1*dQ5*m5*t32*t33*4.0+Lxcm5*Lzcm5*dQ1*dQ5*m5*t32*t34*2.0-Lxcm5*Lzcm5*dQ1*dQ5*m5*t32*t35*4.0+Lxcm5*Lzcm5*dQ1*dQ5*m5*t33*t34*2.0-Lxcm5*Lzcm5*dQ1*dQ5*m5*t33*t35*4.0+Lycm6*Lz6*dQ1*dQ2*m6*t4*t11*2.0+Lycm6*Lz6*dQ1*dQ3*m6*t4*t11*2.0-Lycm6*Lz6*dQ1*dQ5*m6*t11*t32*2.0-Lycm6*Lz6*dQ1*dQ5*m6*t11*t33*2.0;
et30 = Lycm6*Lz6*dQ1*dQ5*m6*t11*t35*-4.0+Lycm3*Lzcm3*dQ2*dQ3*m3*t2*t8*2.0+Lycm3*Lzcm3*dQ2*dQ3*m3*t3*t7*2.0-Lycm5*Lzcm5*dQ1*dQ2*m5*t5*t9*2.0-Lycm5*Lzcm5*dQ1*dQ3*m5*t5*t9*2.0+Lycm6*Lzcm6*dQ1*dQ2*m6*t4*t11*2.0+Lycm6*Lzcm6*dQ1*dQ3*m6*t4*t11*2.0+Lycm4*Lzcm4*dQ1*dQ2*m4*t9*t32*4.0+Lycm4*Lzcm4*dQ1*dQ2*m4*t9*t33*4.0+Lycm4*Lzcm4*dQ1*dQ3*m4*t9*t32*4.0+Lycm4*Lzcm4*dQ1*dQ3*m4*t9*t33*4.0-Lycm5*Lzcm5*dQ1*dQ4*m5*t10*t32*2.0-Lycm5*Lzcm5*dQ1*dQ4*m5*t10*t33*2.0-Lycm6*Lzcm6*dQ1*dQ5*m6*t11*t32*2.0-Lycm6*Lzcm6*dQ1*dQ5*m6*t11*t33*2.0-Lycm6*Lzcm6*dQ1*dQ5*m6*t11*t35*4.0-Lz6*Lzcm6*dQ2*dQ4*m6*t2*t8*4.0-Lz6*Lzcm6*dQ2*dQ4*m6*t3*t7*4.0-Lz6*Lzcm6*dQ3*dQ4*m6*t2*t8*4.0-Lz6*Lzcm6*dQ3*dQ4*m6*t3*t7*4.0;
et31 = Ixx4*dQ2*dQ3*t2*t3*t4*t9*-2.0+Ixx6*dQ2*dQ3*t2*t3*t4*t9*2.0+Ixx6*dQ2*dQ6*t2*t3*t4*t10+Ixx5*dQ4*dQ5*t2*t3*t5*t10*2.0+Ixx6*dQ3*dQ6*t2*t3*t4*t10+Ixx6*dQ5*dQ6*t2*t4*t5*t8+Ixx6*dQ5*dQ6*t3*t4*t5*t7+Ixx4*dQ2*dQ3*t4*t7*t8*t9*2.0-Ixx6*dQ4*dQ6*t2*t3*t6*t11*2.0-Ixx6*dQ2*dQ3*t4*t7*t8*t9*2.0-Ixx6*dQ1*dQ6*t2*t7*t9*t10*2.0-Ixx6*dQ1*dQ6*t3*t8*t9*t10*2.0-Ixx6*dQ2*dQ6*t4*t7*t8*t10-Ixx5*dQ4*dQ5*t5*t7*t8*t10*2.0-Ixx6*dQ3*dQ6*t4*t7*t8*t10-Ixx6*dQ1*dQ2*t6*t9*t10*t11*2.0+Ixx6*dQ4*dQ6*t2*t8*t9*t10+Ixx6*dQ4*dQ6*t3*t7*t9*t10-Ixx6*dQ1*dQ3*t6*t9*t10*t11*2.0+Ixx6*dQ4*dQ6*t6*t7*t8*t11*2.0-Ixx5*dQ1*dQ5*t2*t4*t7*t33*4.0;
et32 = Ixx5*dQ1*dQ5*t3*t4*t8*t32*-4.0-Ixx5*dQ1*dQ2*t4*t5*t10*t32*4.0-Ixx5*dQ1*dQ5*t2*t4*t7*t35*4.0-Ixx5*dQ1*dQ2*t4*t5*t10*t33*4.0-Ixx5*dQ1*dQ3*t4*t5*t10*t32*4.0-Ixx5*dQ1*dQ3*t4*t5*t10*t33*4.0-Ixx5*dQ1*dQ5*t3*t4*t8*t35*4.0-Ixx5*dQ2*dQ5*t2*t3*t9*t35*2.0+Ixx6*dQ1*dQ5*t2*t4*t7*t36*2.0-Ixx5*dQ3*dQ5*t2*t3*t9*t35*2.0+Ixx5*dQ4*dQ5*t2*t4*t8*t35*2.0+Ixx5*dQ4*dQ5*t3*t4*t7*t35*2.0+Ixx6*dQ1*dQ5*t3*t4*t8*t36*2.0+Ixx6*dQ1*dQ6*t4*t5*t9*t32*2.0+Ixx6*dQ2*dQ6*t2*t5*t8*t34*2.0+Ixx6*dQ2*dQ6*t3*t5*t7*t34*2.0+Ixx6*dQ1*dQ2*t4*t5*t10*t36*2.0+Ixx6*dQ1*dQ6*t4*t5*t9*t33*2.0+Ixx6*dQ3*dQ6*t2*t5*t8*t34*2.0+Ixx6*dQ3*dQ6*t3*t5*t7*t34*2.0+Ixx6*dQ1*dQ3*t4*t5*t10*t36*2.0;
et33 = Ixx6*dQ1*dQ4*t5*t6*t11*t32*2.0+Ixx6*dQ2*dQ6*t2*t5*t8*t36*2.0+Ixx6*dQ2*dQ6*t3*t5*t7*t36*2.0-Ixx6*dQ4*dQ5*t2*t4*t8*t36*2.0-Ixx6*dQ4*dQ5*t3*t4*t7*t36*2.0+Ixx6*dQ1*dQ4*t5*t6*t11*t33*2.0+Ixx6*dQ3*dQ6*t2*t5*t8*t36*2.0+Ixx6*dQ3*dQ6*t3*t5*t7*t36*2.0-Ixx6*dQ5*dQ6*t2*t3*t10*t36*2.0+Ixx5*dQ2*dQ5*t7*t8*t9*t35*2.0+Ixx5*dQ3*dQ5*t7*t8*t9*t35*2.0+Ixx6*dQ5*dQ6*t7*t8*t10*t36*2.0+Ixx4*dQ1*dQ2*t2*t7*t33*t34*4.0+Ixx4*dQ1*dQ2*t3*t8*t32*t34*4.0+Ixx4*dQ1*dQ3*t2*t7*t33*t34*4.0+Ixx4*dQ1*dQ3*t3*t8*t32*t34*4.0+Ixx5*dQ1*dQ2*t2*t7*t33*t35*4.0-Ixx6*dQ1*dQ2*t2*t7*t33*t34*4.0-Ixx5*dQ1*dQ2*t2*t7*t34*t35*2.0+Ixx5*dQ1*dQ2*t3*t8*t32*t35*4.0+Ixx5*dQ1*dQ3*t2*t7*t33*t35*4.0;
et34 = Ixx6*dQ1*dQ2*t3*t8*t32*t34*-4.0-Ixx6*dQ1*dQ3*t2*t7*t33*t34*4.0+Ixx4*dQ1*dQ4*t4*t9*t32*t33*4.0-Ixx5*dQ1*dQ3*t2*t7*t34*t35*2.0+Ixx5*dQ1*dQ3*t3*t8*t32*t35*4.0-Ixx6*dQ1*dQ2*t2*t7*t33*t36*8.0-Ixx6*dQ1*dQ3*t3*t8*t32*t34*4.0-Ixx5*dQ1*dQ2*t3*t8*t34*t35*2.0-Ixx6*dQ1*dQ2*t2*t7*t34*t36*2.0-Ixx6*dQ1*dQ2*t3*t8*t32*t36*8.0-Ixx6*dQ1*dQ3*t2*t7*t33*t36*8.0-Ixx5*dQ1*dQ3*t3*t8*t34*t35*2.0-Ixx6*dQ1*dQ2*t2*t7*t35*t36*2.0-Ixx6*dQ1*dQ3*t2*t7*t34*t36*2.0-Ixx6*dQ1*dQ3*t3*t8*t32*t36*8.0-Ixx6*dQ1*dQ4*t4*t9*t32*t33*4.0-Ixx5*dQ1*dQ4*t4*t9*t32*t35*2.0-Ixx5*dQ2*dQ4*t2*t8*t34*t35*2.0-Ixx5*dQ2*dQ4*t3*t7*t34*t35*2.0;
et35 = Ixx6*dQ1*dQ2*t3*t8*t34*t36*-2.0-Ixx6*dQ1*dQ3*t2*t7*t35*t36*2.0-Ixx5*dQ1*dQ4*t4*t9*t33*t35*2.0+Ixx5*dQ1*dQ5*t5*t10*t32*t33*4.0-Ixx5*dQ3*dQ4*t2*t8*t34*t35*2.0-Ixx5*dQ3*dQ4*t3*t7*t34*t35*2.0-Ixx6*dQ1*dQ2*t3*t8*t35*t36*2.0-Ixx6*dQ1*dQ3*t3*t8*t34*t36*2.0-Ixx5*dQ1*dQ5*t5*t10*t32*t34*2.0-Ixx6*dQ1*dQ3*t3*t8*t35*t36*2.0-Ixx6*dQ1*dQ4*t4*t9*t32*t36*2.0-Ixx6*dQ2*dQ4*t2*t8*t34*t36*2.0-Ixx6*dQ2*dQ4*t3*t7*t34*t36*2.0-Ixx5*dQ1*dQ5*t5*t10*t33*t34*2.0-Ixx6*dQ1*dQ4*t4*t9*t33*t36*2.0+Ixx6*dQ2*dQ4*t2*t8*t35*t36*2.0+Ixx6*dQ2*dQ4*t3*t7*t35*t36*2.0-Ixx6*dQ3*dQ4*t2*t8*t34*t36*2.0-Ixx6*dQ3*dQ4*t3*t7*t34*t36*2.0+Ixx6*dQ3*dQ4*t2*t8*t35*t36*2.0;
et36 = Ixx6*dQ3*dQ4*t3*t7*t35*t36*2.0-Ixx6*dQ1*dQ5*t5*t10*t32*t36*2.0-Ixx6*dQ1*dQ6*t6*t11*t32*t33*8.0-Ixx6*dQ1*dQ5*t5*t10*t33*t36*2.0-Ixx6*dQ1*dQ6*t6*t11*t32*t34*2.0-Ixx6*dQ1*dQ6*t6*t11*t32*t35*2.0-Ixx6*dQ1*dQ6*t6*t11*t33*t34*2.0-Ixx6*dQ1*dQ6*t6*t11*t33*t35*2.0+Iyy4*dQ2*dQ3*t2*t3*t4*t9*2.0+Iyy5*dQ2*dQ3*t2*t3*t4*t9*2.0-Iyy6*dQ2*dQ6*t2*t3*t4*t10-Iyy6*dQ3*dQ6*t2*t3*t4*t10+Iyy6*dQ4*dQ5*t2*t3*t5*t10*2.0-Iyy6*dQ5*dQ6*t2*t4*t5*t8-Iyy6*dQ5*dQ6*t3*t4*t5*t7-Iyy4*dQ2*dQ3*t4*t7*t8*t9*2.0-Iyy5*dQ2*dQ3*t4*t7*t8*t9*2.0+Iyy6*dQ4*dQ6*t2*t3*t6*t11*2.0+Iyy6*dQ1*dQ6*t2*t7*t9*t10*2.0+Iyy6*dQ1*dQ6*t3*t8*t9*t10*2.0;
et37 = Iyy6*dQ2*dQ6*t4*t7*t8*t10+Iyy6*dQ3*dQ6*t4*t7*t8*t10+Iyy6*dQ1*dQ2*t6*t9*t10*t11*2.0-Iyy6*dQ4*dQ5*t5*t7*t8*t10*2.0-Iyy6*dQ4*dQ6*t2*t8*t9*t10-Iyy6*dQ4*dQ6*t3*t7*t9*t10+Iyy6*dQ1*dQ3*t6*t9*t10*t11*2.0-Iyy6*dQ4*dQ6*t6*t7*t8*t11*2.0-Iyy6*dQ1*dQ5*t2*t4*t7*t33*4.0-Iyy6*dQ1*dQ5*t3*t4*t8*t32*4.0-Iyy6*dQ1*dQ2*t4*t5*t10*t32*4.0-Iyy6*dQ1*dQ5*t2*t4*t7*t35*4.0-Iyy6*dQ1*dQ2*t4*t5*t10*t33*4.0-Iyy6*dQ1*dQ3*t4*t5*t10*t32*4.0-Iyy6*dQ1*dQ5*t2*t4*t7*t36*2.0-Iyy6*dQ1*dQ3*t4*t5*t10*t33*4.0-Iyy6*dQ1*dQ5*t3*t4*t8*t35*4.0-Iyy6*dQ2*dQ5*t2*t3*t9*t35*2.0-Iyy6*dQ1*dQ5*t3*t4*t8*t36*2.0-Iyy6*dQ1*dQ6*t4*t5*t9*t32*2.0;
et38 = Iyy6*dQ2*dQ6*t2*t5*t8*t34*-2.0-Iyy6*dQ2*dQ6*t3*t5*t7*t34*2.0-Iyy6*dQ3*dQ5*t2*t3*t9*t35*2.0-Iyy6*dQ1*dQ2*t4*t5*t10*t36*2.0-Iyy6*dQ1*dQ6*t4*t5*t9*t33*2.0-Iyy6*dQ3*dQ6*t2*t5*t8*t34*2.0-Iyy6*dQ3*dQ6*t3*t5*t7*t34*2.0+Iyy6*dQ4*dQ5*t2*t4*t8*t35*2.0+Iyy6*dQ4*dQ5*t3*t4*t7*t35*2.0-Iyy6*dQ1*dQ3*t4*t5*t10*t36*2.0-Iyy6*dQ1*dQ4*t5*t6*t11*t32*2.0-Iyy6*dQ2*dQ6*t2*t5*t8*t36*2.0-Iyy6*dQ2*dQ6*t3*t5*t7*t36*2.0+Iyy6*dQ4*dQ5*t2*t4*t8*t36*2.0+Iyy6*dQ4*dQ5*t3*t4*t7*t36*2.0-Iyy6*dQ1*dQ4*t5*t6*t11*t33*2.0-Iyy6*dQ3*dQ6*t2*t5*t8*t36*2.0-Iyy6*dQ3*dQ6*t3*t5*t7*t36*2.0+Iyy6*dQ5*dQ6*t2*t3*t10*t36*2.0+Iyy6*dQ2*dQ5*t7*t8*t9*t35*2.0;
et39 = Iyy6*dQ3*dQ5*t7*t8*t9*t35*2.0-Iyy6*dQ5*dQ6*t7*t8*t10*t36*2.0-Iyy4*dQ1*dQ2*t2*t7*t33*t34*4.0-Iyy4*dQ1*dQ2*t3*t8*t32*t34*4.0-Iyy4*dQ1*dQ3*t2*t7*t33*t34*4.0-Iyy5*dQ1*dQ2*t2*t7*t33*t34*4.0-Iyy4*dQ1*dQ3*t3*t8*t32*t34*4.0-Iyy5*dQ1*dQ2*t3*t8*t32*t34*4.0-Iyy5*dQ1*dQ3*t2*t7*t33*t34*4.0-Iyy5*dQ1*dQ3*t3*t8*t32*t34*4.0+Iyy6*dQ1*dQ2*t2*t7*t33*t35*4.0-Iyy4*dQ1*dQ4*t4*t9*t32*t33*4.0+Iyy6*dQ1*dQ2*t2*t7*t33*t36*8.0-Iyy6*dQ1*dQ2*t2*t7*t34*t35*2.0+Iyy6*dQ1*dQ2*t3*t8*t32*t35*4.0+Iyy6*dQ1*dQ3*t2*t7*t33*t35*4.0-Iyy5*dQ1*dQ4*t4*t9*t32*t33*4.0+Iyy6*dQ1*dQ2*t2*t7*t34*t36*2.0+Iyy6*dQ1*dQ2*t3*t8*t32*t36*8.0+Iyy6*dQ1*dQ3*t2*t7*t33*t36*8.0;
et40 = Iyy6*dQ1*dQ3*t2*t7*t34*t35*-2.0+Iyy6*dQ1*dQ3*t3*t8*t32*t35*4.0+Iyy6*dQ1*dQ2*t2*t7*t35*t36*2.0-Iyy6*dQ1*dQ2*t3*t8*t34*t35*2.0+Iyy6*dQ1*dQ3*t2*t7*t34*t36*2.0+Iyy6*dQ1*dQ3*t3*t8*t32*t36*8.0+Iyy6*dQ1*dQ2*t3*t8*t34*t36*2.0+Iyy6*dQ1*dQ3*t2*t7*t35*t36*2.0-Iyy6*dQ1*dQ3*t3*t8*t34*t35*2.0+Iyy6*dQ1*dQ2*t3*t8*t35*t36*2.0+Iyy6*dQ1*dQ3*t3*t8*t34*t36*2.0-Iyy6*dQ1*dQ4*t4*t9*t32*t35*2.0-Iyy6*dQ2*dQ4*t2*t8*t34*t35*2.0-Iyy6*dQ2*dQ4*t3*t7*t34*t35*2.0+Iyy6*dQ1*dQ3*t3*t8*t35*t36*2.0+Iyy6*dQ1*dQ4*t4*t9*t32*t36*2.0-Iyy6*dQ1*dQ4*t4*t9*t33*t35*2.0+Iyy6*dQ1*dQ5*t5*t10*t32*t33*4.0+Iyy6*dQ2*dQ4*t2*t8*t34*t36*2.0+Iyy6*dQ2*dQ4*t3*t7*t34*t36*2.0-Iyy6*dQ3*dQ4*t2*t8*t34*t35*2.0;
et41 = Iyy6*dQ3*dQ4*t3*t7*t34*t35*-2.0+Iyy6*dQ1*dQ4*t4*t9*t33*t36*2.0-Iyy6*dQ1*dQ5*t5*t10*t32*t34*2.0-Iyy6*dQ2*dQ4*t2*t8*t35*t36*2.0-Iyy6*dQ2*dQ4*t3*t7*t35*t36*2.0+Iyy6*dQ3*dQ4*t2*t8*t34*t36*2.0+Iyy6*dQ3*dQ4*t3*t7*t34*t36*2.0-Iyy6*dQ1*dQ5*t5*t10*t33*t34*2.0-Iyy6*dQ3*dQ4*t2*t8*t35*t36*2.0-Iyy6*dQ3*dQ4*t3*t7*t35*t36*2.0+Iyy6*dQ1*dQ5*t5*t10*t32*t36*2.0+Iyy6*dQ1*dQ6*t6*t11*t32*t33*8.0+Iyy6*dQ1*dQ5*t5*t10*t33*t36*2.0+Iyy6*dQ1*dQ6*t6*t11*t32*t34*2.0+Iyy6*dQ1*dQ6*t6*t11*t32*t35*2.0+Iyy6*dQ1*dQ6*t6*t11*t33*t34*2.0+Iyy6*dQ1*dQ6*t6*t11*t33*t35*2.0-Izz5*dQ2*dQ3*t2*t3*t4*t9*2.0-Izz6*dQ2*dQ3*t2*t3*t4*t9*2.0-Izz6*dQ2*dQ6*t2*t3*t4*t10;
et42 = Izz5*dQ4*dQ5*t2*t3*t5*t10*-2.0-Izz6*dQ3*dQ6*t2*t3*t4*t10-Izz6*dQ4*dQ5*t2*t3*t5*t10*2.0-Izz6*dQ5*dQ6*t2*t4*t5*t8-Izz6*dQ5*dQ6*t3*t4*t5*t7+Izz5*dQ2*dQ3*t4*t7*t8*t9*2.0+Izz6*dQ2*dQ3*t4*t7*t8*t9*2.0+Izz6*dQ2*dQ6*t4*t7*t8*t10+Izz5*dQ4*dQ5*t5*t7*t8*t10*2.0+Izz6*dQ3*dQ6*t4*t7*t8*t10+Izz6*dQ4*dQ5*t5*t7*t8*t10*2.0+Izz6*dQ4*dQ6*t2*t8*t9*t10+Izz6*dQ4*dQ6*t3*t7*t9*t10+Izz5*dQ1*dQ5*t2*t4*t7*t33*4.0+Izz5*dQ1*dQ5*t3*t4*t8*t32*4.0+Izz6*dQ1*dQ5*t2*t4*t7*t33*4.0+Izz5*dQ1*dQ2*t4*t5*t10*t32*4.0+Izz5*dQ1*dQ5*t2*t4*t7*t35*4.0+Izz6*dQ1*dQ5*t3*t4*t8*t32*4.0+Izz5*dQ1*dQ2*t4*t5*t10*t33*4.0+Izz5*dQ1*dQ3*t4*t5*t10*t32*4.0+Izz6*dQ1*dQ2*t4*t5*t10*t32*4.0;
et43 = Izz6*dQ1*dQ5*t2*t4*t7*t35*4.0+Izz5*dQ1*dQ3*t4*t5*t10*t33*4.0+Izz5*dQ1*dQ5*t3*t4*t8*t35*4.0+Izz5*dQ2*dQ5*t2*t3*t9*t35*2.0+Izz6*dQ1*dQ2*t4*t5*t10*t33*4.0+Izz6*dQ1*dQ3*t4*t5*t10*t32*4.0+Izz5*dQ3*dQ5*t2*t3*t9*t35*2.0+Izz6*dQ1*dQ3*t4*t5*t10*t33*4.0+Izz6*dQ1*dQ5*t3*t4*t8*t35*4.0+Izz6*dQ2*dQ5*t2*t3*t9*t35*2.0-Izz5*dQ4*dQ5*t2*t4*t8*t35*2.0-Izz5*dQ4*dQ5*t3*t4*t7*t35*2.0+Izz6*dQ3*dQ5*t2*t3*t9*t35*2.0-Izz6*dQ4*dQ5*t2*t4*t8*t35*2.0-Izz6*dQ4*dQ5*t3*t4*t7*t35*2.0-Izz5*dQ2*dQ5*t7*t8*t9*t35*2.0-Izz5*dQ3*dQ5*t7*t8*t9*t35*2.0-Izz6*dQ2*dQ5*t7*t8*t9*t35*2.0-Izz6*dQ3*dQ5*t7*t8*t9*t35*2.0+Izz5*dQ1*dQ2*t2*t7*t33*t34*4.0-Izz5*dQ1*dQ2*t2*t7*t33*t35*4.0;
et44 = Izz5*dQ1*dQ2*t3*t8*t32*t34*4.0+Izz5*dQ1*dQ3*t2*t7*t33*t34*4.0+Izz6*dQ1*dQ2*t2*t7*t33*t34*4.0+Izz5*dQ1*dQ2*t2*t7*t34*t35*2.0-Izz5*dQ1*dQ2*t3*t8*t32*t35*4.0-Izz5*dQ1*dQ3*t2*t7*t33*t35*4.0+Izz5*dQ1*dQ3*t3*t8*t32*t34*4.0-Izz6*dQ1*dQ2*t2*t7*t33*t35*4.0+Izz6*dQ1*dQ2*t3*t8*t32*t34*4.0+Izz6*dQ1*dQ3*t2*t7*t33*t34*4.0+Izz5*dQ1*dQ3*t2*t7*t34*t35*2.0-Izz5*dQ1*dQ3*t3*t8*t32*t35*4.0+Izz6*dQ1*dQ2*t2*t7*t34*t35*2.0-Izz6*dQ1*dQ2*t3*t8*t32*t35*4.0-Izz6*dQ1*dQ3*t2*t7*t33*t35*4.0+Izz6*dQ1*dQ3*t3*t8*t32*t34*4.0+Izz5*dQ1*dQ2*t3*t8*t34*t35*2.0+Izz5*dQ1*dQ4*t4*t9*t32*t33*4.0+Izz6*dQ1*dQ3*t2*t7*t34*t35*2.0-Izz6*dQ1*dQ3*t3*t8*t32*t35*4.0+Izz5*dQ1*dQ3*t3*t8*t34*t35*2.0;
et45 = Izz6*dQ1*dQ2*t3*t8*t34*t35*2.0+Izz6*dQ1*dQ4*t4*t9*t32*t33*4.0+Izz5*dQ1*dQ4*t4*t9*t32*t35*2.0+Izz5*dQ2*dQ4*t2*t8*t34*t35*2.0+Izz5*dQ2*dQ4*t3*t7*t34*t35*2.0+Izz6*dQ1*dQ3*t3*t8*t34*t35*2.0+Izz5*dQ1*dQ4*t4*t9*t33*t35*2.0-Izz5*dQ1*dQ5*t5*t10*t32*t33*4.0+Izz5*dQ3*dQ4*t2*t8*t34*t35*2.0+Izz5*dQ3*dQ4*t3*t7*t34*t35*2.0+Izz6*dQ1*dQ4*t4*t9*t32*t35*2.0+Izz6*dQ2*dQ4*t2*t8*t34*t35*2.0+Izz6*dQ2*dQ4*t3*t7*t34*t35*2.0+Izz5*dQ1*dQ5*t5*t10*t32*t34*2.0+Izz6*dQ1*dQ4*t4*t9*t33*t35*2.0-Izz6*dQ1*dQ5*t5*t10*t32*t33*4.0+Izz6*dQ3*dQ4*t2*t8*t34*t35*2.0+Izz6*dQ3*dQ4*t3*t7*t34*t35*2.0+Izz5*dQ1*dQ5*t5*t10*t33*t34*2.0+Izz6*dQ1*dQ5*t5*t10*t32*t34*2.0+Izz6*dQ1*dQ5*t5*t10*t33*t34*2.0;
et46 = dQ1*dQ5*m5*t2*t4*t7*t17*-2.0-dQ1*dQ5*m5*t3*t4*t8*t17*2.0-dQ1*dQ2*m5*t4*t5*t10*t17*2.0-dQ1*dQ3*m5*t4*t5*t10*t17*2.0+dQ4*dQ5*m5*t2*t4*t8*t17*2.0+dQ4*dQ5*m5*t3*t4*t7*t17*2.0-dQ1*dQ5*m6*t2*t4*t7*t21*2.0+dQ1*dQ5*m6*t2*t4*t7*t22*2.0-dQ1*dQ5*m6*t3*t4*t8*t21*2.0-dQ1*dQ2*m6*t4*t5*t10*t21*2.0+dQ1*dQ5*m5*t2*t4*t7*t25*2.0+dQ1*dQ5*m6*t3*t4*t8*t22*2.0+dQ2*dQ5*m6*t2*t3*t9*t22*2.0+dQ1*dQ2*m6*t4*t5*t10*t22*2.0-dQ1*dQ3*m6*t4*t5*t10*t21*2.0-dQ2*dQ6*m6*t2*t5*t8*t21*2.0-dQ2*dQ6*m6*t3*t5*t7*t21*2.0+dQ3*dQ5*m6*t2*t3*t9*t22*2.0+dQ4*dQ5*m6*t2*t4*t8*t21*2.0+dQ4*dQ5*m6*t3*t4*t7*t21*2.0-dQ5*dQ6*m6*t2*t3*t10*t18*2.0;
et47 = dQ1*dQ3*m6*t4*t5*t10*t22*2.0+dQ1*dQ5*m5*t3*t4*t8*t25*2.0+dQ1*dQ5*m6*t2*t4*t7*t26*2.0+dQ2*dQ5*m5*t2*t3*t9*t25*2.0-dQ3*dQ6*m6*t2*t5*t8*t21*2.0-dQ3*dQ6*m6*t3*t5*t7*t21*2.0+dQ1*dQ2*m5*t4*t5*t10*t25*2.0+dQ3*dQ5*m5*t2*t3*t9*t25*2.0+dQ1*dQ3*m5*t4*t5*t10*t25*2.0+dQ1*dQ5*m6*t3*t4*t8*t26*2.0+dQ2*dQ5*m6*t2*t3*t9*t26*2.0+dQ1*dQ2*m6*t4*t5*t10*t26*2.0+dQ3*dQ5*m6*t2*t3*t9*t26*2.0+dQ1*dQ3*m6*t4*t5*t10*t26*2.0-dQ2*dQ5*m6*t7*t8*t9*t22*2.0-dQ3*dQ5*m6*t7*t8*t9*t22*2.0+dQ5*dQ6*m6*t7*t8*t10*t18*2.0-dQ1*dQ2*m3*t2*t7*t13*t33*4.0-dQ2*dQ5*m5*t7*t8*t9*t25*2.0-dQ1*dQ2*m3*t3*t8*t13*t32*4.0-dQ1*dQ2*m4*t2*t7*t13*t33*4.0;
et48 = dQ1*dQ3*m3*t2*t7*t13*t33*-4.0-dQ3*dQ5*m5*t7*t8*t9*t25*2.0-dQ1*dQ2*m3*t2*t7*t15*t33*4.0-dQ1*dQ2*m4*t3*t8*t13*t32*4.0-dQ1*dQ2*m5*t2*t7*t13*t33*4.0-dQ1*dQ3*m3*t3*t8*t13*t32*4.0-dQ1*dQ3*m4*t2*t7*t13*t33*4.0-dQ2*dQ5*m6*t7*t8*t9*t26*2.0-dQ1*dQ2*m3*t3*t8*t15*t32*4.0+dQ1*dQ2*m4*t2*t7*t14*t34*2.0-dQ1*dQ2*m5*t3*t8*t13*t32*4.0-dQ1*dQ2*m6*t2*t7*t13*t33*4.0-dQ1*dQ3*m3*t2*t7*t15*t33*4.0-dQ1*dQ3*m4*t3*t8*t13*t32*4.0-dQ1*dQ3*m5*t2*t7*t13*t33*4.0-dQ3*dQ5*m6*t7*t8*t9*t26*2.0+dQ1*dQ2*m5*t2*t7*t14*t34*2.0-dQ1*dQ2*m6*t3*t8*t13*t32*4.0-dQ1*dQ3*m3*t3*t8*t15*t32*4.0+dQ1*dQ3*m4*t2*t7*t14*t34*2.0;
et49 = dQ1*dQ3*m5*t3*t8*t13*t32*-4.0-dQ1*dQ3*m6*t2*t7*t13*t33*4.0+dQ1*dQ2*m4*t2*t7*t16*t34*2.0+dQ1*dQ2*m4*t3*t8*t14*t34*2.0+dQ1*dQ2*m6*t2*t7*t14*t34*2.0+dQ1*dQ3*m5*t2*t7*t14*t34*2.0-dQ1*dQ3*m6*t3*t8*t13*t32*4.0+dQ1*dQ2*m5*t2*t7*t17*t33*4.0+dQ1*dQ2*m5*t3*t8*t14*t34*2.0+dQ1*dQ3*m4*t2*t7*t16*t34*2.0+dQ1*dQ3*m4*t3*t8*t14*t34*2.0+dQ1*dQ3*m6*t2*t7*t14*t34*2.0-dQ1*dQ2*m4*t2*t7*t19*t33*4.0+dQ1*dQ2*m4*t3*t8*t16*t34*2.0+dQ1*dQ2*m5*t3*t8*t17*t32*4.0+dQ1*dQ2*m6*t3*t8*t14*t34*2.0+dQ1*dQ3*m5*t2*t7*t17*t33*4.0+dQ1*dQ3*m5*t3*t8*t14*t34*2.0+dQ1*dQ4*m4*t4*t9*t14*t32*2.0+dQ2*dQ4*m4*t2*t8*t14*t34*2.0+dQ2*dQ4*m4*t3*t7*t14*t34*2.0;
et50 = dQ1*dQ2*m4*t2*t7*t19*t34*-2.0-dQ1*dQ2*m4*t3*t8*t19*t32*4.0+dQ1*dQ2*m5*t2*t7*t17*t35*2.0-dQ1*dQ2*m6*t2*t7*t18*t33*4.0-dQ1*dQ3*m4*t2*t7*t19*t33*4.0+dQ1*dQ3*m4*t3*t8*t16*t34*2.0+dQ1*dQ3*m5*t3*t8*t17*t32*4.0+dQ1*dQ3*m6*t3*t8*t14*t34*2.0+dQ1*dQ4*m4*t4*t9*t14*t33*2.0+dQ1*dQ4*m5*t4*t9*t14*t32*2.0+dQ2*dQ4*m5*t2*t8*t14*t34*2.0+dQ2*dQ4*m5*t3*t7*t14*t34*2.0+dQ3*dQ4*m4*t2*t8*t14*t34*2.0+dQ3*dQ4*m4*t3*t7*t14*t34*2.0-dQ1*dQ2*m5*t2*t7*t20*t33*4.0-dQ1*dQ2*m6*t2*t7*t18*t34*2.0-dQ1*dQ2*m6*t3*t8*t18*t32*4.0-dQ1*dQ3*m4*t2*t7*t19*t34*2.0-dQ1*dQ3*m4*t3*t8*t19*t32*4.0+dQ1*dQ3*m5*t2*t7*t17*t35*2.0-dQ1*dQ3*m6*t2*t7*t18*t33*4.0;
et51 = dQ1*dQ4*m4*t4*t9*t16*t32*2.0+dQ1*dQ4*m5*t4*t9*t14*t33*2.0+dQ1*dQ4*m6*t4*t9*t14*t32*2.0+dQ2*dQ4*m4*t2*t8*t16*t34*2.0+dQ2*dQ4*m4*t3*t7*t16*t34*2.0+dQ2*dQ4*m6*t2*t8*t14*t34*2.0+dQ2*dQ4*m6*t3*t7*t14*t34*2.0+dQ3*dQ4*m5*t2*t8*t14*t34*2.0+dQ3*dQ4*m5*t3*t7*t14*t34*2.0+dQ1*dQ2*m3*t2*t7*t23*t33*4.0-dQ1*dQ2*m4*t3*t8*t19*t34*2.0-dQ1*dQ2*m5*t2*t7*t20*t34*2.0+dQ1*dQ2*m5*t3*t8*t17*t35*2.0-dQ1*dQ2*m5*t3*t8*t20*t32*4.0-dQ1*dQ3*m5*t2*t7*t20*t33*4.0-dQ1*dQ3*m6*t2*t7*t18*t34*2.0-dQ1*dQ3*m6*t3*t8*t18*t32*4.0+dQ1*dQ4*m4*t4*t9*t16*t33*2.0+dQ1*dQ4*m6*t4*t9*t14*t33*2.0+dQ3*dQ4*m4*t2*t8*t16*t34*2.0+dQ3*dQ4*m4*t3*t7*t16*t34*2.0;
et52 = dQ3*dQ4*m6*t2*t8*t14*t34*2.0+dQ3*dQ4*m6*t3*t7*t14*t34*2.0+dQ1*dQ2*m3*t3*t8*t23*t32*4.0-dQ1*dQ2*m6*t2*t7*t18*t36*4.0+dQ1*dQ2*m6*t2*t7*t21*t33*4.0-dQ1*dQ2*m6*t3*t8*t18*t34*2.0+dQ1*dQ3*m3*t2*t7*t23*t33*4.0-dQ1*dQ3*m4*t3*t8*t19*t34*2.0-dQ1*dQ3*m5*t2*t7*t20*t34*2.0+dQ1*dQ3*m5*t3*t8*t17*t35*2.0-dQ1*dQ3*m5*t3*t8*t20*t32*4.0+dQ1*dQ2*m4*t2*t7*t24*t33*4.0-dQ1*dQ2*m5*t3*t8*t20*t34*2.0+dQ1*dQ2*m6*t3*t8*t21*t32*4.0+dQ1*dQ3*m3*t3*t8*t23*t32*4.0-dQ1*dQ3*m6*t2*t7*t18*t36*4.0+dQ1*dQ3*m6*t2*t7*t21*t33*4.0-dQ1*dQ3*m6*t3*t8*t18*t34*2.0-dQ1*dQ4*m4*t4*t9*t19*t32*2.0-dQ2*dQ4*m4*t2*t8*t19*t34*2.0-dQ2*dQ4*m4*t3*t7*t19*t34*2.0;
et53 = dQ2*dQ4*m5*t2*t8*t17*t35*-2.0-dQ2*dQ4*m5*t3*t7*t17*t35*2.0+dQ1*dQ2*m4*t3*t8*t24*t32*4.0+dQ1*dQ2*m6*t2*t7*t21*t35*2.0+dQ1*dQ2*m6*t2*t7*t22*t34*2.0-dQ1*dQ2*m6*t3*t8*t18*t36*4.0+dQ1*dQ3*m4*t2*t7*t24*t33*4.0-dQ1*dQ3*m5*t3*t8*t20*t34*2.0+dQ1*dQ3*m6*t3*t8*t21*t32*4.0-dQ1*dQ4*m4*t4*t9*t19*t33*2.0-dQ1*dQ4*m6*t4*t9*t18*t32*2.0-dQ2*dQ4*m6*t2*t8*t18*t34*2.0-dQ2*dQ4*m6*t3*t7*t18*t34*2.0-dQ3*dQ4*m4*t2*t8*t19*t34*2.0-dQ3*dQ4*m4*t3*t7*t19*t34*2.0-dQ3*dQ4*m5*t2*t8*t17*t35*2.0-dQ3*dQ4*m5*t3*t7*t17*t35*2.0+dQ1*dQ2*m6*t2*t7*t21*t36*4.0-dQ1*dQ2*m6*t2*t7*t22*t35*2.0+dQ1*dQ3*m4*t3*t8*t24*t32*4.0;
et54 = dQ1*dQ3*m6*t2*t7*t21*t35*2.0+dQ1*dQ3*m6*t2*t7*t22*t34*2.0-dQ1*dQ3*m6*t3*t8*t18*t36*4.0-dQ1*dQ4*m5*t4*t9*t20*t32*2.0-dQ1*dQ4*m6*t4*t9*t18*t33*2.0+dQ1*dQ5*m5*t5*t10*t17*t32*2.0-dQ2*dQ4*m5*t2*t8*t20*t34*2.0-dQ2*dQ4*m5*t3*t7*t20*t34*2.0-dQ3*dQ4*m6*t2*t8*t18*t34*2.0-dQ3*dQ4*m6*t3*t7*t18*t34*2.0+dQ1*dQ2*m5*t2*t7*t25*t34*2.0+dQ1*dQ2*m6*t3*t8*t21*t35*2.0+dQ1*dQ2*m6*t3*t8*t22*t34*2.0+dQ1*dQ3*m6*t2*t7*t21*t36*4.0-dQ1*dQ3*m6*t2*t7*t22*t35*2.0-dQ1*dQ4*m5*t4*t9*t20*t33*2.0+dQ1*dQ5*m5*t5*t10*t17*t33*2.0-dQ3*dQ4*m5*t2*t8*t20*t34*2.0-dQ3*dQ4*m5*t3*t7*t20*t34*2.0-dQ1*dQ2*m5*t2*t7*t25*t35*2.0;
et55 = dQ1*dQ2*m6*t3*t8*t21*t36*4.0-dQ1*dQ2*m6*t3*t8*t22*t35*2.0+dQ1*dQ3*m5*t2*t7*t25*t34*2.0+dQ1*dQ3*m6*t3*t8*t21*t35*2.0+dQ1*dQ3*m6*t3*t8*t22*t34*2.0+dQ1*dQ2*m5*t3*t8*t25*t34*2.0+dQ1*dQ2*m6*t2*t7*t26*t34*2.0-dQ1*dQ3*m5*t2*t7*t25*t35*2.0+dQ1*dQ3*m6*t3*t8*t21*t36*4.0-dQ1*dQ3*m6*t3*t8*t22*t35*2.0+dQ1*dQ4*m6*t4*t9*t22*t32*2.0-dQ2*dQ4*m6*t2*t8*t21*t35*2.0+dQ2*dQ4*m6*t2*t8*t22*t34*2.0-dQ2*dQ4*m6*t3*t7*t21*t35*2.0+dQ2*dQ4*m6*t3*t7*t22*t34*2.0-dQ1*dQ2*m5*t3*t8*t25*t35*2.0-dQ1*dQ2*m6*t2*t7*t26*t35*2.0+dQ1*dQ3*m5*t3*t8*t25*t34*2.0+dQ1*dQ3*m6*t2*t7*t26*t34*2.0+dQ1*dQ4*m6*t4*t9*t22*t33*2.0+dQ2*dQ4*m6*t2*t8*t22*t35*2.0;
et56 = dQ2*dQ4*m6*t3*t7*t22*t35*2.0-dQ3*dQ4*m6*t2*t8*t21*t35*2.0+dQ3*dQ4*m6*t2*t8*t22*t34*2.0-dQ3*dQ4*m6*t3*t7*t21*t35*2.0+dQ3*dQ4*m6*t3*t7*t22*t34*2.0+dQ1*dQ2*m6*t3*t8*t26*t34*2.0-dQ1*dQ3*m5*t3*t8*t25*t35*2.0-dQ1*dQ3*m6*t2*t7*t26*t35*2.0+dQ1*dQ4*m5*t4*t9*t25*t32*2.0+dQ1*dQ5*m6*t5*t10*t21*t32*2.0-dQ1*dQ6*m6*t6*t11*t18*t32*4.0+dQ2*dQ4*m5*t2*t8*t25*t34*2.0+dQ2*dQ4*m5*t3*t7*t25*t34*2.0+dQ3*dQ4*m6*t2*t8*t22*t35*2.0+dQ3*dQ4*m6*t3*t7*t22*t35*2.0-dQ1*dQ2*m6*t3*t8*t26*t35*2.0+dQ1*dQ3*m6*t3*t8*t26*t34*2.0+dQ1*dQ4*m5*t4*t9*t25*t33*2.0-dQ1*dQ5*m6*t5*t10*t18*t36*2.0+dQ1*dQ5*m6*t5*t10*t21*t33*2.0-dQ1*dQ5*m6*t5*t10*t22*t32*2.0;
et57 = dQ1*dQ6*m6*t6*t11*t18*t33*-4.0+dQ2*dQ4*m5*t2*t8*t25*t35*2.0+dQ2*dQ4*m5*t3*t7*t25*t35*2.0+dQ3*dQ4*m5*t2*t8*t25*t34*2.0+dQ3*dQ4*m5*t3*t7*t25*t34*2.0-dQ1*dQ3*m6*t3*t8*t26*t35*2.0+dQ1*dQ4*m6*t4*t9*t26*t32*2.0-dQ1*dQ5*m6*t5*t10*t22*t33*2.0+dQ2*dQ4*m6*t2*t8*t26*t34*2.0+dQ2*dQ4*m6*t3*t7*t26*t34*2.0+dQ3*dQ4*m5*t2*t8*t25*t35*2.0+dQ3*dQ4*m5*t3*t7*t25*t35*2.0+dQ1*dQ4*m6*t4*t9*t26*t33*2.0-dQ1*dQ5*m5*t5*t10*t25*t32*2.0-dQ1*dQ6*m6*t6*t11*t18*t35*2.0+dQ1*dQ6*m6*t6*t11*t21*t32*4.0+dQ2*dQ4*m6*t2*t8*t26*t35*2.0+dQ2*dQ4*m6*t3*t7*t26*t35*2.0+dQ3*dQ4*m6*t2*t8*t26*t34*2.0+dQ3*dQ4*m6*t3*t7*t26*t34*2.0-dQ1*dQ5*m5*t5*t10*t25*t33*2.0;
et58 = dQ1*dQ5*m6*t5*t10*t21*t36*2.0+dQ1*dQ6*m6*t6*t11*t21*t33*4.0+dQ3*dQ4*m6*t2*t8*t26*t35*2.0+dQ3*dQ4*m6*t3*t7*t26*t35*2.0-dQ1*dQ5*m6*t5*t10*t26*t32*2.0-dQ1*dQ5*m6*t5*t10*t26*t33*2.0+dQ1*dQ6*m6*t6*t11*t21*t35*2.0-t3*t5*t6*t7*t11*t34*t84*8.0+t3*t5*t6*t7*t11*t34*t92*8.0-t3*t4*t7*t9*t35*t36*t84*4.0+t3*t4*t7*t9*t35*t36*t92*4.0+t4*t6*t7*t8*t10*t11*t148*4.0-t4*t6*t7*t8*t10*t11*t152*4.0-Lx2*Lx3*dQ1*dQ2*m3*t2*t3*t7*4.0-Lx2*Lx3*dQ1*dQ2*m4*t2*t3*t7*4.0-Lx2*Lx3*dQ1*dQ3*m3*t2*t3*t7*2.0-Lx2*Lx3*dQ1*dQ2*m5*t2*t3*t7*4.0-Lx2*Lx3*dQ1*dQ3*m4*t2*t3*t7*2.0-Lx2*Lx3*dQ1*dQ2*m6*t2*t3*t7*4.0;
et59 = Lx2*Lx3*dQ1*dQ3*m5*t2*t3*t7*-2.0-Lx2*Lx3*dQ1*dQ3*m6*t2*t3*t7*2.0+Lx3*Lx4*dQ1*dQ2*m4*t2*t4*t7*4.0+Lx3*Lx4*dQ1*dQ2*m5*t2*t4*t7*4.0+Lx3*Lx4*dQ1*dQ3*m4*t2*t4*t7*4.0+Lx3*Lx4*dQ1*dQ2*m4*t3*t4*t8*4.0+Lx3*Lx4*dQ1*dQ2*m6*t2*t4*t7*4.0+Lx3*Lx4*dQ1*dQ3*m5*t2*t4*t7*4.0+Lx3*Lx4*dQ1*dQ2*m5*t3*t4*t8*4.0+Lx3*Lx4*dQ1*dQ3*m4*t3*t4*t8*4.0+Lx3*Lx4*dQ1*dQ3*m6*t2*t4*t7*4.0+Lx3*Lx4*dQ2*dQ3*m4*t2*t3*t9*2.0+Lx3*Lx4*dQ1*dQ2*m6*t3*t4*t8*4.0+Lx3*Lx4*dQ1*dQ3*m5*t3*t4*t8*4.0+Lx3*Lx4*dQ2*dQ3*m5*t2*t3*t9*2.0+Lx3*Lx4*dQ1*dQ3*m6*t3*t4*t8*4.0+Lx3*Lx4*dQ2*dQ3*m6*t2*t3*t9*2.0-Lx3*Lx4*dQ2*dQ3*m4*t7*t8*t9*2.0-Lx3*Lx4*dQ2*dQ3*m5*t7*t8*t9*2.0;
et60 = Lx3*Lx4*dQ2*dQ3*m6*t7*t8*t9*-2.0-Lx2*Lx4*dQ1*dQ2*m4*t4*t8*t32*4.0-Lx2*Lx4*dQ1*dQ2*m5*t4*t8*t32*4.0-Lx2*Lx4*dQ1*dQ3*m4*t4*t8*t32*2.0-Lx2*Lx4*dQ1*dQ2*m6*t4*t8*t32*4.0-Lx2*Lx4*dQ1*dQ3*m5*t4*t8*t32*2.0-Lx2*Lx4*dQ1*dQ4*m4*t3*t9*t32*2.0-Lx2*Lx4*dQ1*dQ3*m6*t4*t8*t32*2.0-Lx2*Lx4*dQ1*dQ4*m5*t3*t9*t32*2.0-Lx2*Lx4*dQ1*dQ4*m6*t3*t9*t32*2.0-Lx3*Lx4*dQ1*dQ4*m4*t9*t32*t33*4.0-Lx3*Lx4*dQ1*dQ4*m5*t9*t32*t33*4.0-Lx3*Lx4*dQ1*dQ4*m6*t9*t32*t33*4.0-Lx2*Lxcm3*dQ1*dQ2*m3*t2*t3*t7*4.0-Lx2*Lxcm3*dQ1*dQ3*m3*t2*t3*t7*2.0+Lx3*Lxcm4*dQ1*dQ2*m4*t2*t4*t7*4.0+Lx3*Lxcm4*dQ1*dQ3*m4*t2*t4*t7*4.0+Lx3*Lxcm4*dQ1*dQ2*m4*t3*t4*t8*4.0;
et61 = Lx3*Lxcm4*dQ1*dQ3*m4*t3*t4*t8*4.0+Lx3*Lxcm4*dQ2*dQ3*m4*t2*t3*t9*2.0+Lx2*Lxcm5*dQ1*dQ2*m5*t4*t5*t8*2.0+Lx3*Lxcm5*dQ1*dQ5*m5*t2*t5*t7*2.0+Lx3*Lxcm5*dQ1*dQ5*m5*t3*t5*t8*2.0-Lx4*Lxcm5*dQ2*dQ4*m5*t2*t5*t8*4.0-Lx4*Lxcm5*dQ2*dQ4*m5*t3*t5*t7*4.0+Lx2*Lxcm6*dQ1*dQ2*m6*t3*t6*t10*2.0-Lx4*Lxcm5*dQ3*dQ4*m5*t2*t5*t8*4.0-Lx4*Lxcm5*dQ3*dQ4*m5*t3*t5*t7*4.0-Lx2*Lxcm5*dQ4*dQ5*m5*t2*t4*t10*2.0-Lx4*Lxcm6*dQ2*dQ3*m6*t2*t3*t11*2.0-Lx4*Lxcm5*dQ4*dQ5*m5*t2*t3*t10*2.0-Lx4*Lxcm6*dQ1*dQ2*m6*t4*t6*t10*2.0-Lx3*Lxcm4*dQ2*dQ3*m4*t7*t8*t9*2.0-Lx3*Lxcm6*dQ1*dQ4*m6*t5*t6*t9*2.0-Lx4*Lxcm6*dQ1*dQ3*m6*t4*t6*t10*2.0-Lx4*Lxcm6*dQ2*dQ6*m6*t2*t6*t8*2.0;
et62 = Lx4*Lxcm6*dQ2*dQ6*m6*t3*t6*t7*-2.0-Lx2*Lxcm6*dQ4*dQ6*m6*t2*t6*t9*2.0-Lx3*Lxcm6*dQ1*dQ5*m6*t4*t6*t10*2.0-Lx4*Lxcm6*dQ3*dQ6*m6*t2*t6*t8*2.0-Lx4*Lxcm6*dQ3*dQ6*m6*t3*t6*t7*2.0-Lx3*Lxcm6*dQ1*dQ6*m6*t4*t5*t11*2.0-Lx2*Lxcm6*dQ1*dQ2*m6*t8*t9*t11*2.0+Lx4*Lxcm6*dQ2*dQ3*m6*t7*t8*t11*2.0+Lx4*Lxcm5*dQ4*dQ5*m5*t7*t8*t10*2.0-Lx3*Lxcm3*dQ1*dQ2*m3*t2*t7*t33*8.0-Lx3*Lxcm3*dQ1*dQ2*m3*t3*t8*t32*8.0-Lx3*Lxcm3*dQ1*dQ3*m3*t2*t7*t33*8.0-Lx3*Lxcm3*dQ1*dQ3*m3*t3*t8*t32*8.0-Lx2*Lxcm4*dQ1*dQ2*m4*t4*t8*t32*4.0-Lx2*Lxcm4*dQ1*dQ3*m4*t4*t8*t32*2.0+Lx4*Lxcm4*dQ1*dQ2*m4*t2*t7*t34*4.0-Lx2*Lxcm4*dQ1*dQ4*m4*t3*t9*t32*2.0+Lx4*Lxcm4*dQ1*dQ3*m4*t2*t7*t34*4.0;
et63 = Lx2*Lxcm5*dQ1*dQ2*m5*t3*t10*t32*-4.0+Lx4*Lxcm4*dQ1*dQ2*m4*t3*t8*t34*4.0-Lx2*Lxcm5*dQ1*dQ3*m5*t3*t10*t32*2.0+Lx4*Lxcm4*dQ1*dQ3*m4*t3*t8*t34*4.0+Lx4*Lxcm4*dQ1*dQ4*m4*t4*t9*t32*4.0+Lx4*Lxcm4*dQ2*dQ4*m4*t2*t8*t34*4.0+Lx4*Lxcm4*dQ2*dQ4*m4*t3*t7*t34*4.0-Lx2*Lxcm5*dQ1*dQ5*m5*t5*t8*t32*2.0+Lx4*Lxcm4*dQ1*dQ4*m4*t4*t9*t33*4.0+Lx4*Lxcm4*dQ3*dQ4*m4*t2*t8*t34*4.0+Lx4*Lxcm4*dQ3*dQ4*m4*t3*t7*t34*4.0+Lx4*Lxcm5*dQ1*dQ2*m5*t4*t10*t32*4.0+Lx3*Lxcm5*dQ1*dQ4*m5*t5*t9*t32*2.0+Lx4*Lxcm5*dQ1*dQ2*m5*t4*t10*t33*4.0+Lx4*Lxcm5*dQ1*dQ3*m5*t4*t10*t32*4.0+Lx3*Lxcm5*dQ1*dQ4*m5*t5*t9*t33*2.0+Lx3*Lxcm5*dQ1*dQ5*m5*t4*t10*t32*2.0+Lx4*Lxcm5*dQ1*dQ3*m5*t4*t10*t33*4.0+Lx3*Lxcm5*dQ1*dQ5*m5*t4*t10*t33*2.0;
et64 = Lx3*Lxcm6*dQ1*dQ2*m6*t6*t10*t32*4.0+Lx3*Lxcm6*dQ1*dQ2*m6*t6*t10*t33*4.0+Lx3*Lxcm6*dQ1*dQ3*m6*t6*t10*t32*4.0+Lx3*Lxcm6*dQ1*dQ4*m6*t4*t11*t32*2.0+Lx3*Lxcm6*dQ1*dQ3*m6*t6*t10*t33*4.0+Lx3*Lxcm6*dQ1*dQ4*m6*t4*t11*t33*2.0+Lx3*Lxcm6*dQ1*dQ6*m6*t6*t9*t32*2.0+Lx3*Lxcm6*dQ1*dQ6*m6*t6*t9*t33*2.0-Lx3*Lxcm4*dQ1*dQ4*m4*t9*t32*t33*4.0-Lx3*Lxcm5*dQ1*dQ2*m5*t10*t32*t33*8.0-Lx3*Lxcm5*dQ1*dQ3*m5*t10*t32*t33*8.0+Lx4*Lxcm5*dQ1*dQ5*m5*t10*t32*t34*2.0+Lx4*Lxcm5*dQ1*dQ5*m5*t10*t33*t34*2.0+Lx4*Lxcm6*dQ1*dQ4*m6*t11*t32*t33*4.0+Lx4*Lxcm6*dQ1*dQ4*m6*t11*t32*t34*4.0+Lx4*Lxcm6*dQ1*dQ4*m6*t11*t33*t34*4.0+Lx3*Lycm4*dQ2*dQ3*m4*t2*t3*t4*2.0+Lx3*Lycm5*dQ2*dQ3*m5*t2*t3*t4*2.0-Lx3*Lycm4*dQ1*dQ2*m4*t2*t7*t9*4.0;
et65 = Lx4*Lycm6*dQ2*dQ3*m6*t2*t3*t6*-2.0-Lx3*Lycm4*dQ1*dQ3*m4*t2*t7*t9*4.0-Lx3*Lycm4*dQ1*dQ2*m4*t3*t8*t9*4.0-Lx3*Lycm5*dQ1*dQ2*m5*t2*t7*t9*4.0-Lx3*Lycm4*dQ1*dQ3*m4*t3*t8*t9*4.0-Lx3*Lycm4*dQ2*dQ3*m4*t4*t7*t8*2.0-Lx3*Lycm5*dQ1*dQ3*m5*t2*t7*t9*4.0-Lx3*Lycm5*dQ1*dQ2*m5*t3*t8*t9*4.0-Lx3*Lycm5*dQ1*dQ3*m5*t3*t8*t9*4.0-Lx3*Lycm5*dQ2*dQ3*m5*t4*t7*t8*2.0-Lx3*Lycm6*dQ1*dQ6*m6*t4*t5*t6*2.0-Lx2*Lycm6*dQ1*dQ2*m6*t6*t8*t9*2.0-Lx2*Lycm6*dQ1*dQ2*m6*t3*t10*t11*2.0+Lx4*Lycm6*dQ2*dQ3*m6*t6*t7*t8*2.0+Lx4*Lycm6*dQ1*dQ2*m6*t4*t10*t11*2.0+Lx3*Lycm6*dQ1*dQ4*m6*t5*t9*t11*2.0+Lx4*Lycm6*dQ1*dQ3*m6*t4*t10*t11*2.0+Lx4*Lycm6*dQ2*dQ6*m6*t2*t8*t11*2.0;
et66 = Lx4*Lycm6*dQ2*dQ6*m6*t3*t7*t11*2.0+Lx2*Lycm6*dQ4*dQ6*m6*t2*t9*t11*2.0+Lx3*Lycm6*dQ1*dQ5*m6*t4*t10*t11*2.0+Lx4*Lycm6*dQ3*dQ6*m6*t2*t8*t11*2.0+Lx4*Lycm6*dQ3*dQ6*m6*t3*t7*t11*2.0-Lx2*Lycm4*dQ1*dQ4*m4*t3*t4*t32*2.0-Lx2*Lycm5*dQ1*dQ4*m5*t3*t4*t32*2.0+Lx4*Lycm4*dQ2*dQ3*m4*t2*t3*t34*4.0+Lx4*Lycm5*dQ2*dQ3*m5*t2*t3*t34*4.0+Lx2*Lycm4*dQ1*dQ2*m4*t8*t9*t32*4.0+Lx3*Lycm6*dQ1*dQ4*m6*t4*t6*t32*2.0+Lx2*Lycm4*dQ1*dQ3*m4*t8*t9*t32*2.0+Lx3*Lycm6*dQ1*dQ4*m6*t4*t6*t33*2.0+Lx2*Lycm5*dQ1*dQ2*m5*t8*t9*t32*4.0+Lx2*Lycm5*dQ1*dQ3*m5*t8*t9*t32*2.0-Lx4*Lycm4*dQ2*dQ3*m4*t7*t8*t34*4.0-Lx4*Lycm5*dQ2*dQ3*m5*t7*t8*t34*4.0-Lx3*Lycm6*dQ1*dQ2*m6*t10*t11*t32*4.0-Lx3*Lycm6*dQ1*dQ2*m6*t10*t11*t33*4.0;
et67 = Lx3*Lycm6*dQ1*dQ3*m6*t10*t11*t32*-4.0-Lx3*Lycm6*dQ1*dQ3*m6*t10*t11*t33*4.0-Lx3*Lycm6*dQ1*dQ6*m6*t9*t11*t32*2.0-Lx3*Lycm6*dQ1*dQ6*m6*t9*t11*t33*2.0-Lx3*Lycm4*dQ1*dQ4*m4*t4*t32*t33*4.0-Lx3*Lycm5*dQ1*dQ4*m5*t4*t32*t33*4.0+Lx4*Lycm6*dQ1*dQ4*m6*t6*t32*t33*4.0+Lx4*Lycm6*dQ1*dQ4*m6*t6*t32*t34*4.0+Lx4*Lycm6*dQ1*dQ4*m6*t6*t33*t34*4.0-Lx4*Lycm4*dQ1*dQ4*m4*t32*t33*t34*8.0-Lx4*Lycm5*dQ1*dQ4*m5*t32*t33*t34*8.0-Lxcm5*Lycm5*dQ2*dQ3*m5*t2*t3*t5*2.0+Lxcm6*Lycm6*dQ2*dQ3*m6*t2*t3*t5*2.0+Lxcm5*Lycm5*dQ2*dQ3*m5*t5*t7*t8*2.0-Lxcm6*Lycm6*dQ2*dQ3*m6*t5*t7*t8*2.0+Lxcm6*Lycm6*dQ5*dQ6*m6*t2*t8*t9*2.0+Lxcm6*Lycm6*dQ5*dQ6*m6*t3*t7*t9*2.0+Lxcm4*Lycm4*dQ2*dQ3*m4*t2*t3*t34*4.0;
et68 = Lxcm4*Lycm4*dQ2*dQ3*m4*t7*t8*t34*-4.0+Lxcm6*Lycm6*dQ4*dQ6*m6*t2*t3*t35*2.0-Lxcm5*Lycm5*dQ1*dQ2*m5*t9*t10*t32*4.0+Lxcm6*Lycm6*dQ4*dQ6*m6*t2*t3*t36*4.0-Lxcm5*Lycm5*dQ1*dQ2*m5*t9*t10*t33*4.0-Lxcm5*Lycm5*dQ1*dQ3*m5*t9*t10*t32*4.0-Lxcm5*Lycm5*dQ1*dQ3*m5*t9*t10*t33*4.0+Lxcm6*Lycm6*dQ1*dQ2*m6*t9*t10*t32*4.0+Lxcm6*Lycm6*dQ1*dQ2*m6*t9*t10*t33*4.0+Lxcm6*Lycm6*dQ1*dQ3*m6*t9*t10*t32*4.0+Lxcm6*Lycm6*dQ1*dQ3*m6*t9*t10*t33*4.0+Lxcm6*Lycm6*dQ1*dQ2*m6*t9*t10*t36*4.0+Lxcm6*Lycm6*dQ1*dQ3*m6*t9*t10*t36*4.0-Lxcm6*Lycm6*dQ4*dQ6*m6*t7*t8*t35*2.0-Lxcm6*Lycm6*dQ4*dQ6*m6*t7*t8*t36*4.0+Lxcm5*Lycm5*dQ1*dQ4*m5*t5*t32*t33*4.0+Lxcm5*Lycm5*dQ1*dQ4*m5*t5*t32*t34*4.0+Lxcm5*Lycm5*dQ1*dQ4*m5*t5*t33*t34*4.0-Lxcm6*Lycm6*dQ1*dQ4*m6*t5*t32*t33*4.0;
et69 = Lxcm6*Lycm6*dQ1*dQ4*m6*t5*t32*t34*-4.0-Lxcm6*Lycm6*dQ1*dQ4*m6*t5*t33*t34*4.0-Lxcm6*Lycm6*dQ1*dQ4*m6*t5*t32*t36*4.0-Lxcm6*Lycm6*dQ1*dQ4*m6*t5*t33*t36*4.0-Lxcm4*Lycm4*dQ1*dQ4*m4*t32*t33*t34*8.0+Lxcm6*Lycm6*dQ1*dQ6*m6*t32*t33*t34*4.0+Lxcm6*Lycm6*dQ1*dQ6*m6*t32*t33*t35*4.0+Lxcm6*Lycm6*dQ1*dQ6*m6*t32*t33*t36*1.6e+1-Lxcm6*Lycm6*dQ1*dQ6*m6*t32*t34*t35*2.0+Lxcm6*Lycm6*dQ1*dQ6*m6*t32*t34*t36*4.0-Lxcm6*Lycm6*dQ1*dQ6*m6*t33*t34*t35*2.0+Lxcm6*Lycm6*dQ1*dQ6*m6*t32*t35*t36*4.0+Lxcm6*Lycm6*dQ1*dQ6*m6*t33*t34*t36*4.0+Lxcm6*Lycm6*dQ1*dQ6*m6*t33*t35*t36*4.0+Lx2*Lz6*dQ4*dQ5*m6*t2*t4*t5*2.0+Lx4*Lz6*dQ4*dQ5*m6*t2*t3*t5*2.0+Lx2*Lz6*dQ1*dQ2*m6*t4*t8*t10*2.0+Lx3*Lz6*dQ1*dQ5*m6*t2*t7*t10*2.0+Lx3*Lz6*dQ1*dQ5*m6*t3*t8*t10*2.0;
et70 = Lx4*Lz6*dQ2*dQ4*m6*t2*t8*t10*-4.0-Lx4*Lz6*dQ2*dQ4*m6*t3*t7*t10*4.0-Lx4*Lz6*dQ3*dQ4*m6*t2*t8*t10*4.0-Lx4*Lz6*dQ3*dQ4*m6*t3*t7*t10*4.0-Lx4*Lz6*dQ4*dQ5*m6*t5*t7*t8*2.0+Lx2*Lz6*dQ1*dQ2*m6*t3*t5*t32*4.0+Lx2*Lz6*dQ1*dQ3*m6*t3*t5*t32*2.0-Lx4*Lz6*dQ1*dQ2*m6*t4*t5*t32*4.0-Lx4*Lz6*dQ1*dQ2*m6*t4*t5*t33*4.0-Lx4*Lz6*dQ1*dQ3*m6*t4*t5*t32*4.0-Lx3*Lz6*dQ1*dQ5*m6*t4*t5*t32*2.0-Lx4*Lz6*dQ1*dQ3*m6*t4*t5*t33*4.0-Lx3*Lz6*dQ1*dQ5*m6*t4*t5*t33*2.0-Lx2*Lz6*dQ1*dQ5*m6*t8*t10*t32*2.0+Lx3*Lz6*dQ1*dQ4*m6*t9*t10*t32*2.0+Lx3*Lz6*dQ1*dQ4*m6*t9*t10*t33*2.0+Lx3*Lz6*dQ1*dQ2*m6*t5*t32*t33*8.0+Lx3*Lz6*dQ1*dQ3*m6*t5*t32*t33*8.0;
et71 = Lx4*Lz6*dQ1*dQ5*m6*t5*t32*t34*-2.0-Lx4*Lz6*dQ1*dQ5*m6*t5*t33*t34*2.0-Lx2*Lzcm3*dQ1*dQ2*m3*t2*t7*t8*4.0-Lx2*Lzcm3*dQ1*dQ3*m3*t2*t7*t8*2.0-Lx2*Lzcm4*dQ1*dQ2*m4*t2*t7*t8*4.0-Lx2*Lzcm4*dQ1*dQ3*m4*t2*t7*t8*2.0+Lx2*Lzcm5*dQ4*dQ5*m5*t2*t4*t5*2.0+Lx4*Lzcm5*dQ4*dQ5*m5*t2*t3*t5*2.0+Lx2*Lzcm6*dQ4*dQ5*m6*t2*t4*t5*2.0+Lx4*Lzcm4*dQ1*dQ4*m4*t2*t7*t9*2.0+Lx4*Lzcm6*dQ4*dQ5*m6*t2*t3*t5*2.0+Lx4*Lzcm4*dQ2*dQ3*m4*t2*t8*t9*2.0+Lx4*Lzcm4*dQ2*dQ3*m4*t3*t7*t9*2.0+Lx2*Lzcm5*dQ1*dQ2*m5*t4*t8*t10*2.0+Lx4*Lzcm4*dQ1*dQ4*m4*t3*t8*t9*2.0+Lx3*Lzcm5*dQ1*dQ5*m5*t2*t7*t10*2.0-Lxcm6*Lz6*dQ4*dQ5*m6*t2*t3*t6*2.0+Lx2*Lzcm6*dQ1*dQ2*m6*t4*t8*t10*2.0+Lx3*Lzcm5*dQ1*dQ5*m5*t3*t8*t10*2.0;
et72 = Lx3*Lzcm6*dQ1*dQ5*m6*t2*t7*t10*2.0-Lx4*Lzcm5*dQ2*dQ4*m5*t2*t8*t10*4.0-Lx4*Lzcm5*dQ2*dQ4*m5*t3*t7*t10*4.0-Lx4*Lzcm5*dQ3*dQ4*m5*t2*t8*t10*4.0-Lx4*Lzcm5*dQ3*dQ4*m5*t3*t7*t10*4.0+Lx3*Lzcm6*dQ1*dQ5*m6*t3*t8*t10*2.0-Lx4*Lzcm6*dQ2*dQ4*m6*t2*t8*t10*4.0-Lx4*Lzcm6*dQ2*dQ4*m6*t3*t7*t10*4.0-Lx4*Lzcm5*dQ4*dQ5*m5*t5*t7*t8*2.0-Lx4*Lzcm6*dQ3*dQ4*m6*t2*t8*t10*4.0-Lx4*Lzcm6*dQ3*dQ4*m6*t3*t7*t10*4.0-Lx4*Lzcm6*dQ4*dQ5*m6*t5*t7*t8*2.0-Lxcm6*Lz6*dQ1*dQ2*m6*t5*t9*t11*2.0-Lxcm6*Lz6*dQ1*dQ3*m6*t5*t9*t11*2.0+Lxcm6*Lz6*dQ4*dQ5*m6*t6*t7*t8*2.0-Lxcm6*Lz6*dQ1*dQ6*m6*t5*t10*t11*2.0+Lx2*Lzcm5*dQ1*dQ2*m5*t3*t5*t32*4.0+Lx2*Lzcm5*dQ1*dQ3*m5*t3*t5*t32*2.0;
et73 = Lx2*Lzcm6*dQ1*dQ2*m6*t3*t5*t32*4.0+Lx2*Lzcm6*dQ1*dQ3*m6*t3*t5*t32*2.0-Lx4*Lzcm5*dQ1*dQ2*m5*t4*t5*t32*4.0-Lx4*Lzcm5*dQ1*dQ2*m5*t4*t5*t33*4.0-Lx4*Lzcm5*dQ1*dQ3*m5*t4*t5*t32*4.0-Lx3*Lzcm5*dQ1*dQ5*m5*t4*t5*t32*2.0-Lx4*Lzcm5*dQ1*dQ3*m5*t4*t5*t33*4.0-Lx4*Lzcm6*dQ1*dQ2*m6*t4*t5*t32*4.0-Lx3*Lzcm5*dQ1*dQ5*m5*t4*t5*t33*2.0-Lx4*Lzcm6*dQ1*dQ2*m6*t4*t5*t33*4.0-Lx4*Lzcm6*dQ1*dQ3*m6*t4*t5*t32*4.0-Lx3*Lzcm6*dQ1*dQ5*m6*t4*t5*t32*2.0-Lx4*Lzcm6*dQ1*dQ3*m6*t4*t5*t33*4.0-Lx3*Lzcm6*dQ1*dQ5*m6*t4*t5*t33*2.0+Lxcm6*Lz6*dQ1*dQ2*m6*t4*t6*t32*4.0+Lxcm6*Lz6*dQ1*dQ2*m6*t4*t6*t33*4.0+Lxcm6*Lz6*dQ1*dQ3*m6*t4*t6*t32*4.0+Lxcm6*Lz6*dQ1*dQ3*m6*t4*t6*t33*4.0;
et74 = Lxcm6*Lz6*dQ1*dQ2*m6*t4*t6*t35*4.0+Lxcm6*Lz6*dQ1*dQ3*m6*t4*t6*t35*4.0-Lx2*Lzcm5*dQ1*dQ5*m5*t8*t10*t32*2.0+Lx3*Lzcm5*dQ1*dQ4*m5*t9*t10*t32*2.0-Lx2*Lzcm6*dQ1*dQ5*m6*t8*t10*t32*2.0+Lx3*Lzcm5*dQ1*dQ4*m5*t9*t10*t33*2.0+Lx3*Lzcm6*dQ1*dQ4*m6*t9*t10*t32*2.0+Lx3*Lzcm6*dQ1*dQ4*m6*t9*t10*t33*2.0-Lxcm6*Lz6*dQ1*dQ4*m6*t10*t11*t32*2.0-Lxcm6*Lz6*dQ1*dQ4*m6*t10*t11*t33*2.0+Lx4*Lzcm4*dQ1*dQ2*m4*t4*t32*t33*8.0+Lx4*Lzcm4*dQ1*dQ3*m4*t4*t32*t33*8.0+Lx3*Lzcm5*dQ1*dQ2*m5*t5*t32*t33*8.0+Lx3*Lzcm5*dQ1*dQ3*m5*t5*t32*t33*8.0+Lx3*Lzcm6*dQ1*dQ2*m6*t5*t32*t33*8.0+Lx3*Lzcm6*dQ1*dQ3*m6*t5*t32*t33*8.0-Lx4*Lzcm5*dQ1*dQ5*m5*t5*t32*t34*2.0-Lx4*Lzcm5*dQ1*dQ5*m5*t5*t33*t34*2.0;
et75 = Lx4*Lzcm6*dQ1*dQ5*m6*t5*t32*t34*-2.0-Lx4*Lzcm6*dQ1*dQ5*m6*t5*t33*t34*2.0-Lxcm6*Lz6*dQ1*dQ5*m6*t6*t32*t33*4.0+Lxcm6*Lz6*dQ1*dQ5*m6*t6*t32*t34*2.0-Lxcm6*Lz6*dQ1*dQ5*m6*t6*t32*t35*4.0+Lxcm6*Lz6*dQ1*dQ5*m6*t6*t33*t34*2.0-Lxcm6*Lz6*dQ1*dQ5*m6*t6*t33*t35*4.0+Lxcm4*Lzcm4*dQ1*dQ4*m4*t2*t7*t9*2.0+Lxcm4*Lzcm4*dQ2*dQ3*m4*t2*t8*t9*2.0+Lxcm4*Lzcm4*dQ2*dQ3*m4*t3*t7*t9*2.0+Lxcm4*Lzcm4*dQ1*dQ4*m4*t3*t8*t9*2.0-Lxcm5*Lzcm5*dQ1*dQ4*m5*t2*t7*t9*2.0-Lxcm6*Lzcm6*dQ4*dQ5*m6*t2*t3*t6*2.0-Lxcm5*Lzcm5*dQ2*dQ3*m5*t2*t8*t9*2.0-Lxcm5*Lzcm5*dQ2*dQ3*m5*t3*t7*t9*2.0-Lxcm5*Lzcm5*dQ1*dQ4*m5*t3*t8*t9*2.0-Lxcm6*Lzcm6*dQ1*dQ2*m6*t5*t9*t11*2.0-Lxcm6*Lzcm6*dQ1*dQ3*m6*t5*t9*t11*2.0;
et76 = Lxcm6*Lzcm6*dQ4*dQ5*m6*t6*t7*t8*2.0-Lxcm6*Lzcm6*dQ1*dQ6*m6*t5*t10*t11*2.0+Lxcm6*Lzcm6*dQ1*dQ2*m6*t4*t6*t32*4.0+Lxcm5*Lzcm5*dQ4*dQ5*m5*t2*t3*t35*4.0+Lxcm6*Lzcm6*dQ1*dQ2*m6*t4*t6*t33*4.0+Lxcm6*Lzcm6*dQ1*dQ3*m6*t4*t6*t32*4.0+Lxcm6*Lzcm6*dQ1*dQ3*m6*t4*t6*t33*4.0+Lxcm6*Lzcm6*dQ1*dQ2*m6*t4*t6*t35*4.0+Lxcm6*Lzcm6*dQ1*dQ3*m6*t4*t6*t35*4.0-Lxcm5*Lzcm5*dQ4*dQ5*m5*t7*t8*t35*4.0-Lxcm6*Lzcm6*dQ1*dQ4*m6*t10*t11*t32*2.0-Lxcm6*Lzcm6*dQ1*dQ4*m6*t10*t11*t33*2.0+Lxcm4*Lzcm4*dQ1*dQ2*m4*t4*t32*t33*8.0+Lxcm4*Lzcm4*dQ1*dQ3*m4*t4*t32*t33*8.0-Lxcm5*Lzcm5*dQ1*dQ2*m5*t4*t32*t33*8.0-Lxcm5*Lzcm5*dQ1*dQ3*m5*t4*t32*t33*8.0-Lxcm5*Lzcm5*dQ1*dQ2*m5*t4*t32*t35*8.0-Lxcm5*Lzcm5*dQ1*dQ2*m5*t4*t33*t35*8.0;
et77 = Lxcm5*Lzcm5*dQ1*dQ3*m5*t4*t32*t35*-8.0-Lxcm5*Lzcm5*dQ1*dQ3*m5*t4*t33*t35*8.0-Lxcm6*Lzcm6*dQ1*dQ5*m6*t6*t32*t33*4.0+Lxcm6*Lzcm6*dQ1*dQ5*m6*t6*t32*t34*2.0-Lxcm6*Lzcm6*dQ1*dQ5*m6*t6*t32*t35*4.0+Lxcm6*Lzcm6*dQ1*dQ5*m6*t6*t33*t34*2.0-Lxcm6*Lzcm6*dQ1*dQ5*m6*t6*t33*t35*4.0-Lxcm5*Lzcm5*dQ1*dQ5*m5*t32*t33*t34*4.0+Lxcm5*Lzcm5*dQ1*dQ5*m5*t32*t33*t35*8.0-Lxcm5*Lzcm5*dQ1*dQ5*m5*t32*t34*t35*4.0-Lxcm5*Lzcm5*dQ1*dQ5*m5*t33*t34*t35*4.0-Lycm6*Lz6*dQ1*dQ2*m6*t5*t6*t9*2.0-Lycm6*Lz6*dQ1*dQ3*m6*t5*t6*t9*2.0+Lycm6*Lz6*dQ4*dQ5*m6*t2*t3*t11*2.0-Lycm6*Lz6*dQ1*dQ6*m6*t5*t6*t10*2.0-Lycm6*Lz6*dQ4*dQ5*m6*t7*t8*t11*2.0-Lycm6*Lz6*dQ1*dQ2*m6*t4*t11*t32*4.0-Lycm6*Lz6*dQ1*dQ2*m6*t4*t11*t33*4.0;
et78 = Lycm6*Lz6*dQ1*dQ3*m6*t4*t11*t32*-4.0-Lycm6*Lz6*dQ1*dQ3*m6*t4*t11*t33*4.0-Lycm6*Lz6*dQ1*dQ2*m6*t4*t11*t35*4.0-Lycm6*Lz6*dQ1*dQ4*m6*t6*t10*t32*2.0-Lycm6*Lz6*dQ1*dQ3*m6*t4*t11*t35*4.0-Lycm6*Lz6*dQ1*dQ4*m6*t6*t10*t33*2.0+Lycm6*Lz6*dQ1*dQ5*m6*t11*t32*t33*4.0-Lycm6*Lz6*dQ1*dQ5*m6*t11*t32*t34*2.0+Lycm6*Lz6*dQ1*dQ5*m6*t11*t32*t35*4.0-Lycm6*Lz6*dQ1*dQ5*m6*t11*t33*t34*2.0+Lycm6*Lz6*dQ1*dQ5*m6*t11*t33*t35*4.0+Lycm4*Lzcm4*dQ1*dQ4*m4*t2*t4*t7*2.0+Lycm4*Lzcm4*dQ2*dQ3*m4*t2*t4*t8*2.0+Lycm4*Lzcm4*dQ2*dQ3*m4*t3*t4*t7*2.0+Lycm4*Lzcm4*dQ1*dQ4*m4*t3*t4*t8*2.0-Lycm5*Lzcm5*dQ2*dQ3*m5*t2*t3*t10*2.0-Lycm6*Lzcm6*dQ1*dQ2*m6*t5*t6*t9*2.0-Lycm6*Lzcm6*dQ1*dQ3*m6*t5*t6*t9*2.0;
et79 = Lycm6*Lzcm6*dQ4*dQ5*m6*t2*t3*t11*2.0+Lycm5*Lzcm5*dQ2*dQ3*m5*t7*t8*t10*2.0-Lycm6*Lzcm6*dQ1*dQ6*m6*t5*t6*t10*2.0-Lycm6*Lzcm6*dQ4*dQ5*m6*t7*t8*t11*2.0+Lycm5*Lzcm5*dQ1*dQ2*m5*t5*t9*t32*4.0+Lycm5*Lzcm5*dQ1*dQ2*m5*t5*t9*t33*4.0+Lycm5*Lzcm5*dQ1*dQ3*m5*t5*t9*t32*4.0+Lycm5*Lzcm5*dQ1*dQ3*m5*t5*t9*t33*4.0-Lycm6*Lzcm6*dQ1*dQ2*m6*t4*t11*t32*4.0-Lycm6*Lzcm6*dQ1*dQ2*m6*t4*t11*t33*4.0-Lycm6*Lzcm6*dQ1*dQ3*m6*t4*t11*t32*4.0-Lycm6*Lzcm6*dQ1*dQ3*m6*t4*t11*t33*4.0-Lycm6*Lzcm6*dQ1*dQ2*m6*t4*t11*t35*4.0-Lycm6*Lzcm6*dQ1*dQ4*m6*t6*t10*t32*2.0-Lycm6*Lzcm6*dQ1*dQ3*m6*t4*t11*t35*4.0-Lycm6*Lzcm6*dQ1*dQ4*m6*t6*t10*t33*2.0-Lycm4*Lzcm4*dQ1*dQ2*m4*t9*t32*t33*8.0-Lycm4*Lzcm4*dQ1*dQ3*m4*t9*t32*t33*8.0;
et80 = Lycm5*Lzcm5*dQ1*dQ4*m5*t10*t32*t33*4.0+Lycm5*Lzcm5*dQ1*dQ4*m5*t10*t32*t34*4.0+Lycm5*Lzcm5*dQ1*dQ4*m5*t10*t33*t34*4.0+Lycm6*Lzcm6*dQ1*dQ5*m6*t11*t32*t33*4.0-Lycm6*Lzcm6*dQ1*dQ5*m6*t11*t32*t34*2.0+Lycm6*Lzcm6*dQ1*dQ5*m6*t11*t32*t35*4.0-Lycm6*Lzcm6*dQ1*dQ5*m6*t11*t33*t34*2.0+Lycm6*Lzcm6*dQ1*dQ5*m6*t11*t33*t35*4.0+Lz6*Lzcm6*dQ1*dQ5*m6*t2*t4*t7*4.0+Lz6*Lzcm6*dQ1*dQ5*m6*t3*t4*t8*4.0+Lz6*Lzcm6*dQ2*dQ5*m6*t2*t3*t9*4.0+Lz6*Lzcm6*dQ1*dQ2*m6*t4*t5*t10*4.0+Lz6*Lzcm6*dQ3*dQ5*m6*t2*t3*t9*4.0+Lz6*Lzcm6*dQ1*dQ3*m6*t4*t5*t10*4.0-Lz6*Lzcm6*dQ2*dQ5*m6*t7*t8*t9*4.0-Lz6*Lzcm6*dQ3*dQ5*m6*t7*t8*t9*4.0+Lz6*Lzcm6*dQ1*dQ2*m6*t2*t7*t34*4.0-Lz6*Lzcm6*dQ1*dQ2*m6*t2*t7*t35*4.0+Lz6*Lzcm6*dQ1*dQ3*m6*t2*t7*t34*4.0;
et81 = Lz6*Lzcm6*dQ1*dQ2*m6*t3*t8*t34*4.0-Lz6*Lzcm6*dQ1*dQ3*m6*t2*t7*t35*4.0-Lz6*Lzcm6*dQ1*dQ2*m6*t3*t8*t35*4.0+Lz6*Lzcm6*dQ1*dQ3*m6*t3*t8*t34*4.0-Lz6*Lzcm6*dQ1*dQ3*m6*t3*t8*t35*4.0+Lz6*Lzcm6*dQ1*dQ4*m6*t4*t9*t32*4.0+Lz6*Lzcm6*dQ2*dQ4*m6*t2*t8*t34*4.0+Lz6*Lzcm6*dQ2*dQ4*m6*t3*t7*t34*4.0+Lz6*Lzcm6*dQ1*dQ4*m6*t4*t9*t33*4.0+Lz6*Lzcm6*dQ2*dQ4*m6*t2*t8*t35*4.0+Lz6*Lzcm6*dQ2*dQ4*m6*t3*t7*t35*4.0+Lz6*Lzcm6*dQ3*dQ4*m6*t2*t8*t34*4.0+Lz6*Lzcm6*dQ3*dQ4*m6*t3*t7*t34*4.0+Lz6*Lzcm6*dQ3*dQ4*m6*t2*t8*t35*4.0+Lz6*Lzcm6*dQ3*dQ4*m6*t3*t7*t35*4.0-Lz6*Lzcm6*dQ1*dQ5*m6*t5*t10*t32*4.0-Lz6*Lzcm6*dQ1*dQ5*m6*t5*t10*t33*4.0+Ixx6*dQ2*dQ3*t2*t3*t5*t6*t11*2.0+Ixx5*dQ1*dQ4*t2*t5*t7*t9*t10*2.0;
et82 = Ixx5*dQ2*dQ3*t2*t5*t8*t9*t10*2.0+Ixx5*dQ2*dQ3*t3*t5*t7*t9*t10*2.0+Ixx5*dQ1*dQ4*t3*t5*t8*t9*t10*2.0-Ixx6*dQ2*dQ3*t5*t6*t7*t8*t11*2.0+Ixx6*dQ5*dQ6*t2*t6*t8*t9*t11*2.0+Ixx6*dQ5*dQ6*t3*t6*t7*t9*t11*2.0-Ixx5*dQ2*dQ3*t2*t3*t4*t9*t35*2.0-Ixx6*dQ2*dQ3*t2*t3*t4*t9*t36*2.0-Ixx6*dQ2*dQ6*t2*t3*t4*t10*t36*2.0-Ixx6*dQ3*dQ6*t2*t3*t4*t10*t36*2.0+Ixx6*dQ4*dQ5*t2*t3*t5*t10*t36*2.0-Ixx6*dQ5*dQ6*t2*t4*t5*t8*t36*2.0-Ixx6*dQ5*dQ6*t3*t4*t5*t7*t36*2.0+Ixx5*dQ2*dQ3*t4*t7*t8*t9*t35*2.0+Ixx6*dQ4*dQ6*t2*t3*t6*t11*t35*2.0+Ixx6*dQ1*dQ6*t2*t7*t9*t10*t33*4.0+Ixx6*dQ1*dQ6*t3*t8*t9*t10*t32*4.0+Ixx6*dQ2*dQ3*t4*t7*t8*t9*t36*2.0+Ixx6*dQ1*dQ2*t6*t9*t10*t11*t32*4.0;
et83 = Ixx6*dQ1*dQ6*t2*t7*t9*t10*t36*4.0+Ixx6*dQ1*dQ2*t6*t9*t10*t11*t33*4.0+Ixx6*dQ1*dQ3*t6*t9*t10*t11*t32*4.0+Ixx6*dQ1*dQ3*t6*t9*t10*t11*t33*4.0+Ixx6*dQ1*dQ6*t3*t8*t9*t10*t36*4.0+Ixx6*dQ2*dQ6*t4*t7*t8*t10*t36*2.0+Ixx6*dQ3*dQ6*t4*t7*t8*t10*t36*2.0-Ixx6*dQ4*dQ5*t5*t7*t8*t10*t36*2.0-Ixx6*dQ4*dQ6*t2*t8*t9*t10*t36*2.0-Ixx6*dQ4*dQ6*t3*t7*t9*t10*t36*2.0-Ixx6*dQ4*dQ6*t6*t7*t8*t11*t35*2.0+Ixx5*dQ1*dQ2*t4*t5*t10*t32*t33*8.0+Ixx5*dQ1*dQ5*t2*t4*t7*t33*t35*8.0+Ixx5*dQ1*dQ3*t4*t5*t10*t32*t33*8.0+Ixx5*dQ1*dQ5*t3*t4*t8*t32*t35*8.0-Ixx6*dQ1*dQ5*t2*t4*t7*t33*t36*4.0-Ixx6*dQ1*dQ5*t3*t4*t8*t32*t36*4.0-Ixx6*dQ1*dQ2*t4*t5*t10*t32*t36*4.0;
et84 = Ixx6*dQ1*dQ5*t2*t4*t7*t35*t36*-4.0-Ixx6*dQ1*dQ6*t4*t5*t9*t32*t33*4.0-Ixx6*dQ1*dQ2*t4*t5*t10*t33*t36*4.0-Ixx6*dQ1*dQ3*t4*t5*t10*t32*t36*4.0-Ixx6*dQ1*dQ3*t4*t5*t10*t33*t36*4.0-Ixx6*dQ1*dQ4*t5*t6*t11*t32*t33*4.0-Ixx6*dQ1*dQ5*t3*t4*t8*t35*t36*4.0-Ixx6*dQ2*dQ5*t2*t3*t9*t35*t36*2.0-Ixx6*dQ1*dQ4*t5*t6*t11*t32*t34*4.0-Ixx6*dQ1*dQ6*t4*t5*t9*t32*t36*4.0-Ixx6*dQ2*dQ6*t2*t5*t8*t34*t36*4.0-Ixx6*dQ2*dQ6*t3*t5*t7*t34*t36*4.0-Ixx6*dQ3*dQ5*t2*t3*t9*t35*t36*2.0-Ixx6*dQ1*dQ4*t5*t6*t11*t33*t34*4.0-Ixx6*dQ1*dQ6*t4*t5*t9*t33*t36*4.0-Ixx6*dQ3*dQ6*t2*t5*t8*t34*t36*4.0-Ixx6*dQ3*dQ6*t3*t5*t7*t34*t36*4.0+Ixx6*dQ4*dQ5*t2*t4*t8*t35*t36*2.0;
et85 = Ixx6*dQ4*dQ5*t3*t4*t7*t35*t36*2.0+Ixx6*dQ2*dQ5*t7*t8*t9*t35*t36*2.0+Ixx6*dQ3*dQ5*t7*t8*t9*t35*t36*2.0+Ixx5*dQ1*dQ2*t2*t7*t33*t34*t35*4.0+Ixx5*dQ1*dQ2*t3*t8*t32*t34*t35*4.0+Ixx5*dQ1*dQ3*t2*t7*t33*t34*t35*4.0+Ixx5*dQ1*dQ3*t3*t8*t32*t34*t35*4.0+Ixx6*dQ1*dQ2*t2*t7*t33*t34*t36*4.0+Ixx6*dQ1*dQ2*t2*t7*t33*t35*t36*4.0+Ixx6*dQ1*dQ2*t3*t8*t32*t34*t36*4.0+Ixx6*dQ1*dQ3*t2*t7*t33*t34*t36*4.0+Ixx5*dQ1*dQ4*t4*t9*t32*t33*t35*4.0-Ixx6*dQ1*dQ2*t2*t7*t34*t35*t36*2.0+Ixx6*dQ1*dQ2*t3*t8*t32*t35*t36*4.0+Ixx6*dQ1*dQ3*t2*t7*t33*t35*t36*4.0+Ixx6*dQ1*dQ3*t3*t8*t32*t34*t36*4.0-Ixx6*dQ1*dQ3*t2*t7*t34*t35*t36*2.0+Ixx6*dQ1*dQ3*t3*t8*t32*t35*t36*4.0+Ixx5*dQ1*dQ5*t5*t10*t32*t33*t34*4.0;
et86 = Ixx6*dQ1*dQ2*t3*t8*t34*t35*t36*-2.0+Ixx6*dQ1*dQ4*t4*t9*t32*t33*t36*4.0-Ixx6*dQ1*dQ3*t3*t8*t34*t35*t36*2.0-Ixx6*dQ1*dQ4*t4*t9*t32*t35*t36*2.0-Ixx6*dQ2*dQ4*t2*t8*t34*t35*t36*2.0-Ixx6*dQ2*dQ4*t3*t7*t34*t35*t36*2.0-Ixx6*dQ1*dQ4*t4*t9*t33*t35*t36*2.0+Ixx6*dQ1*dQ5*t5*t10*t32*t33*t36*4.0-Ixx6*dQ3*dQ4*t2*t8*t34*t35*t36*2.0-Ixx6*dQ3*dQ4*t3*t7*t34*t35*t36*2.0-Ixx6*dQ1*dQ5*t5*t10*t32*t34*t36*2.0+Ixx6*dQ1*dQ6*t6*t11*t32*t33*t34*4.0-Ixx6*dQ1*dQ5*t5*t10*t33*t34*t36*2.0+Ixx6*dQ1*dQ6*t6*t11*t32*t33*t35*4.0-Ixx6*dQ1*dQ6*t6*t11*t32*t34*t35*2.0-Ixx6*dQ1*dQ6*t6*t11*t33*t34*t35*2.0-Iyy6*dQ2*dQ3*t2*t3*t5*t6*t11*2.0+Iyy6*dQ1*dQ4*t2*t5*t7*t9*t10*2.0;
et87 = Iyy6*dQ2*dQ3*t2*t5*t8*t9*t10*2.0+Iyy6*dQ2*dQ3*t3*t5*t7*t9*t10*2.0+Iyy6*dQ1*dQ4*t3*t5*t8*t9*t10*2.0+Iyy6*dQ2*dQ3*t5*t6*t7*t8*t11*2.0-Iyy6*dQ5*dQ6*t2*t6*t8*t9*t11*2.0-Iyy6*dQ5*dQ6*t3*t6*t7*t9*t11*2.0-Iyy6*dQ2*dQ3*t2*t3*t4*t9*t35*2.0+Iyy6*dQ2*dQ3*t2*t3*t4*t9*t36*2.0+Iyy6*dQ2*dQ6*t2*t3*t4*t10*t36*2.0+Iyy6*dQ3*dQ6*t2*t3*t4*t10*t36*2.0-Iyy6*dQ4*dQ5*t2*t3*t5*t10*t36*2.0+Iyy6*dQ5*dQ6*t2*t4*t5*t8*t36*2.0+Iyy6*dQ5*dQ6*t3*t4*t5*t7*t36*2.0-Iyy6*dQ4*dQ6*t2*t3*t6*t11*t35*2.0-Iyy6*dQ1*dQ6*t2*t7*t9*t10*t33*4.0+Iyy6*dQ2*dQ3*t4*t7*t8*t9*t35*2.0-Iyy6*dQ1*dQ6*t3*t8*t9*t10*t32*4.0-Iyy6*dQ2*dQ3*t4*t7*t8*t9*t36*2.0-Iyy6*dQ1*dQ2*t6*t9*t10*t11*t32*4.0;
et88 = Iyy6*dQ1*dQ6*t2*t7*t9*t10*t36*-4.0-Iyy6*dQ1*dQ2*t6*t9*t10*t11*t33*4.0-Iyy6*dQ1*dQ3*t6*t9*t10*t11*t32*4.0-Iyy6*dQ1*dQ3*t6*t9*t10*t11*t33*4.0-Iyy6*dQ1*dQ6*t3*t8*t9*t10*t36*4.0-Iyy6*dQ2*dQ6*t4*t7*t8*t10*t36*2.0-Iyy6*dQ3*dQ6*t4*t7*t8*t10*t36*2.0+Iyy6*dQ4*dQ5*t5*t7*t8*t10*t36*2.0+Iyy6*dQ4*dQ6*t2*t8*t9*t10*t36*2.0+Iyy6*dQ4*dQ6*t3*t7*t9*t10*t36*2.0+Iyy6*dQ4*dQ6*t6*t7*t8*t11*t35*2.0+Iyy6*dQ1*dQ2*t4*t5*t10*t32*t33*8.0+Iyy6*dQ1*dQ5*t2*t4*t7*t33*t35*8.0+Iyy6*dQ1*dQ3*t4*t5*t10*t32*t33*8.0+Iyy6*dQ1*dQ5*t2*t4*t7*t33*t36*4.0+Iyy6*dQ1*dQ5*t3*t4*t8*t32*t35*8.0+Iyy6*dQ1*dQ5*t3*t4*t8*t32*t36*4.0+Iyy6*dQ1*dQ2*t4*t5*t10*t32*t36*4.0;
